simulink model "cubli_XYZ_extensive_simulations"  (R2016a)
settings: Solver=VariableStepAuto  StartTime=0.0  StopTime=10  FixedStep=0.001  RelTol=1e-3
values from neighbouring files (symbols this model uses):
  a = 0.15    [init.m]
  M = 2.5    [init.m]    (also in skew.m = [0 -z y)
  m = 0.204    [init.m]
  s = size(delta_i)    [accessibility_test.m]    (also in observability_test.m = size(delta_i,1))
  state0 = get_equilibrium(0, -pi/4, pi/2, f, state)    [init.m]
undefined symbols (not defined in the file or in its folder): X, Y, Z
libraries: sm_lib x15, nesl_utility x13
(part 3 of 9)

== matlab function cubli_XYZ_extensive_simulations/Cubli/Reference/Slerp ==
  data: R0 input; Rf input; t input; theta_des output; theta input; dtheta_des output; ddtheta_des output
function [theta_des, dtheta_des, ddtheta_des]    = slerp(R0, Rf, t, theta)

% persistent counter th0 thf R0 Rf

% if isempty(counter)
%     counter = 0;
%     R0 = rotx(state0(1))*roty(state0(2))*rotz(state0(3));
%     Rf = rotz(theta) * R0;
%     th0 = [state0(1);state0(2);state0(3)];
%     th21 = atan2(Rf(1,3), sqrt(Rf(2,3)^2 + Rf(3,3)^2));
%     thf = [atan2(-Rf(2,3) / cos(th21), Rf(3,3) / cos(th21));
%            th21;
%            atan2(-Rf(1,2) / cos(th21), Rf(1,1) / cos(th21))];
% end
% t = time/tf;
% 
% if time >= tf
%     t = 1;
% end

% t = time - tf * counter;
% t = time / tf - counter;
% if t > 1
%     counter = counter + 1;
%     t = time/tf - counter;
%     tmp = thf;
%     thf = th0;
%     th0 = tmp;
%     tmp = Rf;
%     Rf = R0;
%     R0 = tmp;
% 
% end

% traj_5_const = 6.0;
% traj_4_const = -15.0;
% traj_3_const = 10.0;
% 
% theta_des = zeros(3,1);
% dtheta_des = zeros(3,1);
% ddtheta_des = zeros(3,1);

% for i = 1:3
%     traj_0_coeff = th0(i);
%     traj_3_coeff = traj_3_const / (tf ^3) * (thf(i) - th0(i));
%     traj_4_coeff = traj_4_const / (tf ^4) * (thf(i) - th0(i));
%     traj_5_coeff = traj_5_const / (tf ^5) * (thf(i) - th0(i));
%     theta_des(i) = traj_5_coeff * t^5 + traj_4_coeff * t^4 + traj_3_coeff * t^3 + traj_0_coeff;
%     dtheta_des(i) = 5 * traj_5_coeff * t^4 + 4 * traj_4_coeff * t^3 + 3 * traj_3_coeff * t^2;
%     ddtheta_des(i) = 5 * 4 * traj_5_coeff * t^3 + 4 * 3 * traj_4_coeff * t^2 + 3 * 2 * traj_3_coeff * t;
% end

q0 = rotm2quat(R0);
q1 = rotm2quat(Rf);

q01 = q0(1);
q02 = q0(2);
q03 = q0(3);
q04 = q0(4);

q11 = q1(1);
q12 = q1(2);
q13 = q1(3);
q14 = q1(4);

th1_des = atan2(2.*csc((1/2).*theta).^2.*((q01.*q02+(-1).* ...
  q03.*q04).*sin((1/2).*(1+(-1).*t).*theta).^2+(q02.*q11+q01.*q12+(-1).* ...
  q04.*q13+(-1).*q03.*q14).*sin((1/2).*(1+(-1).*t).*theta).*sin((1/2).*t.* ...
  theta)+(q11.*q12+(-1).*q13.*q14).*sin((1/2).*t.*theta).^2).*(4.*csc(( ...
  1/2).*theta).^4.*(((-1).*q01.*q02+q03.*q04).*sin((1/2).*(1+(-1).*t).* ...
  theta).^2+(-1).*(q02.*q11+q01.*q12+(-1).*q04.*q13+(-1).*q03.*q14).*sin(( ...
  1/2).*(1+(-1).*t).*theta).*sin((1/2).*t.*theta)+((-1).*q11.*q12+q13.* ...
  q14).*sin((1/2).*t.*theta).^2).^2+(1+(-2).*csc((1/2).*theta).^2.*((q02.* ...
  sin((1/2).*(1+(-1).*t).*theta)+q12.*sin((1/2).*t.*theta)).^2+(q03.*sin(( ...
  1/2).*(1+(-1).*t).*theta)+q13.*sin((1/2).*t.*theta)).^2)).^2).^(-1/2).*( ...
  4.*csc((1/2).*theta).^4.*((q01.*q03+q02.*q04).*sin((1/2).*(1+(-1).*t).* ...
  theta).^2+(q03.*q11+q04.*q12+q01.*q13+q02.*q14).*sin((1/2).*(1+(-1).*t) ...
  .*theta).*sin((1/2).*t.*theta)+(q11.*q13+q12.*q14).*sin((1/2).*t.*theta) ...
  .^2).^2+4.*csc((1/2).*theta).^4.*(((-1).*q01.*q02+q03.*q04).*sin((1/2).* ...
  (1+(-1).*t).*theta).^2+(-1).*(q02.*q11+q01.*q12+(-1).*q04.*q13+(-1).* ...
  q03.*q14).*sin((1/2).*(1+(-1).*t).*theta).*sin((1/2).*t.*theta)+((-1).* ...
  q11.*q12+q13.*q14).*sin((1/2).*t.*theta).^2).^2+(1+(-2).*csc((1/2).* ...
  theta).^2.*((q02.*sin((1/2).*(1+(-1).*t).*theta)+q12.*sin((1/2).*t.* ...
  theta)).^2+(q03.*sin((1/2).*(1+(-1).*t).*theta)+q13.*sin((1/2).*t.* ...
  theta)).^2)).^2).^(1/2),...
  (1+(-2).*csc((1/2).*theta).^2.*((q02.^2+q03.^2).*sin((1/2).*(1+(-1) ...
  .*t).*theta).^2+2.*(q02.*q12+q03.*q13).*sin((1/2).*(1+(-1).*t).*theta).* ...
  sin((1/2).*t.*theta)+(q12.^2+q13.^2).*sin((1/2).*t.*theta).^2)).*(4.* ...
  csc((1/2).*theta).^4.*(((-1).*q01.*q02+q03.*q04).*sin((1/2).*(1+(-1).*t) ...
  .*theta).^2+(-1).*(q02.*q11+q01.*q12+(-1).*q04.*q13+(-1).*q03.*q14).* ...
  sin((1/2).*(1+(-1).*t).*theta).*sin((1/2).*t.*theta)+((-1).*q11.*q12+ ...
  q13.*q14).*sin((1/2).*t.*theta).^2).^2+(1+(-2).*csc((1/2).*theta).^2.*(( ...
  q02.*sin((1/2).*(1+(-1).*t).*theta)+q12.*sin((1/2).*t.*theta)).^2+(q03.* ...
  sin((1/2).*(1+(-1).*t).*theta)+q13.*sin((1/2).*t.*theta)).^2)).^2).^( ...
  -1/2).*(4.*csc((1/2).*theta).^4.*((q01.*q03+q02.*q04).*sin((1/2).*(1+( ...
  -1).*t).*theta).^2+(q03.*q11+q04.*q12+q01.*q13+q02.*q14).*sin((1/2).*(1+ ...
  (-1).*t).*theta).*sin((1/2).*t.*theta)+(q11.*q13+q12.*q14).*sin((1/2).* ...
  t.*theta).^2).^2+4.*csc((1/2).*theta).^4.*(((-1).*q01.*q02+q03.*q04).* ...
  sin((1/2).*(1+(-1).*t).*theta).^2+(-1).*(q02.*q11+q01.*q12+(-1).*q04.* ...
  q13+(-1).*q03.*q14).*sin((1/2).*(1+(-1).*t).*theta).*sin((1/2).*t.* ...
  theta)+((-1).*q11.*q12+q13.*q14).*sin((1/2).*t.*theta).^2).^2+(1+(-2).* ...
  csc((1/2).*theta).^2.*((q02.*sin((1/2).*(1+(-1).*t).*theta)+q12.*sin(( ...
  1/2).*t.*theta)).^2+(q03.*sin((1/2).*(1+(-1).*t).*theta)+q13.*sin((1/2) ...
  .*t.*theta)).^2)).^2).^(1/2));

th2_des = atan2(2.*csc((1/2).*theta).^2.*((q01.*q03+q02.*q04).* ...
  sin((1/2).*(1+(-1).*t).*theta).^2+(q03.*q11+q04.*q12+q01.*q13+q02.*q14) ...
  .*sin((1/2).*(1+(-1).*t).*theta).*sin((1/2).*t.*theta)+(q11.*q13+q12.* ...
  q14).*sin((1/2).*t.*theta).^2),...
 (4.*csc((1/2).*theta).^4.*(((-1).*q01.*q02+q03.*q04).*sin((1/2).*( ...
  1+(-1).*t).*theta).^2+(-1).*(q02.*q11+q01.*q12+(-1).*q04.*q13+(-1).* ...
  q03.*q14).*sin((1/2).*(1+(-1).*t).*theta).*sin((1/2).*t.*theta)+((-1).* ...
  q11.*q12+q13.*q14).*sin((1/2).*t.*theta).^2).^2+(1+(-2).*csc((1/2).* ...
  theta).^2.*((q02.*sin((1/2).*(1+(-1).*t).*theta)+q12.*sin((1/2).*t.* ...
  theta)).^2+(q03.*sin((1/2).*(1+(-1).*t).*theta)+q13.*sin((1/2).*t.* ...
  theta)).^2)).^2).^(1/2));

th3_des = atan2((-2).*csc((1/2).*theta).^2.*((q02.*q03+(-1) ...
  .*q01.*q04).*sin((1/2).*(1+(-1).*t).*theta).^2+(-1).*(q04.*q11+(-1).* ...
  q03.*q12+(-1).*q02.*q13+q01.*q14).*sin((1/2).*(1+(-1).*t).*theta).*sin(( ...
  1/2).*t.*theta)+(q12.*q13+(-1).*q11.*q14).*sin((1/2).*t.*theta).^2).*( ...
  4.*csc((1/2).*theta).^4.*(((-1).*q01.*q02+q03.*q04).*sin((1/2).*(1+(-1) ...
  .*t).*theta).^2+(-1).*(q02.*q11+q01.*q12+(-1).*q04.*q13+(-1).*q03.*q14) ...
  .*sin((1/2).*(1+(-1).*t).*theta).*sin((1/2).*t.*theta)+((-1).*q11.*q12+ ...
  q13.*q14).*sin((1/2).*t.*theta).^2).^2+(1+(-2).*csc((1/2).*theta).^2.*(( ...
  q02.*sin((1/2).*(1+(-1).*t).*theta)+q12.*sin((1/2).*t.*theta)).^2+(q03.* ...
  sin((1/2).*(1+(-1).*t).*theta)+q13.*sin((1/2).*t.*theta)).^2)).^2).^( ...
  -1/2).*(4.*csc((1/2).*theta).^4.*((q01.*q03+q02.*q04).*sin((1/2).*(1+( ...
  -1).*t).*theta).^2+(q03.*q11+q04.*q12+q01.*q13+q02.*q14).*sin((1/2).*(1+ ...
  (-1).*t).*theta).*sin((1/2).*t.*theta)+(q11.*q13+q12.*q14).*sin((1/2).* ...
  t.*theta).^2).^2+4.*csc((1/2).*theta).^4.*(((-1).*q01.*q02+q03.*q04).* ...
  sin((1/2).*(1+(-1).*t).*theta).^2+(-1).*(q02.*q11+q01.*q12+(-1).*q04.* ...
  q13+(-1).*q03.*q14).*sin((1/2).*(1+(-1).*t).*theta).*sin((1/2).*t.* ...
  theta)+((-1).*q11.*q12+q13.*q14).*sin((1/2).*t.*theta).^2).^2+(1+(-2).* ...
  csc((1/2).*theta).^2.*((q02.*sin((1/2).*(1+(-1).*t).*theta)+q12.*sin(( ...
  1/2).*t.*theta)).^2+(q03.*sin((1/2).*(1+(-1).*t).*theta)+q13.*sin((1/2) ...
  .*t.*theta)).^2)).^2).^(1/2),...
  (1+(-2).*csc((1/2).*theta).^2.*((q03.^2+q04.^2).*sin((1/2).*(1+(-1) ...
  .*t).*theta).^2+2.*(q03.*q13+q04.*q14).*sin((1/2).*(1+(-1).*t).*theta).* ...
  sin((1/2).*t.*theta)+(q13.^2+q14.^2).*sin((1/2).*t.*theta).^2)).*(4.* ...
  csc((1/2).*theta).^4.*(((-1).*q01.*q02+q03.*q04).*sin((1/2).*(1+(-1).*t) ...
  .*theta).^2+(-1).*(q02.*q11+q01.*q12+(-1).*q04.*q13+(-1).*q03.*q14).* ...
  sin((1/2).*(1+(-1).*t).*theta).*sin((1/2).*t.*theta)+((-1).*q11.*q12+ ...
  q13.*q14).*sin((1/2).*t.*theta).^2).^2+(1+(-2).*csc((1/2).*theta).^2.*(( ...
  q02.*sin((1/2).*(1+(-1).*t).*theta)+q12.*sin((1/2).*t.*theta)).^2+(q03.* ...
  sin((1/2).*(1+(-1).*t).*theta)+q13.*sin((1/2).*t.*theta)).^2)).^2).^( ...
  -1/2).*(4.*csc((1/2).*theta).^4.*((q01.*q03+q02.*q04).*sin((1/2).*(1+( ...
  -1).*t).*theta).^2+(q03.*q11+q04.*q12+q01.*q13+q02.*q14).*sin((1/2).*(1+ ...
  (-1).*t).*theta).*sin((1/2).*t.*theta)+(q11.*q13+q12.*q14).*sin((1/2).* ...
  t.*theta).^2).^2+4.*csc((1/2).*theta).^4.*(((-1).*q01.*q02+q03.*q04).* ...
  sin((1/2).*(1+(-1).*t).*theta).^2+(-1).*(q02.*q11+q01.*q12+(-1).*q04.* ...
  q13+(-1).*q03.*q14).*sin((1/2).*(1+(-1).*t).*theta).*sin((1/2).*t.* ...
  theta)+((-1).*q11.*q12+q13.*q14).*sin((1/2).*t.*theta).^2).^2+(1+(-2).* ...
  csc((1/2).*theta).^2.*((q02.*sin((1/2).*(1+(-1).*t).*theta)+q12.*sin(( ...
  1/2).*t.*theta)).^2+(q03.*sin((1/2).*(1+(-1).*t).*theta)+q13.*sin((1/2) ...
  .*t.*theta)).^2)).^2).^(1/2));

theta_des = [th1_des; th2_des; th3_des];

dth1_des = (1/4).*theta.*csc((1/2).*theta).^4.*(1+(-4).*csc((1/2).*theta).^2.*(( ...
  q02.^2+q03.^2).*sin((1/2).*(1+(-1).*t).*theta).^2+2.*(q02.*q12+q03.*q13) ...
  .*sin((1/2).*(1+(-1).*t).*theta).*sin((1/2).*t.*theta)+(q12.^2+q13.^2).* ...
  sin((1/2).*t.*theta).^2)+4.*csc((1/2).*theta).^4.*((q01.^2.*q02.^2+ ...
  q02.^4+2.*q02.^2.*q03.^2+q03.^4+(-2).*q01.*q02.*q03.*q04+q03.^2.*q04.^2) ...
  .*sin((1/2).*(1+(-1).*t).*theta).^4+2.*(q01.^2.*q02.*q12+2.*q02.^3.*q12+ ...
  q02.*q03.*((-1).*q04.*q11+2.*q03.*q12)+2.*q02.^2.*q03.*q13+q03.*(2.* ...
  q03.^2.*q13+q04.^2.*q13+q03.*q04.*q14)+q01.*(q02.^2.*q11+(-1).*q03.* ...
  q04.*q12+(-1).*q02.*(q04.*q13+q03.*q14))).*sin((1/2).*(1+(-1).*t).* ...
  theta).^3.*sin((1/2).*t.*theta)+((q01.*q12+(-1).*q04.*q13).^2+q02.^2.*( ...
  q11.^2+6.*q12.^2+2.*q13.^2)+q02.*(4.*q01.*q11.*q12+(-2).*q04.*q11.*q13+ ...
  8.*q03.*q12.*q13+(-2).*q03.*q11.*q14+(-2).*q01.*q13.*q14)+(-2).*q03.*( ...
  q04.*q11.*q12+q01.*q12.*q14+(-2).*q04.*q13.*q14)+q03.^2.*(2.*q12.^2+6.* ...
  q13.^2+q14.^2)).*sin((1/2).*(1+(-1).*t).*theta).^2.*sin((1/2).*t.*theta) ...
  .^2+2.*((-1).*q04.*q11.*q12.*q13+2.*q03.*q12.^2.*q13+2.*q03.*q13.^3+(-1) ...
  .*q03.*q11.*q12.*q14+q04.*q13.^2.*q14+q03.*q13.*q14.^2+q01.*q12.*(q11.* ...
  q12+(-1).*q13.*q14)+q02.*(q11.^2.*q12+2.*q12.*(q12.^2+q13.^2)+(-1).* ...
  q11.*q13.*q14)).*sin((1/2).*(1+(-1).*t).*theta).*sin((1/2).*t.*theta) ...
  .^3+(q11.^2.*q12.^2+q12.^4+2.*q12.^2.*q13.^2+q13.^4+(-2).*q11.*q12.* ...
  q13.*q14+q13.^2.*q14.^2).*sin((1/2).*t.*theta).^4)).^(-1).*((-4).*( ...
  q02.^3.*q11+q03.^2.*q04.*q13+2.*q03.*q11.*q12.*q13+q04.*q12.^2.*q13+ ...
  q04.*q13.^3+(-1).*q01.*q12.*((-1).*q03.^2+q12.^2+q13.^2)+(-1).*q03.^3.* ...
  q14+q03.*q12.^2.*q14+(-1).*q03.*q13.^2.*q14+(-1).*q02.^2.*(q01.*q12+ ...
  q04.*q13+q03.*q14)+q02.*(q03.^2.*q11+2.*q03.*q04.*q12+q11.*q12.^2+(-2).* ...
  q01.*q03.*q13+(-1).*q11.*q13.^2+(-2).*q12.*q13.*q14)).*sin((1/2).*theta) ...
  +4.*((-1).*q01.*q02.*(q12.^2+q13.^2)+q02.^2.*(q11.*q12+(-1).*q13.*q14)+ ...
  q03.*(q04.*(q12.^2+q13.^2)+q03.*(q11.*q12+(-1).*q13.*q14))).*sin(theta)+ ...
  (-1).*q02.*q11.*sin(((3/2)+(-1).*t).*theta)+2.*q02.^3.*q11.*sin(((3/2)+( ...
  -1).*t).*theta)+2.*q02.*q03.^2.*q11.*sin(((3/2)+(-1).*t).*theta)+(-1).* ...
  q01.*q12.*sin(((3/2)+(-1).*t).*theta)+(-2).*q01.*q02.^2.*q12.*sin(((3/2) ...
  +(-1).*t).*theta)+2.*q01.*q03.^2.*q12.*sin(((3/2)+(-1).*t).*theta)+4.* ...
  q02.*q03.*q04.*q12.*sin(((3/2)+(-1).*t).*theta)+(-4).*q01.*q02.*q03.* ...
  q13.*sin(((3/2)+(-1).*t).*theta)+q04.*q13.*sin(((3/2)+(-1).*t).*theta)+( ...
  -2).*q02.^2.*q04.*q13.*sin(((3/2)+(-1).*t).*theta)+2.*q03.^2.*q04.*q13.* ...
  sin(((3/2)+(-1).*t).*theta)+q03.*q14.*sin(((3/2)+(-1).*t).*theta)+(-2).* ...
  q02.^2.*q03.*q14.*sin(((3/2)+(-1).*t).*theta)+(-2).*q03.^3.*q14.*sin((( ...
  3/2)+(-1).*t).*theta)+(-1).*q01.*q02.*sin(((-2)+t).*theta)+q03.*q04.* ...
  sin(((-2)+t).*theta)+(-1).*q01.*q02.*sin(t.*theta)+q03.*q04.*sin(t.* ...
  theta)+2.*q11.*q12.*sin(t.*theta)+(-4).*q02.^2.*q11.*q12.*sin(t.*theta)+ ...
  (-4).*q03.^2.*q11.*q12.*sin(t.*theta)+4.*q01.*q02.*q12.^2.*sin(t.*theta) ...
  +(-4).*q03.*q04.*q12.^2.*sin(t.*theta)+4.*q01.*q02.*q13.^2.*sin(t.* ...
  theta)+(-4).*q03.*q04.*q13.^2.*sin(t.*theta)+(-2).*q13.*q14.*sin(t.* ...
  theta)+4.*q02.^2.*q13.*q14.*sin(t.*theta)+4.*q03.^2.*q13.*q14.*sin(t.* ...
  theta)+q02.*q11.*sin(((1/2)+t).*theta)+q01.*q12.*sin(((1/2)+t).*theta)+ ...
  2.*q02.*q11.*q12.^2.*sin(((1/2)+t).*theta)+(-2).*q01.*q12.^3.*sin(((1/2) ...
  +t).*theta)+(-1).*q04.*q13.*sin(((1/2)+t).*theta)+4.*q03.*q11.*q12.* ...
  q13.*sin(((1/2)+t).*theta)+2.*q04.*q12.^2.*q13.*sin(((1/2)+t).*theta)+( ...
  -2).*q02.*q11.*q13.^2.*sin(((1/2)+t).*theta)+(-2).*q01.*q12.*q13.^2.* ...
  sin(((1/2)+t).*theta)+2.*q04.*q13.^3.*sin(((1/2)+t).*theta)+(-1).*q03.* ...
  q14.*sin(((1/2)+t).*theta)+2.*q03.*q12.^2.*q14.*sin(((1/2)+t).*theta)+( ...
  -4).*q02.*q12.*q13.*q14.*sin(((1/2)+t).*theta)+(-2).*q03.*q13.^2.*q14.* ...
  sin(((1/2)+t).*theta)+(-1).*q11.*q12.*sin((1+t).*theta)+q13.*q14.*sin(( ...
  1+t).*theta)+2.*q02.*q11.*sin((1/2).*(theta+(-2).*t.*theta))+(-2).* ...
  q02.^3.*q11.*sin((1/2).*(theta+(-2).*t.*theta))+(-2).*q02.*q03.^2.*q11.* ...
  sin((1/2).*(theta+(-2).*t.*theta))+2.*q01.*q12.*sin((1/2).*(theta+(-2).* ...
  t.*theta))+2.*q01.*q02.^2.*q12.*sin((1/2).*(theta+(-2).*t.*theta))+(-2) ...
  .*q01.*q03.^2.*q12.*sin((1/2).*(theta+(-2).*t.*theta))+(-4).*q02.*q03.* ...
  q04.*q12.*sin((1/2).*(theta+(-2).*t.*theta))+2.*q02.*q11.*q12.^2.*sin(( ...
  1/2).*(theta+(-2).*t.*theta))+(-2).*q01.*q12.^3.*sin((1/2).*(theta+(-2) ...
  .*t.*theta))+4.*q01.*q02.*q03.*q13.*sin((1/2).*(theta+(-2).*t.*theta))+( ...
  -2).*q04.*q13.*sin((1/2).*(theta+(-2).*t.*theta))+2.*q02.^2.*q04.*q13.* ...
  sin((1/2).*(theta+(-2).*t.*theta))+(-2).*q03.^2.*q04.*q13.*sin((1/2).*( ...
  theta+(-2).*t.*theta))+4.*q03.*q11.*q12.*q13.*sin((1/2).*(theta+(-2).* ...
  t.*theta))+2.*q04.*q12.^2.*q13.*sin((1/2).*(theta+(-2).*t.*theta))+(-2) ...
  .*q02.*q11.*q13.^2.*sin((1/2).*(theta+(-2).*t.*theta))+(-2).*q01.*q12.* ...
  q13.^2.*sin((1/2).*(theta+(-2).*t.*theta))+2.*q04.*q13.^3.*sin((1/2).*( ...
  theta+(-2).*t.*theta))+(-2).*q03.*q14.*sin((1/2).*(theta+(-2).*t.*theta) ...
  )+2.*q02.^2.*q03.*q14.*sin((1/2).*(theta+(-2).*t.*theta))+2.*q03.^3.* ...
  q14.*sin((1/2).*(theta+(-2).*t.*theta))+2.*q03.*q12.^2.*q14.*sin((1/2).* ...
  (theta+(-2).*t.*theta))+(-4).*q02.*q12.*q13.*q14.*sin((1/2).*(theta+(-2) ...
  .*t.*theta))+(-2).*q03.*q13.^2.*q14.*sin((1/2).*(theta+(-2).*t.*theta))+ ...
  (-2).*q01.*q02.*sin(theta+(-1).*t.*theta)+2.*q03.*q04.*sin(theta+(-1).* ...
  t.*theta)+q11.*q12.*sin(theta+(-1).*t.*theta)+(-4).*q02.^2.*q11.*q12.* ...
  sin(theta+(-1).*t.*theta)+(-4).*q03.^2.*q11.*q12.*sin(theta+(-1).*t.* ...
  theta)+4.*q01.*q02.*q12.^2.*sin(theta+(-1).*t.*theta)+(-4).*q03.*q04.* ...
  q12.^2.*sin(theta+(-1).*t.*theta)+4.*q01.*q02.*q13.^2.*sin(theta+(-1).* ...
  t.*theta)+(-4).*q03.*q04.*q13.^2.*sin(theta+(-1).*t.*theta)+(-1).*q13.* ...
  q14.*sin(theta+(-1).*t.*theta)+4.*q02.^2.*q13.*q14.*sin(theta+(-1).*t.* ...
  theta)+4.*q03.^2.*q13.*q14.*sin(theta+(-1).*t.*theta));

dth2_des = csc((1/2).*theta).^2.*(4.*csc((1/2).*theta).^4.*(((-1).*q01.*q02+q03.* ...
  q04).*sin((1/2).*(1+(-1).*t).*theta).^2+(-1).*(q02.*q11+q01.*q12+(-1).* ...
  q04.*q13+(-1).*q03.*q14).*sin((1/2).*(1+(-1).*t).*theta).*sin((1/2).*t.* ...
  theta)+((-1).*q11.*q12+q13.*q14).*sin((1/2).*t.*theta).^2).^2+(1+(-2).* ...
  csc((1/2).*theta).^2.*((q02.*sin((1/2).*(1+(-1).*t).*theta)+q12.*sin(( ...
  1/2).*t.*theta)).^2+(q03.*sin((1/2).*(1+(-1).*t).*theta)+q13.*sin((1/2) ...
  .*t.*theta)).^2)).^2).^(-1/2).*(4.*csc((1/2).*theta).^4.*((q01.*q03+ ...
  q02.*q04).*sin((1/2).*(1+(-1).*t).*theta).^2+(q03.*q11+q04.*q12+q01.* ...
  q13+q02.*q14).*sin((1/2).*(1+(-1).*t).*theta).*sin((1/2).*t.*theta)+( ...
  q11.*q13+q12.*q14).*sin((1/2).*t.*theta).^2).^2+4.*csc((1/2).*theta) ...
  .^4.*(((-1).*q01.*q02+q03.*q04).*sin((1/2).*(1+(-1).*t).*theta).^2+(-1) ...
  .*(q02.*q11+q01.*q12+(-1).*q04.*q13+(-1).*q03.*q14).*sin((1/2).*(1+(-1) ...
  .*t).*theta).*sin((1/2).*t.*theta)+((-1).*q11.*q12+q13.*q14).*sin((1/2) ...
  .*t.*theta).^2).^2+(1+(-2).*csc((1/2).*theta).^2.*((q02.*sin((1/2).*(1+( ...
  -1).*t).*theta)+q12.*sin((1/2).*t.*theta)).^2+(q03.*sin((1/2).*(1+(-1).* ...
  t).*theta)+q13.*sin((1/2).*t.*theta)).^2)).^2).^(-1).*((1/2).*theta.*( ...
  4.*csc((1/2).*theta).^4.*(((-1).*q01.*q02+q03.*q04).*sin((1/2).*(1+(-1) ...
  .*t).*theta).^2+(-1).*(q02.*q11+q01.*q12+(-1).*q04.*q13+(-1).*q03.*q14) ...
  .*sin((1/2).*(1+(-1).*t).*theta).*sin((1/2).*t.*theta)+((-1).*q11.*q12+ ...
  q13.*q14).*sin((1/2).*t.*theta).^2).^2+(1+(-2).*csc((1/2).*theta).^2.*(( ...
  q02.*sin((1/2).*(1+(-1).*t).*theta)+q12.*sin((1/2).*t.*theta)).^2+(q03.* ...
  sin((1/2).*(1+(-1).*t).*theta)+q13.*sin((1/2).*t.*theta)).^2)).^2).*(2.* ...
  (q03.*q11+q04.*q12+q01.*q13+q02.*q14).*cos((1/2).*t.*theta).*sin((1/2).* ...
  (1+(-1).*t).*theta)+(-2).*(q03.*q11+q04.*q12+q01.*q13+q02.*q14).*cos(( ...
  1/2).*((-1)+t).*theta).*sin((1/2).*t.*theta)+2.*(q11.*q13+q12.*q14).* ...
  sin(t.*theta)+(-2).*(q01.*q03+q02.*q04).*sin(theta+(-1).*t.*theta))+(-1) ...
  .*((q01.*q03+q02.*q04).*sin((1/2).*(1+(-1).*t).*theta).^2+(q03.*q11+ ...
  q04.*q12+q01.*q13+q02.*q14).*sin((1/2).*(1+(-1).*t).*theta).*sin((1/2).* ...
  t.*theta)+(q11.*q13+q12.*q14).*sin((1/2).*t.*theta).^2).*((-2).*theta.* ...
  csc((1/2).*theta).^2.*(1+(-2).*csc((1/2).*theta).^2.*((q02.*sin((1/2).*( ...
  1+(-1).*t).*theta)+q12.*sin((1/2).*t.*theta)).^2+(q03.*sin((1/2).*(1+( ...
  -1).*t).*theta)+q13.*sin((1/2).*t.*theta)).^2)).*((q12.^2+q13.^2).*sin( ...
  t.*theta)+2.*(q02.*q12+q03.*q13).*sin((1/2).*(theta+(-2).*t.*theta))+( ...
  -1).*(q02.^2+q03.^2).*sin(theta+(-1).*t.*theta))+(-4).*theta.*csc((1/2) ...
  .*theta).^4.*(((-1).*q01.*q02+q03.*q04).*sin((1/2).*(1+(-1).*t).*theta) ...
  .^2+(-1).*(q02.*q11+q01.*q12+(-1).*q04.*q13+(-1).*q03.*q14).*sin((1/2).* ...
  (1+(-1).*t).*theta).*sin((1/2).*t.*theta)+((-1).*q11.*q12+q13.*q14).* ...
  sin((1/2).*t.*theta).^2).*((q11.*q12+(-1).*q13.*q14).*sin(t.*theta)+( ...
  q02.*q11+q01.*q12+(-1).*q04.*q13+(-1).*q03.*q14).*sin((1/2).*(theta+(-2) ...
  .*t.*theta))+((-1).*q01.*q02+q03.*q04).*sin(theta+(-1).*t.*theta))));

dth3_des = (-1/4).*theta.*csc((1/2).*theta).^4.*(1+(-4).*csc((1/2).*theta).^2.*(( ...
  q03.^2+q04.^2).*sin((1/2).*(1+(-1).*t).*theta).^2+2.*(q03.*q13+q04.*q14) ...
  .*sin((1/2).*(1+(-1).*t).*theta).*sin((1/2).*t.*theta)+(q13.^2+q14.^2).* ...
  sin((1/2).*t.*theta).^2)+4.*csc((1/2).*theta).^4.*((q02.^2.*q03.^2+ ...
  q03.^4+(-2).*q01.*q02.*q03.*q04+q01.^2.*q04.^2+2.*q03.^2.*q04.^2+q04.^4) ...
  .*sin((1/2).*(1+(-1).*t).*theta).^4+2.*(q01.*q04.*(q04.*q11+(-1).*q03.* ...
  q12)+q02.^2.*q03.*q13+q01.^2.*q04.*q14+2.*(q03.^2+q04.^2).*(q03.*q13+ ...
  q04.*q14)+q02.*(q03.^2.*q12+(-1).*q01.*q04.*q13+(-1).*q03.*(q04.*q11+ ...
  q01.*q14))).*sin((1/2).*(1+(-1).*t).*theta).^3.*sin((1/2).*t.*theta)+(( ...
  q02.*q13+(-1).*q01.*q14).^2+(-2).*q03.*((-2).*q02.*q12.*q13+q02.*q11.* ...
  q14+q01.*q12.*q14)+(-2).*q04.*(q03.*q11.*q12+q02.*q11.*q13+q01.*q12.* ...
  q13+(-2).*q01.*q11.*q14+(-4).*q03.*q13.*q14)+q03.^2.*(q12.^2+6.*q13.^2+ ...
  2.*q14.^2)+q04.^2.*(q11.^2+2.*q13.^2+6.*q14.^2)).*sin((1/2).*(1+(-1).*t) ...
  .*theta).^2.*sin((1/2).*t.*theta).^2+2.*((q02.*q13+(-1).*q01.*q14).*( ...
  q12.*q13+(-1).*q11.*q14)+q03.*(q12.^2.*q13+(-1).*q11.*q12.*q14+2.*q13.*( ...
  q13.^2+q14.^2))+q04.*((-1).*q11.*q12.*q13+q11.^2.*q14+2.*q14.*(q13.^2+ ...
  q14.^2))).*sin((1/2).*(1+(-1).*t).*theta).*sin((1/2).*t.*theta).^3+( ...
  q12.^2.*q13.^2+q13.^4+(-2).*q11.*q12.*q13.*q14+q11.^2.*q14.^2+2.* ...
  q13.^2.*q14.^2+q14.^4).*sin((1/2).*t.*theta).^4)).^(-1).*((-4).*((-1).* ...
  q04.^3.*q11+q03.^3.*q12+q04.^2.*(q02.*q13+q01.*q14)+(-1).*q03.^2.*(q04.* ...
  q11+q02.*q13+q01.*q14)+(-1).*(q02.*q13+(-1).*q01.*q14).*(q13.^2+q14.^2)+ ...
  q04.*(q11.*q13.^2+2.*q12.*q13.*q14+(-1).*q11.*q14.^2)+q03.*(q04.^2.*q12+ ...
  2.*q01.*q04.*q13+q12.*q13.^2+(-2).*q02.*q04.*q14+(-2).*q11.*q13.*q14+( ...
  -1).*q12.*q14.^2)).*sin((1/2).*theta)+4.*(q03.^2.*(q12.*q13+(-1).*q11.* ...
  q14)+(-1).*q02.*q03.*(q13.^2+q14.^2)+q04.*(q04.*(q12.*q13+(-1).*q11.* ...
  q14)+q01.*(q13.^2+q14.^2))).*sin(theta)+q04.*q11.*sin(((3/2)+(-1).*t).* ...
  theta)+(-2).*q03.^2.*q04.*q11.*sin(((3/2)+(-1).*t).*theta)+(-2).* ...
  q04.^3.*q11.*sin(((3/2)+(-1).*t).*theta)+(-1).*q03.*q12.*sin(((3/2)+(-1) ...
  .*t).*theta)+2.*q03.^3.*q12.*sin(((3/2)+(-1).*t).*theta)+2.*q03.* ...
  q04.^2.*q12.*sin(((3/2)+(-1).*t).*theta)+(-1).*q02.*q13.*sin(((3/2)+(-1) ...
  .*t).*theta)+(-2).*q02.*q03.^2.*q13.*sin(((3/2)+(-1).*t).*theta)+4.* ...
  q01.*q03.*q04.*q13.*sin(((3/2)+(-1).*t).*theta)+2.*q02.*q04.^2.*q13.* ...
  sin(((3/2)+(-1).*t).*theta)+q01.*q14.*sin(((3/2)+(-1).*t).*theta)+(-2).* ...
  q01.*q03.^2.*q14.*sin(((3/2)+(-1).*t).*theta)+(-4).*q02.*q03.*q04.*q14.* ...
  sin(((3/2)+(-1).*t).*theta)+2.*q01.*q04.^2.*q14.*sin(((3/2)+(-1).*t).* ...
  theta)+(-1).*q02.*q03.*sin(((-2)+t).*theta)+q01.*q04.*sin(((-2)+t).* ...
  theta)+(-1).*q02.*q03.*sin(t.*theta)+q01.*q04.*sin(t.*theta)+2.*q12.* ...
  q13.*sin(t.*theta)+(-4).*q03.^2.*q12.*q13.*sin(t.*theta)+(-4).*q04.^2.* ...
  q12.*q13.*sin(t.*theta)+4.*q02.*q03.*q13.^2.*sin(t.*theta)+(-4).*q01.* ...
  q04.*q13.^2.*sin(t.*theta)+(-2).*q11.*q14.*sin(t.*theta)+4.*q03.^2.* ...
  q11.*q14.*sin(t.*theta)+4.*q04.^2.*q11.*q14.*sin(t.*theta)+4.*q02.*q03.* ...
  q14.^2.*sin(t.*theta)+(-4).*q01.*q04.*q14.^2.*sin(t.*theta)+(-1).*q04.* ...
  q11.*sin(((1/2)+t).*theta)+q03.*q12.*sin(((1/2)+t).*theta)+q02.*q13.* ...
  sin(((1/2)+t).*theta)+2.*q04.*q11.*q13.^2.*sin(((1/2)+t).*theta)+2.* ...
  q03.*q12.*q13.^2.*sin(((1/2)+t).*theta)+(-2).*q02.*q13.^3.*sin(((1/2)+t) ...
  .*theta)+(-1).*q01.*q14.*sin(((1/2)+t).*theta)+(-4).*q03.*q11.*q13.* ...
  q14.*sin(((1/2)+t).*theta)+4.*q04.*q12.*q13.*q14.*sin(((1/2)+t).*theta)+ ...
  2.*q01.*q13.^2.*q14.*sin(((1/2)+t).*theta)+(-2).*q04.*q11.*q14.^2.*sin(( ...
  (1/2)+t).*theta)+(-2).*q03.*q12.*q14.^2.*sin(((1/2)+t).*theta)+(-2).* ...
  q02.*q13.*q14.^2.*sin(((1/2)+t).*theta)+2.*q01.*q14.^3.*sin(((1/2)+t).* ...
  theta)+(-1).*q12.*q13.*sin((1+t).*theta)+q11.*q14.*sin((1+t).*theta)+( ...
  -2).*q04.*q11.*sin((1/2).*(theta+(-2).*t.*theta))+2.*q03.^2.*q04.*q11.* ...
  sin((1/2).*(theta+(-2).*t.*theta))+2.*q04.^3.*q11.*sin((1/2).*(theta+( ...
  -2).*t.*theta))+2.*q03.*q12.*sin((1/2).*(theta+(-2).*t.*theta))+(-2).* ...
  q03.^3.*q12.*sin((1/2).*(theta+(-2).*t.*theta))+(-2).*q03.*q04.^2.*q12.* ...
  sin((1/2).*(theta+(-2).*t.*theta))+2.*q02.*q13.*sin((1/2).*(theta+(-2).* ...
  t.*theta))+2.*q02.*q03.^2.*q13.*sin((1/2).*(theta+(-2).*t.*theta))+(-4) ...
  .*q01.*q03.*q04.*q13.*sin((1/2).*(theta+(-2).*t.*theta))+(-2).*q02.* ...
  q04.^2.*q13.*sin((1/2).*(theta+(-2).*t.*theta))+2.*q04.*q11.*q13.^2.* ...
  sin((1/2).*(theta+(-2).*t.*theta))+2.*q03.*q12.*q13.^2.*sin((1/2).*( ...
  theta+(-2).*t.*theta))+(-2).*q02.*q13.^3.*sin((1/2).*(theta+(-2).*t.* ...
  theta))+(-2).*q01.*q14.*sin((1/2).*(theta+(-2).*t.*theta))+2.*q01.* ...
  q03.^2.*q14.*sin((1/2).*(theta+(-2).*t.*theta))+4.*q02.*q03.*q04.*q14.* ...
  sin((1/2).*(theta+(-2).*t.*theta))+(-2).*q01.*q04.^2.*q14.*sin((1/2).*( ...
  theta+(-2).*t.*theta))+(-4).*q03.*q11.*q13.*q14.*sin((1/2).*(theta+(-2) ...
  .*t.*theta))+4.*q04.*q12.*q13.*q14.*sin((1/2).*(theta+(-2).*t.*theta))+ ...
  2.*q01.*q13.^2.*q14.*sin((1/2).*(theta+(-2).*t.*theta))+(-2).*q04.*q11.* ...
  q14.^2.*sin((1/2).*(theta+(-2).*t.*theta))+(-2).*q03.*q12.*q14.^2.*sin(( ...
  1/2).*(theta+(-2).*t.*theta))+(-2).*q02.*q13.*q14.^2.*sin((1/2).*(theta+ ...
  (-2).*t.*theta))+2.*q01.*q14.^3.*sin((1/2).*(theta+(-2).*t.*theta))+(-2) ...
  .*q02.*q03.*sin(theta+(-1).*t.*theta)+2.*q01.*q04.*sin(theta+(-1).*t.* ...
  theta)+q12.*q13.*sin(theta+(-1).*t.*theta)+(-4).*q03.^2.*q12.*q13.*sin( ...
  theta+(-1).*t.*theta)+(-4).*q04.^2.*q12.*q13.*sin(theta+(-1).*t.*theta)+ ...
  4.*q02.*q03.*q13.^2.*sin(theta+(-1).*t.*theta)+(-4).*q01.*q04.*q13.^2.* ...
  sin(theta+(-1).*t.*theta)+(-1).*q11.*q14.*sin(theta+(-1).*t.*theta)+4.* ...
  q03.^2.*q11.*q14.*sin(theta+(-1).*t.*theta)+4.*q04.^2.*q11.*q14.*sin( ...
  theta+(-1).*t.*theta)+4.*q02.*q03.*q14.^2.*sin(theta+(-1).*t.*theta)+( ...
  -4).*q01.*q04.*q14.^2.*sin(theta+(-1).*t.*theta));

 dtheta_des = [dth1_des; dth2_des; dth3_des];
 
ddth1_des = (1/4).*theta.*(q02.*q11.*theta.*cos(((3/2)+(-1).*t).*theta)+(-2).* ...
  q02.^3.*q11.*theta.*cos(((3/2)+(-1).*t).*theta)+(-2).*q02.*q03.^2.*q11.* ...
  theta.*cos(((3/2)+(-1).*t).*theta)+q01.*q12.*theta.*cos(((3/2)+(-1).*t) ...
  .*theta)+2.*q01.*q02.^2.*q12.*theta.*cos(((3/2)+(-1).*t).*theta)+(-2).* ...
  q01.*q03.^2.*q12.*theta.*cos(((3/2)+(-1).*t).*theta)+(-4).*q02.*q03.* ...
  q04.*q12.*theta.*cos(((3/2)+(-1).*t).*theta)+4.*q01.*q02.*q03.*q13.* ...
  theta.*cos(((3/2)+(-1).*t).*theta)+(-1).*q04.*q13.*theta.*cos(((3/2)+( ...
  -1).*t).*theta)+2.*q02.^2.*q04.*q13.*theta.*cos(((3/2)+(-1).*t).*theta)+ ...
  (-2).*q03.^2.*q04.*q13.*theta.*cos(((3/2)+(-1).*t).*theta)+(-1).*q03.* ...
  q14.*theta.*cos(((3/2)+(-1).*t).*theta)+2.*q02.^2.*q03.*q14.*theta.*cos( ...
  ((3/2)+(-1).*t).*theta)+2.*q03.^3.*q14.*theta.*cos(((3/2)+(-1).*t).* ...
  theta)+(-1).*q01.*q02.*theta.*cos(((-2)+t).*theta)+q03.*q04.*theta.*cos( ...
  ((-2)+t).*theta)+(-1).*q01.*q02.*theta.*cos(t.*theta)+q03.*q04.*theta.* ...
  cos(t.*theta)+2.*q11.*q12.*theta.*cos(t.*theta)+(-4).*q02.^2.*q11.*q12.* ...
  theta.*cos(t.*theta)+(-4).*q03.^2.*q11.*q12.*theta.*cos(t.*theta)+4.* ...
  q01.*q02.*q12.^2.*theta.*cos(t.*theta)+(-4).*q03.*q04.*q12.^2.*theta.* ...
  cos(t.*theta)+4.*q01.*q02.*q13.^2.*theta.*cos(t.*theta)+(-4).*q03.*q04.* ...
  q13.^2.*theta.*cos(t.*theta)+(-2).*q13.*q14.*theta.*cos(t.*theta)+4.* ...
  q02.^2.*q13.*q14.*theta.*cos(t.*theta)+4.*q03.^2.*q13.*q14.*theta.*cos( ...
  t.*theta)+q02.*q11.*theta.*cos(((1/2)+t).*theta)+q01.*q12.*theta.*cos((( ...
  1/2)+t).*theta)+2.*q02.*q11.*q12.^2.*theta.*cos(((1/2)+t).*theta)+(-2).* ...
  q01.*q12.^3.*theta.*cos(((1/2)+t).*theta)+(-1).*q04.*q13.*theta.*cos((( ...
  1/2)+t).*theta)+4.*q03.*q11.*q12.*q13.*theta.*cos(((1/2)+t).*theta)+2.* ...
  q04.*q12.^2.*q13.*theta.*cos(((1/2)+t).*theta)+(-2).*q02.*q11.*q13.^2.* ...
  theta.*cos(((1/2)+t).*theta)+(-2).*q01.*q12.*q13.^2.*theta.*cos(((1/2)+ ...
  t).*theta)+2.*q04.*q13.^3.*theta.*cos(((1/2)+t).*theta)+(-1).*q03.*q14.* ...
  theta.*cos(((1/2)+t).*theta)+2.*q03.*q12.^2.*q14.*theta.*cos(((1/2)+t).* ...
  theta)+(-4).*q02.*q12.*q13.*q14.*theta.*cos(((1/2)+t).*theta)+(-2).* ...
  q03.*q13.^2.*q14.*theta.*cos(((1/2)+t).*theta)+(-1).*q11.*q12.*theta.* ...
  cos((1+t).*theta)+q13.*q14.*theta.*cos((1+t).*theta)+(-2).*q02.*q11.* ...
  theta.*cos((1/2).*(theta+(-2).*t.*theta))+2.*q02.^3.*q11.*theta.*cos(( ...
  1/2).*(theta+(-2).*t.*theta))+2.*q02.*q03.^2.*q11.*theta.*cos((1/2).*( ...
  theta+(-2).*t.*theta))+(-2).*q01.*q12.*theta.*cos((1/2).*(theta+(-2).* ...
  t.*theta))+(-2).*q01.*q02.^2.*q12.*theta.*cos((1/2).*(theta+(-2).*t.* ...
  theta))+2.*q01.*q03.^2.*q12.*theta.*cos((1/2).*(theta+(-2).*t.*theta))+ ...
  4.*q02.*q03.*q04.*q12.*theta.*cos((1/2).*(theta+(-2).*t.*theta))+(-2).* ...
  q02.*q11.*q12.^2.*theta.*cos((1/2).*(theta+(-2).*t.*theta))+2.*q01.* ...
  q12.^3.*theta.*cos((1/2).*(theta+(-2).*t.*theta))+(-4).*q01.*q02.*q03.* ...
  q13.*theta.*cos((1/2).*(theta+(-2).*t.*theta))+2.*q04.*q13.*theta.*cos(( ...
  1/2).*(theta+(-2).*t.*theta))+(-2).*q02.^2.*q04.*q13.*theta.*cos((1/2).* ...
  (theta+(-2).*t.*theta))+2.*q03.^2.*q04.*q13.*theta.*cos((1/2).*(theta+( ...
  -2).*t.*theta))+(-4).*q03.*q11.*q12.*q13.*theta.*cos((1/2).*(theta+(-2) ...
  .*t.*theta))+(-2).*q04.*q12.^2.*q13.*theta.*cos((1/2).*(theta+(-2).*t.* ...
  theta))+2.*q02.*q11.*q13.^2.*theta.*cos((1/2).*(theta+(-2).*t.*theta))+ ...
  2.*q01.*q12.*q13.^2.*theta.*cos((1/2).*(theta+(-2).*t.*theta))+(-2).* ...
  q04.*q13.^3.*theta.*cos((1/2).*(theta+(-2).*t.*theta))+2.*q03.*q14.* ...
  theta.*cos((1/2).*(theta+(-2).*t.*theta))+(-2).*q02.^2.*q03.*q14.* ...
  theta.*cos((1/2).*(theta+(-2).*t.*theta))+(-2).*q03.^3.*q14.*theta.*cos( ...
  (1/2).*(theta+(-2).*t.*theta))+(-2).*q03.*q12.^2.*q14.*theta.*cos((1/2) ...
  .*(theta+(-2).*t.*theta))+4.*q02.*q12.*q13.*q14.*theta.*cos((1/2).*( ...
  theta+(-2).*t.*theta))+2.*q03.*q13.^2.*q14.*theta.*cos((1/2).*(theta+( ...
  -2).*t.*theta))+2.*q01.*q02.*theta.*cos(theta+(-1).*t.*theta)+(-2).* ...
  q03.*q04.*theta.*cos(theta+(-1).*t.*theta)+(-1).*q11.*q12.*theta.*cos( ...
  theta+(-1).*t.*theta)+4.*q02.^2.*q11.*q12.*theta.*cos(theta+(-1).*t.* ...
  theta)+4.*q03.^2.*q11.*q12.*theta.*cos(theta+(-1).*t.*theta)+(-4).*q01.* ...
  q02.*q12.^2.*theta.*cos(theta+(-1).*t.*theta)+4.*q03.*q04.*q12.^2.* ...
  theta.*cos(theta+(-1).*t.*theta)+(-4).*q01.*q02.*q13.^2.*theta.*cos( ...
  theta+(-1).*t.*theta)+4.*q03.*q04.*q13.^2.*theta.*cos(theta+(-1).*t.* ...
  theta)+q13.*q14.*theta.*cos(theta+(-1).*t.*theta)+(-4).*q02.^2.*q13.* ...
  q14.*theta.*cos(theta+(-1).*t.*theta)+(-4).*q03.^2.*q13.*q14.*theta.* ...
  cos(theta+(-1).*t.*theta)).*csc((1/2).*theta).^4.*(1+(-4).*csc((1/2).* ...
  theta).^2.*((q02.^2+q03.^2).*sin((1/2).*(1+(-1).*t).*theta).^2+2.*(q02.* ...
  q12+q03.*q13).*sin((1/2).*(1+(-1).*t).*theta).*sin((1/2).*t.*theta)+( ...
  q12.^2+q13.^2).*sin((1/2).*t.*theta).^2)+4.*csc((1/2).*theta).^4.*(( ...
  q01.^2.*q02.^2+q02.^4+2.*q02.^2.*q03.^2+q03.^4+(-2).*q01.*q02.*q03.*q04+ ...
  q03.^2.*q04.^2).*sin((1/2).*(1+(-1).*t).*theta).^4+2.*(q01.^2.*q02.*q12+ ...
  2.*q02.^3.*q12+q02.*q03.*((-1).*q04.*q11+2.*q03.*q12)+2.*q02.^2.*q03.* ...
  q13+q03.*(2.*q03.^2.*q13+q04.^2.*q13+q03.*q04.*q14)+q01.*(q02.^2.*q11+( ...
  -1).*q03.*q04.*q12+(-1).*q02.*(q04.*q13+q03.*q14))).*sin((1/2).*(1+(-1) ...
  .*t).*theta).^3.*sin((1/2).*t.*theta)+((q01.*q12+(-1).*q04.*q13).^2+ ...
  q02.^2.*(q11.^2+6.*q12.^2+2.*q13.^2)+q02.*(4.*q01.*q11.*q12+(-2).*q04.* ...
  q11.*q13+8.*q03.*q12.*q13+(-2).*q03.*q11.*q14+(-2).*q01.*q13.*q14)+(-2) ...
  .*q03.*(q04.*q11.*q12+q01.*q12.*q14+(-2).*q04.*q13.*q14)+q03.^2.*(2.* ...
  q12.^2+6.*q13.^2+q14.^2)).*sin((1/2).*(1+(-1).*t).*theta).^2.*sin((1/2) ...
  .*t.*theta).^2+2.*((-1).*q04.*q11.*q12.*q13+2.*q03.*q12.^2.*q13+2.*q03.* ...
  q13.^3+(-1).*q03.*q11.*q12.*q14+q04.*q13.^2.*q14+q03.*q13.*q14.^2+q01.* ...
  q12.*(q11.*q12+(-1).*q13.*q14)+q02.*(q11.^2.*q12+2.*q12.*(q12.^2+q13.^2) ...
  +(-1).*q11.*q13.*q14)).*sin((1/2).*(1+(-1).*t).*theta).*sin((1/2).*t.* ...
  theta).^3+(q11.^2.*q12.^2+q12.^4+2.*q12.^2.*q13.^2+q13.^4+(-2).*q11.* ...
  q12.*q13.*q14+q13.^2.*q14.^2).*sin((1/2).*t.*theta).^4)).^(-1)+(-1/4).* ...
  theta.*csc((1/2).*theta).^4.*((-4).*csc((1/2).*theta).^2.*((-1).*( ...
  q02.^2+q03.^2).*theta.*cos((1/2).*(1+(-1).*t).*theta).*sin((1/2).*(1+( ...
  -1).*t).*theta)+(q02.*q12+q03.*q13).*theta.*cos((1/2).*t.*theta).*sin(( ...
  1/2).*(1+(-1).*t).*theta)+(-1).*(q02.*q12+q03.*q13).*theta.*cos((1/2).*( ...
  1+(-1).*t).*theta).*sin((1/2).*t.*theta)+(q12.^2+q13.^2).*theta.*cos(( ...
  1/2).*t.*theta).*sin((1/2).*t.*theta))+4.*csc((1/2).*theta).^4.*((-2).*( ...
  q01.^2.*q02.^2+q02.^4+2.*q02.^2.*q03.^2+q03.^4+(-2).*q01.*q02.*q03.*q04+ ...
  q03.^2.*q04.^2).*theta.*cos((1/2).*(1+(-1).*t).*theta).*sin((1/2).*(1+( ...
  -1).*t).*theta).^3+(q01.^2.*q02.*q12+2.*q02.^3.*q12+q02.*q03.*((-1).* ...
  q04.*q11+2.*q03.*q12)+2.*q02.^2.*q03.*q13+q03.*(2.*q03.^2.*q13+q04.^2.* ...
  q13+q03.*q04.*q14)+q01.*(q02.^2.*q11+(-1).*q03.*q04.*q12+(-1).*q02.*( ...
  q04.*q13+q03.*q14))).*theta.*cos((1/2).*t.*theta).*sin((1/2).*(1+(-1).* ...
  t).*theta).^3+(-3).*(q01.^2.*q02.*q12+2.*q02.^3.*q12+q02.*q03.*((-1).* ...
  q04.*q11+2.*q03.*q12)+2.*q02.^2.*q03.*q13+q03.*(2.*q03.^2.*q13+q04.^2.* ...
  q13+q03.*q04.*q14)+q01.*(q02.^2.*q11+(-1).*q03.*q04.*q12+(-1).*q02.*( ...
  q04.*q13+q03.*q14))).*theta.*cos((1/2).*(1+(-1).*t).*theta).*sin((1/2).* ...
  (1+(-1).*t).*theta).^2.*sin((1/2).*t.*theta)+((q01.*q12+(-1).*q04.*q13) ...
  .^2+q02.^2.*(q11.^2+6.*q12.^2+2.*q13.^2)+q02.*(4.*q01.*q11.*q12+(-2).* ...
  q04.*q11.*q13+8.*q03.*q12.*q13+(-2).*q03.*q11.*q14+(-2).*q01.*q13.*q14)+ ...
  (-2).*q03.*(q04.*q11.*q12+q01.*q12.*q14+(-2).*q04.*q13.*q14)+q03.^2.*( ...
  2.*q12.^2+6.*q13.^2+q14.^2)).*theta.*cos((1/2).*t.*theta).*sin((1/2).*( ...
  1+(-1).*t).*theta).^2.*sin((1/2).*t.*theta)+(-1).*((q01.*q12+(-1).*q04.* ...
  q13).^2+q02.^2.*(q11.^2+6.*q12.^2+2.*q13.^2)+q02.*(4.*q01.*q11.*q12+(-2) ...
  .*q04.*q11.*q13+8.*q03.*q12.*q13+(-2).*q03.*q11.*q14+(-2).*q01.*q13.* ...
  q14)+(-2).*q03.*(q04.*q11.*q12+q01.*q12.*q14+(-2).*q04.*q13.*q14)+ ...
  q03.^2.*(2.*q12.^2+6.*q13.^2+q14.^2)).*theta.*cos((1/2).*(1+(-1).*t).* ...
  theta).*sin((1/2).*(1+(-1).*t).*theta).*sin((1/2).*t.*theta).^2+3.*((-1) ...
  .*q04.*q11.*q12.*q13+2.*q03.*q12.^2.*q13+2.*q03.*q13.^3+(-1).*q03.*q11.* ...
  q12.*q14+q04.*q13.^2.*q14+q03.*q13.*q14.^2+q01.*q12.*(q11.*q12+(-1).* ...
  q13.*q14)+q02.*(q11.^2.*q12+2.*q12.*(q12.^2+q13.^2)+(-1).*q11.*q13.*q14) ...
  ).*theta.*cos((1/2).*t.*theta).*sin((1/2).*(1+(-1).*t).*theta).*sin(( ...
  1/2).*t.*theta).^2+(-1).*((-1).*q04.*q11.*q12.*q13+2.*q03.*q12.^2.*q13+ ...
  2.*q03.*q13.^3+(-1).*q03.*q11.*q12.*q14+q04.*q13.^2.*q14+q03.*q13.* ...
  q14.^2+q01.*q12.*(q11.*q12+(-1).*q13.*q14)+q02.*(q11.^2.*q12+2.*q12.*( ...
  q12.^2+q13.^2)+(-1).*q11.*q13.*q14)).*theta.*cos((1/2).*(1+(-1).*t).* ...
  theta).*sin((1/2).*t.*theta).^3+2.*(q11.^2.*q12.^2+q12.^4+2.*q12.^2.* ...
  q13.^2+q13.^4+(-2).*q11.*q12.*q13.*q14+q13.^2.*q14.^2).*theta.*cos((1/2) ...
  .*t.*theta).*sin((1/2).*t.*theta).^3)).*(1+(-4).*csc((1/2).*theta).^2.*( ...
  (q02.^2+q03.^2).*sin((1/2).*(1+(-1).*t).*theta).^2+2.*(q02.*q12+q03.* ...
  q13).*sin((1/2).*(1+(-1).*t).*theta).*sin((1/2).*t.*theta)+(q12.^2+ ...
  q13.^2).*sin((1/2).*t.*theta).^2)+4.*csc((1/2).*theta).^4.*((q01.^2.* ...
  q02.^2+q02.^4+2.*q02.^2.*q03.^2+q03.^4+(-2).*q01.*q02.*q03.*q04+q03.^2.* ...
  q04.^2).*sin((1/2).*(1+(-1).*t).*theta).^4+2.*(q01.^2.*q02.*q12+2.* ...
  q02.^3.*q12+q02.*q03.*((-1).*q04.*q11+2.*q03.*q12)+2.*q02.^2.*q03.*q13+ ...
  q03.*(2.*q03.^2.*q13+q04.^2.*q13+q03.*q04.*q14)+q01.*(q02.^2.*q11+(-1).* ...
  q03.*q04.*q12+(-1).*q02.*(q04.*q13+q03.*q14))).*sin((1/2).*(1+(-1).*t).* ...
  theta).^3.*sin((1/2).*t.*theta)+((q01.*q12+(-1).*q04.*q13).^2+q02.^2.*( ...
  q11.^2+6.*q12.^2+2.*q13.^2)+q02.*(4.*q01.*q11.*q12+(-2).*q04.*q11.*q13+ ...
  8.*q03.*q12.*q13+(-2).*q03.*q11.*q14+(-2).*q01.*q13.*q14)+(-2).*q03.*( ...
  q04.*q11.*q12+q01.*q12.*q14+(-2).*q04.*q13.*q14)+q03.^2.*(2.*q12.^2+6.* ...
  q13.^2+q14.^2)).*sin((1/2).*(1+(-1).*t).*theta).^2.*sin((1/2).*t.*theta) ...
  .^2+2.*((-1).*q04.*q11.*q12.*q13+2.*q03.*q12.^2.*q13+2.*q03.*q13.^3+(-1) ...
  .*q03.*q11.*q12.*q14+q04.*q13.^2.*q14+q03.*q13.*q14.^2+q01.*q12.*(q11.* ...
  q12+(-1).*q13.*q14)+q02.*(q11.^2.*q12+2.*q12.*(q12.^2+q13.^2)+(-1).* ...
  q11.*q13.*q14)).*sin((1/2).*(1+(-1).*t).*theta).*sin((1/2).*t.*theta) ...
  .^3+(q11.^2.*q12.^2+q12.^4+2.*q12.^2.*q13.^2+q13.^4+(-2).*q11.*q12.* ...
  q13.*q14+q13.^2.*q14.^2).*sin((1/2).*t.*theta).^4)).^(-2).*((-4).*( ...
  q02.^3.*q11+q03.^2.*q04.*q13+2.*q03.*q11.*q12.*q13+q04.*q12.^2.*q13+ ...
  q04.*q13.^3+(-1).*q01.*q12.*((-1).*q03.^2+q12.^2+q13.^2)+(-1).*q03.^3.* ...
  q14+q03.*q12.^2.*q14+(-1).*q03.*q13.^2.*q14+(-1).*q02.^2.*(q01.*q12+ ...
  q04.*q13+q03.*q14)+q02.*(q03.^2.*q11+2.*q03.*q04.*q12+q11.*q12.^2+(-2).* ...
  q01.*q03.*q13+(-1).*q11.*q13.^2+(-2).*q12.*q13.*q14)).*sin((1/2).*theta) ...
  +4.*((-1).*q01.*q02.*(q12.^2+q13.^2)+q02.^2.*(q11.*q12+(-1).*q13.*q14)+ ...
  q03.*(q04.*(q12.^2+q13.^2)+q03.*(q11.*q12+(-1).*q13.*q14))).*sin(theta)+ ...
  (-1).*q02.*q11.*sin(((3/2)+(-1).*t).*theta)+2.*q02.^3.*q11.*sin(((3/2)+( ...
  -1).*t).*theta)+2.*q02.*q03.^2.*q11.*sin(((3/2)+(-1).*t).*theta)+(-1).* ...
  q01.*q12.*sin(((3/2)+(-1).*t).*theta)+(-2).*q01.*q02.^2.*q12.*sin(((3/2) ...
  +(-1).*t).*theta)+2.*q01.*q03.^2.*q12.*sin(((3/2)+(-1).*t).*theta)+4.* ...
  q02.*q03.*q04.*q12.*sin(((3/2)+(-1).*t).*theta)+(-4).*q01.*q02.*q03.* ...
  q13.*sin(((3/2)+(-1).*t).*theta)+q04.*q13.*sin(((3/2)+(-1).*t).*theta)+( ...
  -2).*q02.^2.*q04.*q13.*sin(((3/2)+(-1).*t).*theta)+2.*q03.^2.*q04.*q13.* ...
  sin(((3/2)+(-1).*t).*theta)+q03.*q14.*sin(((3/2)+(-1).*t).*theta)+(-2).* ...
  q02.^2.*q03.*q14.*sin(((3/2)+(-1).*t).*theta)+(-2).*q03.^3.*q14.*sin((( ...
  3/2)+(-1).*t).*theta)+(-1).*q01.*q02.*sin(((-2)+t).*theta)+q03.*q04.* ...
  sin(((-2)+t).*theta)+(-1).*q01.*q02.*sin(t.*theta)+q03.*q04.*sin(t.* ...
  theta)+2.*q11.*q12.*sin(t.*theta)+(-4).*q02.^2.*q11.*q12.*sin(t.*theta)+ ...
  (-4).*q03.^2.*q11.*q12.*sin(t.*theta)+4.*q01.*q02.*q12.^2.*sin(t.*theta) ...
  +(-4).*q03.*q04.*q12.^2.*sin(t.*theta)+4.*q01.*q02.*q13.^2.*sin(t.* ...
  theta)+(-4).*q03.*q04.*q13.^2.*sin(t.*theta)+(-2).*q13.*q14.*sin(t.* ...
  theta)+4.*q02.^2.*q13.*q14.*sin(t.*theta)+4.*q03.^2.*q13.*q14.*sin(t.* ...
  theta)+q02.*q11.*sin(((1/2)+t).*theta)+q01.*q12.*sin(((1/2)+t).*theta)+ ...
  2.*q02.*q11.*q12.^2.*sin(((1/2)+t).*theta)+(-2).*q01.*q12.^3.*sin(((1/2) ...
  +t).*theta)+(-1).*q04.*q13.*sin(((1/2)+t).*theta)+4.*q03.*q11.*q12.* ...
  q13.*sin(((1/2)+t).*theta)+2.*q04.*q12.^2.*q13.*sin(((1/2)+t).*theta)+( ...
  -2).*q02.*q11.*q13.^2.*sin(((1/2)+t).*theta)+(-2).*q01.*q12.*q13.^2.* ...
  sin(((1/2)+t).*theta)+2.*q04.*q13.^3.*sin(((1/2)+t).*theta)+(-1).*q03.* ...
  q14.*sin(((1/2)+t).*theta)+2.*q03.*q12.^2.*q14.*sin(((1/2)+t).*theta)+( ...
  -4).*q02.*q12.*q13.*q14.*sin(((1/2)+t).*theta)+(-2).*q03.*q13.^2.*q14.* ...
  sin(((1/2)+t).*theta)+(-1).*q11.*q12.*sin((1+t).*theta)+q13.*q14.*sin(( ...
  1+t).*theta)+2.*q02.*q11.*sin((1/2).*(theta+(-2).*t.*theta))+(-2).* ...
  q02.^3.*q11.*sin((1/2).*(theta+(-2).*t.*theta))+(-2).*q02.*q03.^2.*q11.* ...
  sin((1/2).*(theta+(-2).*t.*theta))+2.*q01.*q12.*sin((1/2).*(theta+(-2).* ...
  t.*theta))+2.*q01.*q02.^2.*q12.*sin((1/2).*(theta+(-2).*t.*theta))+(-2) ...
  .*q01.*q03.^2.*q12.*sin((1/2).*(theta+(-2).*t.*theta))+(-4).*q02.*q03.* ...
  q04.*q12.*sin((1/2).*(theta+(-2).*t.*theta))+2.*q02.*q11.*q12.^2.*sin(( ...
  1/2).*(theta+(-2).*t.*theta))+(-2).*q01.*q12.^3.*sin((1/2).*(theta+(-2) ...
  .*t.*theta))+4.*q01.*q02.*q03.*q13.*sin((1/2).*(theta+(-2).*t.*theta))+( ...
  -2).*q04.*q13.*sin((1/2).*(theta+(-2).*t.*theta))+2.*q02.^2.*q04.*q13.* ...
  sin((1/2).*(theta+(-2).*t.*theta))+(-2).*q03.^2.*q04.*q13.*sin((1/2).*( ...
  theta+(-2).*t.*theta))+4.*q03.*q11.*q12.*q13.*sin((1/2).*(theta+(-2).* ...
  t.*theta))+2.*q04.*q12.^2.*q13.*sin((1/2).*(theta+(-2).*t.*theta))+(-2) ...
  .*q02.*q11.*q13.^2.*sin((1/2).*(theta+(-2).*t.*theta))+(-2).*q01.*q12.* ...
  q13.^2.*sin((1/2).*(theta+(-2).*t.*theta))+2.*q04.*q13.^3.*sin((1/2).*( ...
  theta+(-2).*t.*theta))+(-2).*q03.*q14.*sin((1/2).*(theta+(-2).*t.*theta) ...
  )+2.*q02.^2.*q03.*q14.*sin((1/2).*(theta+(-2).*t.*theta))+2.*q03.^3.* ...
  q14.*sin((1/2).*(theta+(-2).*t.*theta))+2.*q03.*q12.^2.*q14.*sin((1/2).* ...
  (theta+(-2).*t.*theta))+(-4).*q02.*q12.*q13.*q14.*sin((1/2).*(theta+(-2) ...
  .*t.*theta))+(-2).*q03.*q13.^2.*q14.*sin((1/2).*(theta+(-2).*t.*theta))+ ...
  (-2).*q01.*q02.*sin(theta+(-1).*t.*theta)+2.*q03.*q04.*sin(theta+(-1).* ...
  t.*theta)+q11.*q12.*sin(theta+(-1).*t.*theta)+(-4).*q02.^2.*q11.*q12.* ...
  sin(theta+(-1).*t.*theta)+(-4).*q03.^2.*q11.*q12.*sin(theta+(-1).*t.* ...
  theta)+4.*q01.*q02.*q12.^2.*sin(theta+(-1).*t.*theta)+(-4).*q03.*q04.* ...
  q12.^2.*sin(theta+(-1).*t.*theta)+4.*q01.*q02.*q13.^2.*sin(theta+(-1).* ...
  t.*theta)+(-4).*q03.*q04.*q13.^2.*sin(theta+(-1).*t.*theta)+(-1).*q13.* ...
  q14.*sin(theta+(-1).*t.*theta)+4.*q02.^2.*q13.*q14.*sin(theta+(-1).*t.* ...
  theta)+4.*q03.^2.*q13.*q14.*sin(theta+(-1).*t.*theta));

ddth2_des = (csc((1/2).*theta).^2.*(q01.*sin((1/2).*(1+(-1).*t).*theta)+q11.*sin(( ...
  1/2).*t.*theta)).*(q03.*sin((1/2).*(1+(-1).*t).*theta)+q13.*sin((1/2).* ...
  t.*theta))+csc((1/2).*theta).^2.*(q02.*sin((1/2).*(1+(-1).*t).*theta)+ ...
  q12.*sin((1/2).*t.*theta)).*(q04.*sin((1/2).*(1+(-1).*t).*theta)+q14.* ...
  sin((1/2).*t.*theta))).*(8.*((-1).*((-1/2).*q02.*theta.*cos((1/2).*(1+( ...
  -1).*t).*theta)+(1/2).*q12.*theta.*cos((1/2).*t.*theta)).*csc((1/2).* ...
  theta).^2.*(q01.*sin((1/2).*(1+(-1).*t).*theta)+q11.*sin((1/2).*t.* ...
  theta))+(-1).*((-1/2).*q01.*theta.*cos((1/2).*(1+(-1).*t).*theta)+(1/2) ...
  .*q11.*theta.*cos((1/2).*t.*theta)).*csc((1/2).*theta).^2.*(q02.*sin(( ...
  1/2).*(1+(-1).*t).*theta)+q12.*sin((1/2).*t.*theta))+((-1/2).*q04.* ...
  theta.*cos((1/2).*(1+(-1).*t).*theta)+(1/2).*q14.*theta.*cos((1/2).*t.* ...
  theta)).*csc((1/2).*theta).^2.*(q03.*sin((1/2).*(1+(-1).*t).*theta)+ ...
  q13.*sin((1/2).*t.*theta))+((-1/2).*q03.*theta.*cos((1/2).*(1+(-1).*t).* ...
  theta)+(1/2).*q13.*theta.*cos((1/2).*t.*theta)).*csc((1/2).*theta).^2.*( ...
  q04.*sin((1/2).*(1+(-1).*t).*theta)+q14.*sin((1/2).*t.*theta))).*((-1).* ...
  csc((1/2).*theta).^2.*(q01.*sin((1/2).*(1+(-1).*t).*theta)+q11.*sin(( ...
  1/2).*t.*theta)).*(q02.*sin((1/2).*(1+(-1).*t).*theta)+q12.*sin((1/2).* ...
  t.*theta))+csc((1/2).*theta).^2.*(q03.*sin((1/2).*(1+(-1).*t).*theta)+ ...
  q13.*sin((1/2).*t.*theta)).*(q04.*sin((1/2).*(1+(-1).*t).*theta)+q14.* ...
  sin((1/2).*t.*theta)))+(-4).*(2.*((-1/2).*q02.*theta.*cos((1/2).*(1+(-1) ...
  .*t).*theta)+(1/2).*q12.*theta.*cos((1/2).*t.*theta)).*csc((1/2).*theta) ...
  .^2.*(q02.*sin((1/2).*(1+(-1).*t).*theta)+q12.*sin((1/2).*t.*theta))+2.* ...
  ((-1/2).*q03.*theta.*cos((1/2).*(1+(-1).*t).*theta)+(1/2).*q13.*theta.* ...
  cos((1/2).*t.*theta)).*csc((1/2).*theta).^2.*(q03.*sin((1/2).*(1+(-1).* ...
  t).*theta)+q13.*sin((1/2).*t.*theta))).*(1+(-2).*(csc((1/2).*theta).^2.* ...
  (q02.*sin((1/2).*(1+(-1).*t).*theta)+q12.*sin((1/2).*t.*theta)).^2+csc(( ...
  1/2).*theta).^2.*(q03.*sin((1/2).*(1+(-1).*t).*theta)+q13.*sin((1/2).* ...
  t.*theta)).^2))).*(8.*(((-1/2).*q03.*theta.*cos((1/2).*(1+(-1).*t).* ...
  theta)+(1/2).*q13.*theta.*cos((1/2).*t.*theta)).*csc((1/2).*theta).^2.*( ...
  q01.*sin((1/2).*(1+(-1).*t).*theta)+q11.*sin((1/2).*t.*theta))+((-1/2).* ...
  q04.*theta.*cos((1/2).*(1+(-1).*t).*theta)+(1/2).*q14.*theta.*cos((1/2) ...
  .*t.*theta)).*csc((1/2).*theta).^2.*(q02.*sin((1/2).*(1+(-1).*t).*theta) ...
  +q12.*sin((1/2).*t.*theta))+((-1/2).*q01.*theta.*cos((1/2).*(1+(-1).*t) ...
  .*theta)+(1/2).*q11.*theta.*cos((1/2).*t.*theta)).*csc((1/2).*theta) ...
  .^2.*(q03.*sin((1/2).*(1+(-1).*t).*theta)+q13.*sin((1/2).*t.*theta))+(( ...
  -1/2).*q02.*theta.*cos((1/2).*(1+(-1).*t).*theta)+(1/2).*q12.*theta.* ...
  cos((1/2).*t.*theta)).*csc((1/2).*theta).^2.*(q04.*sin((1/2).*(1+(-1).* ...
  t).*theta)+q14.*sin((1/2).*t.*theta))).*(csc((1/2).*theta).^2.*(q01.* ...
  sin((1/2).*(1+(-1).*t).*theta)+q11.*sin((1/2).*t.*theta)).*(q03.*sin(( ...
  1/2).*(1+(-1).*t).*theta)+q13.*sin((1/2).*t.*theta))+csc((1/2).*theta) ...
  .^2.*(q02.*sin((1/2).*(1+(-1).*t).*theta)+q12.*sin((1/2).*t.*theta)).*( ...
  q04.*sin((1/2).*(1+(-1).*t).*theta)+q14.*sin((1/2).*t.*theta)))+8.*((-1) ...
  .*((-1/2).*q02.*theta.*cos((1/2).*(1+(-1).*t).*theta)+(1/2).*q12.* ...
  theta.*cos((1/2).*t.*theta)).*csc((1/2).*theta).^2.*(q01.*sin((1/2).*(1+ ...
  (-1).*t).*theta)+q11.*sin((1/2).*t.*theta))+(-1).*((-1/2).*q01.*theta.* ...
  cos((1/2).*(1+(-1).*t).*theta)+(1/2).*q11.*theta.*cos((1/2).*t.*theta)) ...
  .*csc((1/2).*theta).^2.*(q02.*sin((1/2).*(1+(-1).*t).*theta)+q12.*sin(( ...
  1/2).*t.*theta))+((-1/2).*q04.*theta.*cos((1/2).*(1+(-1).*t).*theta)+( ...
  1/2).*q14.*theta.*cos((1/2).*t.*theta)).*csc((1/2).*theta).^2.*(q03.* ...
  sin((1/2).*(1+(-1).*t).*theta)+q13.*sin((1/2).*t.*theta))+((-1/2).*q03.* ...
  theta.*cos((1/2).*(1+(-1).*t).*theta)+(1/2).*q13.*theta.*cos((1/2).*t.* ...
  theta)).*csc((1/2).*theta).^2.*(q04.*sin((1/2).*(1+(-1).*t).*theta)+ ...
  q14.*sin((1/2).*t.*theta))).*((-1).*csc((1/2).*theta).^2.*(q01.*sin(( ...
  1/2).*(1+(-1).*t).*theta)+q11.*sin((1/2).*t.*theta)).*(q02.*sin((1/2).*( ...
  1+(-1).*t).*theta)+q12.*sin((1/2).*t.*theta))+csc((1/2).*theta).^2.*( ...
  q03.*sin((1/2).*(1+(-1).*t).*theta)+q13.*sin((1/2).*t.*theta)).*(q04.* ...
  sin((1/2).*(1+(-1).*t).*theta)+q14.*sin((1/2).*t.*theta)))+(-4).*(2.*(( ...
  -1/2).*q02.*theta.*cos((1/2).*(1+(-1).*t).*theta)+(1/2).*q12.*theta.* ...
  cos((1/2).*t.*theta)).*csc((1/2).*theta).^2.*(q02.*sin((1/2).*(1+(-1).* ...
  t).*theta)+q12.*sin((1/2).*t.*theta))+2.*((-1/2).*q03.*theta.*cos((1/2) ...
  .*(1+(-1).*t).*theta)+(1/2).*q13.*theta.*cos((1/2).*t.*theta)).*csc(( ...
  1/2).*theta).^2.*(q03.*sin((1/2).*(1+(-1).*t).*theta)+q13.*sin((1/2).* ...
  t.*theta))).*(1+(-2).*(csc((1/2).*theta).^2.*(q02.*sin((1/2).*(1+(-1).* ...
  t).*theta)+q12.*sin((1/2).*t.*theta)).^2+csc((1/2).*theta).^2.*(q03.* ...
  sin((1/2).*(1+(-1).*t).*theta)+q13.*sin((1/2).*t.*theta)).^2))).*(4.*(( ...
  -1).*csc((1/2).*theta).^2.*(q01.*sin((1/2).*(1+(-1).*t).*theta)+q11.* ...
  sin((1/2).*t.*theta)).*(q02.*sin((1/2).*(1+(-1).*t).*theta)+q12.*sin(( ...
  1/2).*t.*theta))+csc((1/2).*theta).^2.*(q03.*sin((1/2).*(1+(-1).*t).* ...
  theta)+q13.*sin((1/2).*t.*theta)).*(q04.*sin((1/2).*(1+(-1).*t).*theta)+ ...
  q14.*sin((1/2).*t.*theta))).^2+(1+(-2).*(csc((1/2).*theta).^2.*(q02.* ...
  sin((1/2).*(1+(-1).*t).*theta)+q12.*sin((1/2).*t.*theta)).^2+csc((1/2).* ...
  theta).^2.*(q03.*sin((1/2).*(1+(-1).*t).*theta)+q13.*sin((1/2).*t.* ...
  theta)).^2)).^2).^(-1/2).*(4.*(csc((1/2).*theta).^2.*(q01.*sin((1/2).*( ...
  1+(-1).*t).*theta)+q11.*sin((1/2).*t.*theta)).*(q03.*sin((1/2).*(1+(-1) ...
  .*t).*theta)+q13.*sin((1/2).*t.*theta))+csc((1/2).*theta).^2.*(q02.*sin( ...
  (1/2).*(1+(-1).*t).*theta)+q12.*sin((1/2).*t.*theta)).*(q04.*sin((1/2).* ...
  (1+(-1).*t).*theta)+q14.*sin((1/2).*t.*theta))).^2+4.*((-1).*csc((1/2).* ...
  theta).^2.*(q01.*sin((1/2).*(1+(-1).*t).*theta)+q11.*sin((1/2).*t.* ...
  theta)).*(q02.*sin((1/2).*(1+(-1).*t).*theta)+q12.*sin((1/2).*t.*theta)) ...
  +csc((1/2).*theta).^2.*(q03.*sin((1/2).*(1+(-1).*t).*theta)+q13.*sin(( ...
  1/2).*t.*theta)).*(q04.*sin((1/2).*(1+(-1).*t).*theta)+q14.*sin((1/2).* ...
  t.*theta))).^2+(1+(-2).*(csc((1/2).*theta).^2.*(q02.*sin((1/2).*(1+(-1) ...
  .*t).*theta)+q12.*sin((1/2).*t.*theta)).^2+csc((1/2).*theta).^2.*(q03.* ...
  sin((1/2).*(1+(-1).*t).*theta)+q13.*sin((1/2).*t.*theta)).^2)).^2).^(-2) ...
  +(-2).*(((-1/2).*q03.*theta.*cos((1/2).*(1+(-1).*t).*theta)+(1/2).*q13.* ...
  theta.*cos((1/2).*t.*theta)).*csc((1/2).*theta).^2.*(q01.*sin((1/2).*(1+ ...
  (-1).*t).*theta)+q11.*sin((1/2).*t.*theta))+((-1/2).*q04.*theta.*cos(( ...
  1/2).*(1+(-1).*t).*theta)+(1/2).*q14.*theta.*cos((1/2).*t.*theta)).*csc( ...
  (1/2).*theta).^2.*(q02.*sin((1/2).*(1+(-1).*t).*theta)+q12.*sin((1/2).* ...
  t.*theta))+((-1/2).*q01.*theta.*cos((1/2).*(1+(-1).*t).*theta)+(1/2).* ...
  q11.*theta.*cos((1/2).*t.*theta)).*csc((1/2).*theta).^2.*(q03.*sin((1/2) ...
  .*(1+(-1).*t).*theta)+q13.*sin((1/2).*t.*theta))+((-1/2).*q02.*theta.* ...
  cos((1/2).*(1+(-1).*t).*theta)+(1/2).*q12.*theta.*cos((1/2).*t.*theta)) ...
  .*csc((1/2).*theta).^2.*(q04.*sin((1/2).*(1+(-1).*t).*theta)+q14.*sin(( ...
  1/2).*t.*theta))).*(8.*(((-1/2).*q03.*theta.*cos((1/2).*(1+(-1).*t).* ...
  theta)+(1/2).*q13.*theta.*cos((1/2).*t.*theta)).*csc((1/2).*theta).^2.*( ...
  q01.*sin((1/2).*(1+(-1).*t).*theta)+q11.*sin((1/2).*t.*theta))+((-1/2).* ...
  q04.*theta.*cos((1/2).*(1+(-1).*t).*theta)+(1/2).*q14.*theta.*cos((1/2) ...
  .*t.*theta)).*csc((1/2).*theta).^2.*(q02.*sin((1/2).*(1+(-1).*t).*theta) ...
  +q12.*sin((1/2).*t.*theta))+((-1/2).*q01.*theta.*cos((1/2).*(1+(-1).*t) ...
  .*theta)+(1/2).*q11.*theta.*cos((1/2).*t.*theta)).*csc((1/2).*theta) ...
  .^2.*(q03.*sin((1/2).*(1+(-1).*t).*theta)+q13.*sin((1/2).*t.*theta))+(( ...
  -1/2).*q02.*theta.*cos((1/2).*(1+(-1).*t).*theta)+(1/2).*q12.*theta.* ...
  cos((1/2).*t.*theta)).*csc((1/2).*theta).^2.*(q04.*sin((1/2).*(1+(-1).* ...
  t).*theta)+q14.*sin((1/2).*t.*theta))).*(csc((1/2).*theta).^2.*(q01.* ...
  sin((1/2).*(1+(-1).*t).*theta)+q11.*sin((1/2).*t.*theta)).*(q03.*sin(( ...
  1/2).*(1+(-1).*t).*theta)+q13.*sin((1/2).*t.*theta))+csc((1/2).*theta) ...
  .^2.*(q02.*sin((1/2).*(1+(-1).*t).*theta)+q12.*sin((1/2).*t.*theta)).*( ...
  q04.*sin((1/2).*(1+(-1).*t).*theta)+q14.*sin((1/2).*t.*theta)))+8.*((-1) ...
  .*((-1/2).*q02.*theta.*cos((1/2).*(1+(-1).*t).*theta)+(1/2).*q12.* ...
  theta.*cos((1/2).*t.*theta)).*csc((1/2).*theta).^2.*(q01.*sin((1/2).*(1+ ...
  (-1).*t).*theta)+q11.*sin((1/2).*t.*theta))+(-1).*((-1/2).*q01.*theta.* ...
  cos((1/2).*(1+(-1).*t).*theta)+(1/2).*q11.*theta.*cos((1/2).*t.*theta)) ...
  .*csc((1/2).*theta).^2.*(q02.*sin((1/2).*(1+(-1).*t).*theta)+q12.*sin(( ...
  1/2).*t.*theta))+((-1/2).*q04.*theta.*cos((1/2).*(1+(-1).*t).*theta)+( ...
  1/2).*q14.*theta.*cos((1/2).*t.*theta)).*csc((1/2).*theta).^2.*(q03.* ...
  sin((1/2).*(1+(-1).*t).*theta)+q13.*sin((1/2).*t.*theta))+((-1/2).*q03.* ...
  theta.*cos((1/2).*(1+(-1).*t).*theta)+(1/2).*q13.*theta.*cos((1/2).*t.* ...
  theta)).*csc((1/2).*theta).^2.*(q04.*sin((1/2).*(1+(-1).*t).*theta)+ ...
  q14.*sin((1/2).*t.*theta))).*((-1).*csc((1/2).*theta).^2.*(q01.*sin(( ...
  1/2).*(1+(-1).*t).*theta)+q11.*sin((1/2).*t.*theta)).*(q02.*sin((1/2).*( ...
  1+(-1).*t).*theta)+q12.*sin((1/2).*t.*theta))+csc((1/2).*theta).^2.*( ...
  q03.*sin((1/2).*(1+(-1).*t).*theta)+q13.*sin((1/2).*t.*theta)).*(q04.* ...
  sin((1/2).*(1+(-1).*t).*theta)+q14.*sin((1/2).*t.*theta)))+(-4).*(2.*(( ...
  -1/2).*q02.*theta.*cos((1/2).*(1+(-1).*t).*theta)+(1/2).*q12.*theta.* ...
  cos((1/2).*t.*theta)).*csc((1/2).*theta).^2.*(q02.*sin((1/2).*(1+(-1).* ...
  t).*theta)+q12.*sin((1/2).*t.*theta))+2.*((-1/2).*q03.*theta.*cos((1/2) ...
  .*(1+(-1).*t).*theta)+(1/2).*q13.*theta.*cos((1/2).*t.*theta)).*csc(( ...
  1/2).*theta).^2.*(q03.*sin((1/2).*(1+(-1).*t).*theta)+q13.*sin((1/2).* ...
  t.*theta))).*(1+(-2).*(csc((1/2).*theta).^2.*(q02.*sin((1/2).*(1+(-1).* ...
  t).*theta)+q12.*sin((1/2).*t.*theta)).^2+csc((1/2).*theta).^2.*(q03.* ...
  sin((1/2).*(1+(-1).*t).*theta)+q13.*sin((1/2).*t.*theta)).^2))).*(4.*(( ...
  -1).*csc((1/2).*theta).^2.*(q01.*sin((1/2).*(1+(-1).*t).*theta)+q11.* ...
  sin((1/2).*t.*theta)).*(q02.*sin((1/2).*(1+(-1).*t).*theta)+q12.*sin(( ...
  1/2).*t.*theta))+csc((1/2).*theta).^2.*(q03.*sin((1/2).*(1+(-1).*t).* ...
  theta)+q13.*sin((1/2).*t.*theta)).*(q04.*sin((1/2).*(1+(-1).*t).*theta)+ ...
  q14.*sin((1/2).*t.*theta))).^2+(1+(-2).*(csc((1/2).*theta).^2.*(q02.* ...
  sin((1/2).*(1+(-1).*t).*theta)+q12.*sin((1/2).*t.*theta)).^2+csc((1/2).* ...
  theta).^2.*(q03.*sin((1/2).*(1+(-1).*t).*theta)+q13.*sin((1/2).*t.* ...
  theta)).^2)).^2).^(1/2).*(4.*(csc((1/2).*theta).^2.*(q01.*sin((1/2).*(1+ ...
  (-1).*t).*theta)+q11.*sin((1/2).*t.*theta)).*(q03.*sin((1/2).*(1+(-1).* ...
  t).*theta)+q13.*sin((1/2).*t.*theta))+csc((1/2).*theta).^2.*(q02.*sin(( ...
  1/2).*(1+(-1).*t).*theta)+q12.*sin((1/2).*t.*theta)).*(q04.*sin((1/2).*( ...
  1+(-1).*t).*theta)+q14.*sin((1/2).*t.*theta))).^2+4.*((-1).*csc((1/2).* ...
  theta).^2.*(q01.*sin((1/2).*(1+(-1).*t).*theta)+q11.*sin((1/2).*t.* ...
  theta)).*(q02.*sin((1/2).*(1+(-1).*t).*theta)+q12.*sin((1/2).*t.*theta)) ...
  +csc((1/2).*theta).^2.*(q03.*sin((1/2).*(1+(-1).*t).*theta)+q13.*sin(( ...
  1/2).*t.*theta)).*(q04.*sin((1/2).*(1+(-1).*t).*theta)+q14.*sin((1/2).* ...
  t.*theta))).^2+(1+(-2).*(csc((1/2).*theta).^2.*(q02.*sin((1/2).*(1+(-1) ...
  .*t).*theta)+q12.*sin((1/2).*t.*theta)).^2+csc((1/2).*theta).^2.*(q03.* ...
  sin((1/2).*(1+(-1).*t).*theta)+q13.*sin((1/2).*t.*theta)).^2)).^2).^(-2) ...
  +(1/2).*(csc((1/2).*theta).^2.*(q01.*sin((1/2).*(1+(-1).*t).*theta)+ ...
  q11.*sin((1/2).*t.*theta)).*(q03.*sin((1/2).*(1+(-1).*t).*theta)+q13.* ...
  sin((1/2).*t.*theta))+csc((1/2).*theta).^2.*(q02.*sin((1/2).*(1+(-1).*t) ...
  .*theta)+q12.*sin((1/2).*t.*theta)).*(q04.*sin((1/2).*(1+(-1).*t).* ...
  theta)+q14.*sin((1/2).*t.*theta))).*(8.*((-1).*((-1/2).*q02.*theta.*cos( ...
  (1/2).*(1+(-1).*t).*theta)+(1/2).*q12.*theta.*cos((1/2).*t.*theta)).* ...
  csc((1/2).*theta).^2.*(q01.*sin((1/2).*(1+(-1).*t).*theta)+q11.*sin(( ...
  1/2).*t.*theta))+(-1).*((-1/2).*q01.*theta.*cos((1/2).*(1+(-1).*t).* ...
  theta)+(1/2).*q11.*theta.*cos((1/2).*t.*theta)).*csc((1/2).*theta).^2.*( ...
  q02.*sin((1/2).*(1+(-1).*t).*theta)+q12.*sin((1/2).*t.*theta))+((-1/2).* ...
  q04.*theta.*cos((1/2).*(1+(-1).*t).*theta)+(1/2).*q14.*theta.*cos((1/2) ...
  .*t.*theta)).*csc((1/2).*theta).^2.*(q03.*sin((1/2).*(1+(-1).*t).*theta) ...
  +q13.*sin((1/2).*t.*theta))+((-1/2).*q03.*theta.*cos((1/2).*(1+(-1).*t) ...
  .*theta)+(1/2).*q13.*theta.*cos((1/2).*t.*theta)).*csc((1/2).*theta) ...
  .^2.*(q04.*sin((1/2).*(1+(-1).*t).*theta)+q14.*sin((1/2).*t.*theta))).*( ...
  (-1).*csc((1/2).*theta).^2.*(q01.*sin((1/2).*(1+(-1).*t).*theta)+q11.* ...
  sin((1/2).*t.*theta)).*(q02.*sin((1/2).*(1+(-1).*t).*theta)+q12.*sin(( ...
  1/2).*t.*theta))+csc((1/2).*theta).^2.*(q03.*sin((1/2).*(1+(-1).*t).* ...
  theta)+q13.*sin((1/2).*t.*theta)).*(q04.*sin((1/2).*(1+(-1).*t).*theta)+ ...
  q14.*sin((1/2).*t.*theta)))+(-4).*(2.*((-1/2).*q02.*theta.*cos((1/2).*( ...
  1+(-1).*t).*theta)+(1/2).*q12.*theta.*cos((1/2).*t.*theta)).*csc((1/2).* ...
  theta).^2.*(q02.*sin((1/2).*(1+(-1).*t).*theta)+q12.*sin((1/2).*t.* ...
  theta))+2.*((-1/2).*q03.*theta.*cos((1/2).*(1+(-1).*t).*theta)+(1/2).* ...
  q13.*theta.*cos((1/2).*t.*theta)).*csc((1/2).*theta).^2.*(q03.*sin((1/2) ...
  .*(1+(-1).*t).*theta)+q13.*sin((1/2).*t.*theta))).*(1+(-2).*(csc((1/2).* ...
  theta).^2.*(q02.*sin((1/2).*(1+(-1).*t).*theta)+q12.*sin((1/2).*t.* ...
  theta)).^2+csc((1/2).*theta).^2.*(q03.*sin((1/2).*(1+(-1).*t).*theta)+ ...
  q13.*sin((1/2).*t.*theta)).^2))).^2.*(4.*((-1).*csc((1/2).*theta).^2.*( ...
  q01.*sin((1/2).*(1+(-1).*t).*theta)+q11.*sin((1/2).*t.*theta)).*(q02.* ...
  sin((1/2).*(1+(-1).*t).*theta)+q12.*sin((1/2).*t.*theta))+csc((1/2).* ...
  theta).^2.*(q03.*sin((1/2).*(1+(-1).*t).*theta)+q13.*sin((1/2).*t.* ...
  theta)).*(q04.*sin((1/2).*(1+(-1).*t).*theta)+q14.*sin((1/2).*t.*theta)) ...
  ).^2+(1+(-2).*(csc((1/2).*theta).^2.*(q02.*sin((1/2).*(1+(-1).*t).* ...
  theta)+q12.*sin((1/2).*t.*theta)).^2+csc((1/2).*theta).^2.*(q03.*sin(( ...
  1/2).*(1+(-1).*t).*theta)+q13.*sin((1/2).*t.*theta)).^2)).^2).^(-3/2).*( ...
  4.*(csc((1/2).*theta).^2.*(q01.*sin((1/2).*(1+(-1).*t).*theta)+q11.*sin( ...
  (1/2).*t.*theta)).*(q03.*sin((1/2).*(1+(-1).*t).*theta)+q13.*sin((1/2).* ...
  t.*theta))+csc((1/2).*theta).^2.*(q02.*sin((1/2).*(1+(-1).*t).*theta)+ ...
  q12.*sin((1/2).*t.*theta)).*(q04.*sin((1/2).*(1+(-1).*t).*theta)+q14.* ...
  sin((1/2).*t.*theta))).^2+4.*((-1).*csc((1/2).*theta).^2.*(q01.*sin(( ...
  1/2).*(1+(-1).*t).*theta)+q11.*sin((1/2).*t.*theta)).*(q02.*sin((1/2).*( ...
  1+(-1).*t).*theta)+q12.*sin((1/2).*t.*theta))+csc((1/2).*theta).^2.*( ...
  q03.*sin((1/2).*(1+(-1).*t).*theta)+q13.*sin((1/2).*t.*theta)).*(q04.* ...
  sin((1/2).*(1+(-1).*t).*theta)+q14.*sin((1/2).*t.*theta))).^2+(1+(-2).*( ...
  csc((1/2).*theta).^2.*(q02.*sin((1/2).*(1+(-1).*t).*theta)+q12.*sin(( ...
  1/2).*t.*theta)).^2+csc((1/2).*theta).^2.*(q03.*sin((1/2).*(1+(-1).*t).* ...
  theta)+q13.*sin((1/2).*t.*theta)).^2)).^2).^(-1)+(-1).*(csc((1/2).* ...
  theta).^2.*(q01.*sin((1/2).*(1+(-1).*t).*theta)+q11.*sin((1/2).*t.* ...
  theta)).*(q03.*sin((1/2).*(1+(-1).*t).*theta)+q13.*sin((1/2).*t.*theta)) ...
  +csc((1/2).*theta).^2.*(q02.*sin((1/2).*(1+(-1).*t).*theta)+q12.*sin(( ...
  1/2).*t.*theta)).*(q04.*sin((1/2).*(1+(-1).*t).*theta)+q14.*sin((1/2).* ...
  t.*theta))).*(8.*(2.*((-1/2).*q02.*theta.*cos((1/2).*(1+(-1).*t).*theta) ...
  +(1/2).*q12.*theta.*cos((1/2).*t.*theta)).*csc((1/2).*theta).^2.*(q02.* ...
  sin((1/2).*(1+(-1).*t).*theta)+q12.*sin((1/2).*t.*theta))+2.*((-1/2).* ...
  q03.*theta.*cos((1/2).*(1+(-1).*t).*theta)+(1/2).*q13.*theta.*cos((1/2) ...
  .*t.*theta)).*csc((1/2).*theta).^2.*(q03.*sin((1/2).*(1+(-1).*t).*theta) ...
  +q13.*sin((1/2).*t.*theta))).^2+8.*((-1).*((-1/2).*q02.*theta.*cos((1/2) ...
  .*(1+(-1).*t).*theta)+(1/2).*q12.*theta.*cos((1/2).*t.*theta)).*csc(( ...
  1/2).*theta).^2.*(q01.*sin((1/2).*(1+(-1).*t).*theta)+q11.*sin((1/2).* ...
  t.*theta))+(-1).*((-1/2).*q01.*theta.*cos((1/2).*(1+(-1).*t).*theta)+( ...
  1/2).*q11.*theta.*cos((1/2).*t.*theta)).*csc((1/2).*theta).^2.*(q02.* ...
  sin((1/2).*(1+(-1).*t).*theta)+q12.*sin((1/2).*t.*theta))+((-1/2).*q04.* ...
  theta.*cos((1/2).*(1+(-1).*t).*theta)+(1/2).*q14.*theta.*cos((1/2).*t.* ...
  theta)).*csc((1/2).*theta).^2.*(q03.*sin((1/2).*(1+(-1).*t).*theta)+ ...
  q13.*sin((1/2).*t.*theta))+((-1/2).*q03.*theta.*cos((1/2).*(1+(-1).*t).* ...
  theta)+(1/2).*q13.*theta.*cos((1/2).*t.*theta)).*csc((1/2).*theta).^2.*( ...
  q04.*sin((1/2).*(1+(-1).*t).*theta)+q14.*sin((1/2).*t.*theta))).^2+8.*(( ...
  -1).*csc((1/2).*theta).^2.*(q01.*sin((1/2).*(1+(-1).*t).*theta)+q11.* ...
  sin((1/2).*t.*theta)).*(q02.*sin((1/2).*(1+(-1).*t).*theta)+q12.*sin(( ...
  1/2).*t.*theta))+csc((1/2).*theta).^2.*(q03.*sin((1/2).*(1+(-1).*t).* ...
  theta)+q13.*sin((1/2).*t.*theta)).*(q04.*sin((1/2).*(1+(-1).*t).*theta)+ ...
  q14.*sin((1/2).*t.*theta))).*((-2).*((-1/2).*q01.*theta.*cos((1/2).*(1+( ...
  -1).*t).*theta)+(1/2).*q11.*theta.*cos((1/2).*t.*theta)).*((-1/2).*q02.* ...
  theta.*cos((1/2).*(1+(-1).*t).*theta)+(1/2).*q12.*theta.*cos((1/2).*t.* ...
  theta)).*csc((1/2).*theta).^2+2.*((-1/2).*q03.*theta.*cos((1/2).*(1+(-1) ...
  .*t).*theta)+(1/2).*q13.*theta.*cos((1/2).*t.*theta)).*((-1/2).*q04.* ...
  theta.*cos((1/2).*(1+(-1).*t).*theta)+(1/2).*q14.*theta.*cos((1/2).*t.* ...
  theta)).*csc((1/2).*theta).^2+(-1).*csc((1/2).*theta).^2.*(q02.*sin(( ...
  1/2).*(1+(-1).*t).*theta)+q12.*sin((1/2).*t.*theta)).*((-1/4).*q01.* ...
  theta.^2.*sin((1/2).*(1+(-1).*t).*theta)+(-1/4).*q11.*theta.^2.*sin(( ...
  1/2).*t.*theta))+(-1).*csc((1/2).*theta).^2.*(q01.*sin((1/2).*(1+(-1).* ...
  t).*theta)+q11.*sin((1/2).*t.*theta)).*((-1/4).*q02.*theta.^2.*sin((1/2) ...
  .*(1+(-1).*t).*theta)+(-1/4).*q12.*theta.^2.*sin((1/2).*t.*theta))+csc(( ...
  1/2).*theta).^2.*(q04.*sin((1/2).*(1+(-1).*t).*theta)+q14.*sin((1/2).* ...
  t.*theta)).*((-1/4).*q03.*theta.^2.*sin((1/2).*(1+(-1).*t).*theta)+( ...
  -1/4).*q13.*theta.^2.*sin((1/2).*t.*theta))+csc((1/2).*theta).^2.*(q03.* ...
  sin((1/2).*(1+(-1).*t).*theta)+q13.*sin((1/2).*t.*theta)).*((-1/4).* ...
  q04.*theta.^2.*sin((1/2).*(1+(-1).*t).*theta)+(-1/4).*q14.*theta.^2.* ...
  sin((1/2).*t.*theta)))+(-4).*(2.*((-1/2).*q02.*theta.*cos((1/2).*(1+(-1) ...
  .*t).*theta)+(1/2).*q12.*theta.*cos((1/2).*t.*theta)).^2.*csc((1/2).* ...
  theta).^2+2.*((-1/2).*q03.*theta.*cos((1/2).*(1+(-1).*t).*theta)+(1/2).* ...
  q13.*theta.*cos((1/2).*t.*theta)).^2.*csc((1/2).*theta).^2+2.*csc((1/2) ...
  .*theta).^2.*(q02.*sin((1/2).*(1+(-1).*t).*theta)+q12.*sin((1/2).*t.* ...
  theta)).*((-1/4).*q02.*theta.^2.*sin((1/2).*(1+(-1).*t).*theta)+(-1/4).* ...
  q12.*theta.^2.*sin((1/2).*t.*theta))+2.*csc((1/2).*theta).^2.*(q03.*sin( ...
  (1/2).*(1+(-1).*t).*theta)+q13.*sin((1/2).*t.*theta)).*((-1/4).*q03.* ...
  theta.^2.*sin((1/2).*(1+(-1).*t).*theta)+(-1/4).*q13.*theta.^2.*sin(( ...
  1/2).*t.*theta))).*(1+(-2).*(csc((1/2).*theta).^2.*(q02.*sin((1/2).*(1+( ...
  -1).*t).*theta)+q12.*sin((1/2).*t.*theta)).^2+csc((1/2).*theta).^2.*( ...
  q03.*sin((1/2).*(1+(-1).*t).*theta)+q13.*sin((1/2).*t.*theta)).^2))).*( ...
  4.*((-1).*csc((1/2).*theta).^2.*(q01.*sin((1/2).*(1+(-1).*t).*theta)+ ...
  q11.*sin((1/2).*t.*theta)).*(q02.*sin((1/2).*(1+(-1).*t).*theta)+q12.* ...
  sin((1/2).*t.*theta))+csc((1/2).*theta).^2.*(q03.*sin((1/2).*(1+(-1).*t) ...
  .*theta)+q13.*sin((1/2).*t.*theta)).*(q04.*sin((1/2).*(1+(-1).*t).* ...
  theta)+q14.*sin((1/2).*t.*theta))).^2+(1+(-2).*(csc((1/2).*theta).^2.*( ...
  q02.*sin((1/2).*(1+(-1).*t).*theta)+q12.*sin((1/2).*t.*theta)).^2+csc(( ...
  1/2).*theta).^2.*(q03.*sin((1/2).*(1+(-1).*t).*theta)+q13.*sin((1/2).* ...
  t.*theta)).^2)).^2).^(-1/2).*(4.*(csc((1/2).*theta).^2.*(q01.*sin((1/2) ...
  .*(1+(-1).*t).*theta)+q11.*sin((1/2).*t.*theta)).*(q03.*sin((1/2).*(1+( ...
  -1).*t).*theta)+q13.*sin((1/2).*t.*theta))+csc((1/2).*theta).^2.*(q02.* ...
  sin((1/2).*(1+(-1).*t).*theta)+q12.*sin((1/2).*t.*theta)).*(q04.*sin(( ...
  1/2).*(1+(-1).*t).*theta)+q14.*sin((1/2).*t.*theta))).^2+4.*((-1).*csc(( ...
  1/2).*theta).^2.*(q01.*sin((1/2).*(1+(-1).*t).*theta)+q11.*sin((1/2).* ...
  t.*theta)).*(q02.*sin((1/2).*(1+(-1).*t).*theta)+q12.*sin((1/2).*t.* ...
  theta))+csc((1/2).*theta).^2.*(q03.*sin((1/2).*(1+(-1).*t).*theta)+q13.* ...
  sin((1/2).*t.*theta)).*(q04.*sin((1/2).*(1+(-1).*t).*theta)+q14.*sin(( ...
  1/2).*t.*theta))).^2+(1+(-2).*(csc((1/2).*theta).^2.*(q02.*sin((1/2).*( ...
  1+(-1).*t).*theta)+q12.*sin((1/2).*t.*theta)).^2+csc((1/2).*theta).^2.*( ...
  q03.*sin((1/2).*(1+(-1).*t).*theta)+q13.*sin((1/2).*t.*theta)).^2)).^2) ...
  .^(-1)+2.*(2.*((-1/2).*q01.*theta.*cos((1/2).*(1+(-1).*t).*theta)+(1/2) ...
  .*q11.*theta.*cos((1/2).*t.*theta)).*((-1/2).*q03.*theta.*cos((1/2).*(1+ ...
  (-1).*t).*theta)+(1/2).*q13.*theta.*cos((1/2).*t.*theta)).*csc((1/2).* ...
  theta).^2+2.*((-1/2).*q02.*theta.*cos((1/2).*(1+(-1).*t).*theta)+(1/2).* ...
  q12.*theta.*cos((1/2).*t.*theta)).*((-1/2).*q04.*theta.*cos((1/2).*(1+( ...
  -1).*t).*theta)+(1/2).*q14.*theta.*cos((1/2).*t.*theta)).*csc((1/2).* ...
  theta).^2+csc((1/2).*theta).^2.*(q03.*sin((1/2).*(1+(-1).*t).*theta)+ ...
  q13.*sin((1/2).*t.*theta)).*((-1/4).*q01.*theta.^2.*sin((1/2).*(1+(-1).* ...
  t).*theta)+(-1/4).*q11.*theta.^2.*sin((1/2).*t.*theta))+csc((1/2).* ...
  theta).^2.*(q04.*sin((1/2).*(1+(-1).*t).*theta)+q14.*sin((1/2).*t.* ...
  theta)).*((-1/4).*q02.*theta.^2.*sin((1/2).*(1+(-1).*t).*theta)+(-1/4).* ...
  q12.*theta.^2.*sin((1/2).*t.*theta))+csc((1/2).*theta).^2.*(q01.*sin(( ...
  1/2).*(1+(-1).*t).*theta)+q11.*sin((1/2).*t.*theta)).*((-1/4).*q03.* ...
  theta.^2.*sin((1/2).*(1+(-1).*t).*theta)+(-1/4).*q13.*theta.^2.*sin(( ...
  1/2).*t.*theta))+csc((1/2).*theta).^2.*(q02.*sin((1/2).*(1+(-1).*t).* ...
  theta)+q12.*sin((1/2).*t.*theta)).*((-1/4).*q04.*theta.^2.*sin((1/2).*( ...
  1+(-1).*t).*theta)+(-1/4).*q14.*theta.^2.*sin((1/2).*t.*theta))).*(4.*(( ...
  -1).*csc((1/2).*theta).^2.*(q01.*sin((1/2).*(1+(-1).*t).*theta)+q11.* ...
  sin((1/2).*t.*theta)).*(q02.*sin((1/2).*(1+(-1).*t).*theta)+q12.*sin(( ...
  1/2).*t.*theta))+csc((1/2).*theta).^2.*(q03.*sin((1/2).*(1+(-1).*t).* ...
  theta)+q13.*sin((1/2).*t.*theta)).*(q04.*sin((1/2).*(1+(-1).*t).*theta)+ ...
  q14.*sin((1/2).*t.*theta))).^2+(1+(-2).*(csc((1/2).*theta).^2.*(q02.* ...
  sin((1/2).*(1+(-1).*t).*theta)+q12.*sin((1/2).*t.*theta)).^2+csc((1/2).* ...
  theta).^2.*(q03.*sin((1/2).*(1+(-1).*t).*theta)+q13.*sin((1/2).*t.* ...
  theta)).^2)).^2).^(1/2).*(4.*(csc((1/2).*theta).^2.*(q01.*sin((1/2).*(1+ ...
  (-1).*t).*theta)+q11.*sin((1/2).*t.*theta)).*(q03.*sin((1/2).*(1+(-1).* ...
  t).*theta)+q13.*sin((1/2).*t.*theta))+csc((1/2).*theta).^2.*(q02.*sin(( ...
  1/2).*(1+(-1).*t).*theta)+q12.*sin((1/2).*t.*theta)).*(q04.*sin((1/2).*( ...
  1+(-1).*t).*theta)+q14.*sin((1/2).*t.*theta))).^2+4.*((-1).*csc((1/2).* ...
  theta).^2.*(q01.*sin((1/2).*(1+(-1).*t).*theta)+q11.*sin((1/2).*t.* ...
  theta)).*(q02.*sin((1/2).*(1+(-1).*t).*theta)+q12.*sin((1/2).*t.*theta)) ...
  +csc((1/2).*theta).^2.*(q03.*sin((1/2).*(1+(-1).*t).*theta)+q13.*sin(( ...
  1/2).*t.*theta)).*(q04.*sin((1/2).*(1+(-1).*t).*theta)+q14.*sin((1/2).* ...
  t.*theta))).^2+(1+(-2).*(csc((1/2).*theta).^2.*(q02.*sin((1/2).*(1+(-1) ...
  .*t).*theta)+q12.*sin((1/2).*t.*theta)).^2+csc((1/2).*theta).^2.*(q03.* ...
  sin((1/2).*(1+(-1).*t).*theta)+q13.*sin((1/2).*t.*theta)).^2)).^2).^(-1) ...
  ;
ddth3_des = 0;(-1).*(1+(-2).*(csc((1/2).*theta).^2.*(q03.*sin((1/2).*(1+(-1).*t).* ...
  theta)+q13.*sin((1/2).*t.*theta)).^2+csc((1/2).*theta).^2.*(q04.*sin(( ...
  1/2).*(1+(-1).*t).*theta)+q14.*sin((1/2).*t.*theta)).^2)).*(4.*((-1).* ...
  csc((1/2).*theta).^2.*(q01.*sin((1/2).*(1+(-1).*t).*theta)+q11.*sin(( ...
  1/2).*t.*theta)).*(q02.*sin((1/2).*(1+(-1).*t).*theta)+q12.*sin((1/2).* ...
  t.*theta))+csc((1/2).*theta).^2.*(q03.*sin((1/2).*(1+(-1).*t).*theta)+ ...
  q13.*sin((1/2).*t.*theta)).*(q04.*sin((1/2).*(1+(-1).*t).*theta)+q14.* ...
  sin((1/2).*t.*theta))).^2+(1+(-2).*(csc((1/2).*theta).^2.*(q02.*sin(( ...
  1/2).*(1+(-1).*t).*theta)+q12.*sin((1/2).*t.*theta)).^2+csc((1/2).* ...
  theta).^2.*(q03.*sin((1/2).*(1+(-1).*t).*theta)+q13.*sin((1/2).*t.* ...
  theta)).^2)).^2).^(-1/2).*(4.*(csc((1/2).*theta).^2.*(q01.*sin((1/2).*( ...
  1+(-1).*t).*theta)+q11.*sin((1/2).*t.*theta)).*(q03.*sin((1/2).*(1+(-1) ...
  .*t).*theta)+q13.*sin((1/2).*t.*theta))+csc((1/2).*theta).^2.*(q02.*sin( ...
  (1/2).*(1+(-1).*t).*theta)+q12.*sin((1/2).*t.*theta)).*(q04.*sin((1/2).* ...
  (1+(-1).*t).*theta)+q14.*sin((1/2).*t.*theta))).^2+4.*((-1).*csc((1/2).* ...
  theta).^2.*(q01.*sin((1/2).*(1+(-1).*t).*theta)+q11.*sin((1/2).*t.* ...
  theta)).*(q02.*sin((1/2).*(1+(-1).*t).*theta)+q12.*sin((1/2).*t.*theta)) ...
  +csc((1/2).*theta).^2.*(q03.*sin((1/2).*(1+(-1).*t).*theta)+q13.*sin(( ...
  1/2).*t.*theta)).*(q04.*sin((1/2).*(1+(-1).*t).*theta)+q14.*sin((1/2).* ...
  t.*theta))).^2+(1+(-2).*(csc((1/2).*theta).^2.*(q02.*sin((1/2).*(1+(-1) ...
  .*t).*theta)+q12.*sin((1/2).*t.*theta)).^2+csc((1/2).*theta).^2.*(q03.* ...
  sin((1/2).*(1+(-1).*t).*theta)+q13.*sin((1/2).*t.*theta)).^2)).^2).^( ...
  1/2).*((-1).*(csc((1/2).*theta).^2.*(q02.*sin((1/2).*(1+(-1).*t).*theta) ...
  +q12.*sin((1/2).*t.*theta)).*(q03.*sin((1/2).*(1+(-1).*t).*theta)+q13.* ...
  sin((1/2).*t.*theta))+(-1).*csc((1/2).*theta).^2.*(q01.*sin((1/2).*(1+( ...
  -1).*t).*theta)+q11.*sin((1/2).*t.*theta)).*(q04.*sin((1/2).*(1+(-1).*t) ...
  .*theta)+q14.*sin((1/2).*t.*theta))).*(8.*(((-1/2).*q03.*theta.*cos(( ...
  1/2).*(1+(-1).*t).*theta)+(1/2).*q13.*theta.*cos((1/2).*t.*theta)).*csc( ...
  (1/2).*theta).^2.*(q01.*sin((1/2).*(1+(-1).*t).*theta)+q11.*sin((1/2).* ...
  t.*theta))+((-1/2).*q04.*theta.*cos((1/2).*(1+(-1).*t).*theta)+(1/2).* ...
  q14.*theta.*cos((1/2).*t.*theta)).*csc((1/2).*theta).^2.*(q02.*sin((1/2) ...
  .*(1+(-1).*t).*theta)+q12.*sin((1/2).*t.*theta))+((-1/2).*q01.*theta.* ...
  cos((1/2).*(1+(-1).*t).*theta)+(1/2).*q11.*theta.*cos((1/2).*t.*theta)) ...
  .*csc((1/2).*theta).^2.*(q03.*sin((1/2).*(1+(-1).*t).*theta)+q13.*sin(( ...
  1/2).*t.*theta))+((-1/2).*q02.*theta.*cos((1/2).*(1+(-1).*t).*theta)+( ...
  1/2).*q12.*theta.*cos((1/2).*t.*theta)).*csc((1/2).*theta).^2.*(q04.* ...
  sin((1/2).*(1+(-1).*t).*theta)+q14.*sin((1/2).*t.*theta))).*(csc((1/2).* ...
  theta).^2.*(q01.*sin((1/2).*(1+(-1).*t).*theta)+q11.*sin((1/2).*t.* ...
  theta)).*(q03.*sin((1/2).*(1+(-1).*t).*theta)+q13.*sin((1/2).*t.*theta)) ...
  +csc((1/2).*theta).^2.*(q02.*sin((1/2).*(1+(-1).*t).*theta)+q12.*sin(( ...
  1/2).*t.*theta)).*(q04.*sin((1/2).*(1+(-1).*t).*theta)+q14.*sin((1/2).* ...
  t.*theta)))+8.*((-1).*((-1/2).*q02.*theta.*cos((1/2).*(1+(-1).*t).* ...
  theta)+(1/2).*q12.*theta.*cos((1/2).*t.*theta)).*csc((1/2).*theta).^2.*( ...
  q01.*sin((1/2).*(1+(-1).*t).*theta)+q11.*sin((1/2).*t.*theta))+(-1).*(( ...
  -1/2).*q01.*theta.*cos((1/2).*(1+(-1).*t).*theta)+(1/2).*q11.*theta.* ...
  cos((1/2).*t.*theta)).*csc((1/2).*theta).^2.*(q02.*sin((1/2).*(1+(-1).* ...
  t).*theta)+q12.*sin((1/2).*t.*theta))+((-1/2).*q04.*theta.*cos((1/2).*( ...
  1+(-1).*t).*theta)+(1/2).*q14.*theta.*cos((1/2).*t.*theta)).*csc((1/2).* ...
  theta).^2.*(q03.*sin((1/2).*(1+(-1).*t).*theta)+q13.*sin((1/2).*t.* ...
  theta))+((-1/2).*q03.*theta.*cos((1/2).*(1+(-1).*t).*theta)+(1/2).*q13.* ...
  theta.*cos((1/2).*t.*theta)).*csc((1/2).*theta).^2.*(q04.*sin((1/2).*(1+ ...
  (-1).*t).*theta)+q14.*sin((1/2).*t.*theta))).*((-1).*csc((1/2).*theta) ...
  .^2.*(q01.*sin((1/2).*(1+(-1).*t).*theta)+q11.*sin((1/2).*t.*theta)).*( ...
  q02.*sin((1/2).*(1+(-1).*t).*theta)+q12.*sin((1/2).*t.*theta))+csc((1/2) ...
  .*theta).^2.*(q03.*sin((1/2).*(1+(-1).*t).*theta)+q13.*sin((1/2).*t.* ...
  theta)).*(q04.*sin((1/2).*(1+(-1).*t).*theta)+q14.*sin((1/2).*t.*theta)) ...
  )+(-4).*(2.*((-1/2).*q02.*theta.*cos((1/2).*(1+(-1).*t).*theta)+(1/2).* ...
  q12.*theta.*cos((1/2).*t.*theta)).*csc((1/2).*theta).^2.*(q02.*sin((1/2) ...
  .*(1+(-1).*t).*theta)+q12.*sin((1/2).*t.*theta))+2.*((-1/2).*q03.* ...
  theta.*cos((1/2).*(1+(-1).*t).*theta)+(1/2).*q13.*theta.*cos((1/2).*t.* ...
  theta)).*csc((1/2).*theta).^2.*(q03.*sin((1/2).*(1+(-1).*t).*theta)+ ...
  q13.*sin((1/2).*t.*theta))).*(1+(-2).*(csc((1/2).*theta).^2.*(q02.*sin(( ...
  1/2).*(1+(-1).*t).*theta)+q12.*sin((1/2).*t.*theta)).^2+csc((1/2).* ...
  theta).^2.*(q03.*sin((1/2).*(1+(-1).*t).*theta)+q13.*sin((1/2).*t.* ...
  theta)).^2))).*(4.*((-1).*csc((1/2).*theta).^2.*(q01.*sin((1/2).*(1+(-1) ...
  .*t).*theta)+q11.*sin((1/2).*t.*theta)).*(q02.*sin((1/2).*(1+(-1).*t).* ...
  theta)+q12.*sin((1/2).*t.*theta))+csc((1/2).*theta).^2.*(q03.*sin((1/2) ...
  .*(1+(-1).*t).*theta)+q13.*sin((1/2).*t.*theta)).*(q04.*sin((1/2).*(1+( ...
  -1).*t).*theta)+q14.*sin((1/2).*t.*theta))).^2+(1+(-2).*(csc((1/2).* ...
  theta).^2.*(q02.*sin((1/2).*(1+(-1).*t).*theta)+q12.*sin((1/2).*t.* ...
  theta)).^2+csc((1/2).*theta).^2.*(q03.*sin((1/2).*(1+(-1).*t).*theta)+ ...
  q13.*sin((1/2).*t.*theta)).^2)).^2).^(-1/2).*(4.*(csc((1/2).*theta).^2.* ...
  (q01.*sin((1/2).*(1+(-1).*t).*theta)+q11.*sin((1/2).*t.*theta)).*(q03.* ...
  sin((1/2).*(1+(-1).*t).*theta)+q13.*sin((1/2).*t.*theta))+csc((1/2).* ...
  theta).^2.*(q02.*sin((1/2).*(1+(-1).*t).*theta)+q12.*sin((1/2).*t.* ...
  theta)).*(q04.*sin((1/2).*(1+(-1).*t).*theta)+q14.*sin((1/2).*t.*theta)) ...
  ).^2+4.*((-1).*csc((1/2).*theta).^2.*(q01.*sin((1/2).*(1+(-1).*t).* ...
  theta)+q11.*sin((1/2).*t.*theta)).*(q02.*sin((1/2).*(1+(-1).*t).*theta)+ ...
  q12.*sin((1/2).*t.*theta))+csc((1/2).*theta).^2.*(q03.*sin((1/2).*(1+( ...
  -1).*t).*theta)+q13.*sin((1/2).*t.*theta)).*(q04.*sin((1/2).*(1+(-1).*t) ...
  .*theta)+q14.*sin((1/2).*t.*theta))).^2+(1+(-2).*(csc((1/2).*theta).^2.* ...
  (q02.*sin((1/2).*(1+(-1).*t).*theta)+q12.*sin((1/2).*t.*theta)).^2+csc(( ...
  1/2).*theta).^2.*(q03.*sin((1/2).*(1+(-1).*t).*theta)+q13.*sin((1/2).* ...
  t.*theta)).^2)).^2).^(-1/2)+(csc((1/2).*theta).^2.*(q02.*sin((1/2).*(1+( ...
  -1).*t).*theta)+q12.*sin((1/2).*t.*theta)).*(q03.*sin((1/2).*(1+(-1).*t) ...
  .*theta)+q13.*sin((1/2).*t.*theta))+(-1).*csc((1/2).*theta).^2.*(q01.* ...
  sin((1/2).*(1+(-1).*t).*theta)+q11.*sin((1/2).*t.*theta)).*(q04.*sin(( ...
  1/2).*(1+(-1).*t).*theta)+q14.*sin((1/2).*t.*theta))).*(8.*((-1).*(( ...
  -1/2).*q02.*theta.*cos((1/2).*(1+(-1).*t).*theta)+(1/2).*q12.*theta.* ...
  cos((1/2).*t.*theta)).*csc((1/2).*theta).^2.*(q01.*sin((1/2).*(1+(-1).* ...
  t).*theta)+q11.*sin((1/2).*t.*theta))+(-1).*((-1/2).*q01.*theta.*cos(( ...
  1/2).*(1+(-1).*t).*theta)+(1/2).*q11.*theta.*cos((1/2).*t.*theta)).*csc( ...
  (1/2).*theta).^2.*(q02.*sin((1/2).*(1+(-1).*t).*theta)+q12.*sin((1/2).* ...
  t.*theta))+((-1/2).*q04.*theta.*cos((1/2).*(1+(-1).*t).*theta)+(1/2).* ...
  q14.*theta.*cos((1/2).*t.*theta)).*csc((1/2).*theta).^2.*(q03.*sin((1/2) ...
  .*(1+(-1).*t).*theta)+q13.*sin((1/2).*t.*theta))+((-1/2).*q03.*theta.* ...
  cos((1/2).*(1+(-1).*t).*theta)+(1/2).*q13.*theta.*cos((1/2).*t.*theta)) ...
  .*csc((1/2).*theta).^2.*(q04.*sin((1/2).*(1+(-1).*t).*theta)+q14.*sin(( ...
  1/2).*t.*theta))).*((-1).*csc((1/2).*theta).^2.*(q01.*sin((1/2).*(1+(-1) ...
  .*t).*theta)+q11.*sin((1/2).*t.*theta)).*(q02.*sin((1/2).*(1+(-1).*t).* ...
  theta)+q12.*sin((1/2).*t.*theta))+csc((1/2).*theta).^2.*(q03.*sin((1/2) ...
  .*(1+(-1).*t).*theta)+q13.*sin((1/2).*t.*theta)).*(q04.*sin((1/2).*(1+( ...
  -1).*t).*theta)+q14.*sin((1/2).*t.*theta)))+(-4).*(2.*((-1/2).*q02.* ...
  theta.*cos((1/2).*(1+(-1).*t).*theta)+(1/2).*q12.*theta.*cos((1/2).*t.* ...
  theta)).*csc((1/2).*theta).^2.*(q02.*sin((1/2).*(1+(-1).*t).*theta)+ ...
  q12.*sin((1/2).*t.*theta))+2.*((-1/2).*q03.*theta.*cos((1/2).*(1+(-1).* ...
  t).*theta)+(1/2).*q13.*theta.*cos((1/2).*t.*theta)).*csc((1/2).*theta) ...
  .^2.*(q03.*sin((1/2).*(1+(-1).*t).*theta)+q13.*sin((1/2).*t.*theta))).*( ...
  1+(-2).*(csc((1/2).*theta).^2.*(q02.*sin((1/2).*(1+(-1).*t).*theta)+ ...
  q12.*sin((1/2).*t.*theta)).^2+csc((1/2).*theta).^2.*(q03.*sin((1/2).*(1+ ...
  (-1).*t).*theta)+q13.*sin((1/2).*t.*theta)).^2))).*(4.*((-1).*csc((1/2) ...
  .*theta).^2.*(q01.*sin((1/2).*(1+(-1).*t).*theta)+q11.*sin((1/2).*t.* ...
  theta)).*(q02.*sin((1/2).*(1+(-1).*t).*theta)+q12.*sin((1/2).*t.*theta)) ...
  +csc((1/2).*theta).^2.*(q03.*sin((1/2).*(1+(-1).*t).*theta)+q13.*sin(( ...
  1/2).*t.*theta)).*(q04.*sin((1/2).*(1+(-1).*t).*theta)+q14.*sin((1/2).* ...
  t.*theta))).^2+(1+(-2).*(csc((1/2).*theta).^2.*(q02.*sin((1/2).*(1+(-1) ...
  .*t).*theta)+q12.*sin((1/2).*t.*theta)).^2+csc((1/2).*theta).^2.*(q03.* ...
  sin((1/2).*(1+(-1).*t).*theta)+q13.*sin((1/2).*t.*theta)).^2)).^2).^( ...
  -3/2).*(4.*(csc((1/2).*theta).^2.*(q01.*sin((1/2).*(1+(-1).*t).*theta)+ ...
  q11.*sin((1/2).*t.*theta)).*(q03.*sin((1/2).*(1+(-1).*t).*theta)+q13.* ...
  sin((1/2).*t.*theta))+csc((1/2).*theta).^2.*(q02.*sin((1/2).*(1+(-1).*t) ...
  .*theta)+q12.*sin((1/2).*t.*theta)).*(q04.*sin((1/2).*(1+(-1).*t).* ...
  theta)+q14.*sin((1/2).*t.*theta))).^2+4.*((-1).*csc((1/2).*theta).^2.*( ...
  q01.*sin((1/2).*(1+(-1).*t).*theta)+q11.*sin((1/2).*t.*theta)).*(q02.* ...
  sin((1/2).*(1+(-1).*t).*theta)+q12.*sin((1/2).*t.*theta))+csc((1/2).* ...
  theta).^2.*(q03.*sin((1/2).*(1+(-1).*t).*theta)+q13.*sin((1/2).*t.* ...
  theta)).*(q04.*sin((1/2).*(1+(-1).*t).*theta)+q14.*sin((1/2).*t.*theta)) ...
  ).^2+(1+(-2).*(csc((1/2).*theta).^2.*(q02.*sin((1/2).*(1+(-1).*t).* ...
  theta)+q12.*sin((1/2).*t.*theta)).^2+csc((1/2).*theta).^2.*(q03.*sin(( ...
  1/2).*(1+(-1).*t).*theta)+q13.*sin((1/2).*t.*theta)).^2)).^2).^(1/2)+( ...
  -2).*((-1).*((-1/2).*q04.*theta.*cos((1/2).*(1+(-1).*t).*theta)+(1/2).* ...
  q14.*theta.*cos((1/2).*t.*theta)).*csc((1/2).*theta).^2.*(q01.*sin((1/2) ...
  .*(1+(-1).*t).*theta)+q11.*sin((1/2).*t.*theta))+((-1/2).*q03.*theta.* ...
  cos((1/2).*(1+(-1).*t).*theta)+(1/2).*q13.*theta.*cos((1/2).*t.*theta)) ...
  .*csc((1/2).*theta).^2.*(q02.*sin((1/2).*(1+(-1).*t).*theta)+q12.*sin(( ...
  1/2).*t.*theta))+((-1/2).*q02.*theta.*cos((1/2).*(1+(-1).*t).*theta)+( ...
  1/2).*q12.*theta.*cos((1/2).*t.*theta)).*csc((1/2).*theta).^2.*(q03.* ...
  sin((1/2).*(1+(-1).*t).*theta)+q13.*sin((1/2).*t.*theta))+(-1).*((-1/2) ...
  .*q01.*theta.*cos((1/2).*(1+(-1).*t).*theta)+(1/2).*q11.*theta.*cos(( ...
  1/2).*t.*theta)).*csc((1/2).*theta).^2.*(q04.*sin((1/2).*(1+(-1).*t).* ...
  theta)+q14.*sin((1/2).*t.*theta))).*(4.*((-1).*csc((1/2).*theta).^2.*( ...
  q01.*sin((1/2).*(1+(-1).*t).*theta)+q11.*sin((1/2).*t.*theta)).*(q02.* ...
  sin((1/2).*(1+(-1).*t).*theta)+q12.*sin((1/2).*t.*theta))+csc((1/2).* ...
  theta).^2.*(q03.*sin((1/2).*(1+(-1).*t).*theta)+q13.*sin((1/2).*t.* ...
  theta)).*(q04.*sin((1/2).*(1+(-1).*t).*theta)+q14.*sin((1/2).*t.*theta)) ...
  ).^2+(1+(-2).*(csc((1/2).*theta).^2.*(q02.*sin((1/2).*(1+(-1).*t).* ...
  theta)+q12.*sin((1/2).*t.*theta)).^2+csc((1/2).*theta).^2.*(q03.*sin(( ...
  1/2).*(1+(-1).*t).*theta)+q13.*sin((1/2).*t.*theta)).^2)).^2).^(-1/2).*( ...
  4.*(csc((1/2).*theta).^2.*(q01.*sin((1/2).*(1+(-1).*t).*theta)+q11.*sin( ...
  (1/2).*t.*theta)).*(q03.*sin((1/2).*(1+(-1).*t).*theta)+q13.*sin((1/2).* ...
  t.*theta))+csc((1/2).*theta).^2.*(q02.*sin((1/2).*(1+(-1).*t).*theta)+ ...
  q12.*sin((1/2).*t.*theta)).*(q04.*sin((1/2).*(1+(-1).*t).*theta)+q14.* ...
  sin((1/2).*t.*theta))).^2+4.*((-1).*csc((1/2).*theta).^2.*(q01.*sin(( ...
  1/2).*(1+(-1).*t).*theta)+q11.*sin((1/2).*t.*theta)).*(q02.*sin((1/2).*( ...
  1+(-1).*t).*theta)+q12.*sin((1/2).*t.*theta))+csc((1/2).*theta).^2.*( ...
  q03.*sin((1/2).*(1+(-1).*t).*theta)+q13.*sin((1/2).*t.*theta)).*(q04.* ...
  sin((1/2).*(1+(-1).*t).*theta)+q14.*sin((1/2).*t.*theta))).^2+(1+(-2).*( ...
  csc((1/2).*theta).^2.*(q02.*sin((1/2).*(1+(-1).*t).*theta)+q12.*sin(( ...
  1/2).*t.*theta)).^2+csc((1/2).*theta).^2.*(q03.*sin((1/2).*(1+(-1).*t).* ...
  theta)+q13.*sin((1/2).*t.*theta)).^2)).^2).^(1/2)).*(4.*(csc((1/2).* ...
  theta).^2.*(q02.*sin((1/2).*(1+(-1).*t).*theta)+q12.*sin((1/2).*t.* ...
  theta)).*(q03.*sin((1/2).*(1+(-1).*t).*theta)+q13.*sin((1/2).*t.*theta)) ...
  +(-1).*csc((1/2).*theta).^2.*(q01.*sin((1/2).*(1+(-1).*t).*theta)+q11.* ...
  sin((1/2).*t.*theta)).*(q04.*sin((1/2).*(1+(-1).*t).*theta)+q14.*sin(( ...
  1/2).*t.*theta))).^2.*(8.*(((-1/2).*q03.*theta.*cos((1/2).*(1+(-1).*t).* ...
  theta)+(1/2).*q13.*theta.*cos((1/2).*t.*theta)).*csc((1/2).*theta).^2.*( ...
  q01.*sin((1/2).*(1+(-1).*t).*theta)+q11.*sin((1/2).*t.*theta))+((-1/2).* ...
  q04.*theta.*cos((1/2).*(1+(-1).*t).*theta)+(1/2).*q14.*theta.*cos((1/2) ...
  .*t.*theta)).*csc((1/2).*theta).^2.*(q02.*sin((1/2).*(1+(-1).*t).*theta) ...
  +q12.*sin((1/2).*t.*theta))+((-1/2).*q01.*theta.*cos((1/2).*(1+(-1).*t) ...
  .*theta)+(1/2).*q11.*theta.*cos((1/2).*t.*theta)).*csc((1/2).*theta) ...
  .^2.*(q03.*sin((1/2).*(1+(-1).*t).*theta)+q13.*sin((1/2).*t.*theta))+(( ...
  -1/2).*q02.*theta.*cos((1/2).*(1+(-1).*t).*theta)+(1/2).*q12.*theta.* ...
  cos((1/2).*t.*theta)).*csc((1/2).*theta).^2.*(q04.*sin((1/2).*(1+(-1).* ...
  t).*theta)+q14.*sin((1/2).*t.*theta))).*(csc((1/2).*theta).^2.*(q01.* ...
  sin((1/2).*(1+(-1).*t).*theta)+q11.*sin((1/2).*t.*theta)).*(q03.*sin(( ...
  1/2).*(1+(-1).*t).*theta)+q13.*sin((1/2).*t.*theta))+csc((1/2).*theta) ...
  .^2.*(q02.*sin((1/2).*(1+(-1).*t).*theta)+q12.*sin((1/2).*t.*theta)).*( ...
  q04.*sin((1/2).*(1+(-1).*t).*theta)+q14.*sin((1/2).*t.*theta)))+8.*((-1) ...
  .*((-1/2).*q02.*theta.*cos((1/2).*(1+(-1).*t).*theta)+(1/2).*q12.* ...
  theta.*cos((1/2).*t.*theta)).*csc((1/2).*theta).^2.*(q01.*sin((1/2).*(1+ ...
  (-1).*t).*theta)+q11.*sin((1/2).*t.*theta))+(-1).*((-1/2).*q01.*theta.* ...
  cos((1/2).*(1+(-1).*t).*theta)+(1/2).*q11.*theta.*cos((1/2).*t.*theta)) ...
  .*csc((1/2).*theta).^2.*(q02.*sin((1/2).*(1+(-1).*t).*theta)+q12.*sin(( ...
  1/2).*t.*theta))+((-1/2).*q04.*theta.*cos((1/2).*(1+(-1).*t).*theta)+( ...
  1/2).*q14.*theta.*cos((1/2).*t.*theta)).*csc((1/2).*theta).^2.*(q03.* ...
  sin((1/2).*(1+(-1).*t).*theta)+q13.*sin((1/2).*t.*theta))+((-1/2).*q03.* ...
  theta.*cos((1/2).*(1+(-1).*t).*theta)+(1/2).*q13.*theta.*cos((1/2).*t.* ...
  theta)).*csc((1/2).*theta).^2.*(q04.*sin((1/2).*(1+(-1).*t).*theta)+ ...
  q14.*sin((1/2).*t.*theta))).*((-1).*csc((1/2).*theta).^2.*(q01.*sin(( ...
  1/2).*(1+(-1).*t).*theta)+q11.*sin((1/2).*t.*theta)).*(q02.*sin((1/2).*( ...
  1+(-1).*t).*theta)+q12.*sin((1/2).*t.*theta))+csc((1/2).*theta).^2.*( ...
  q03.*sin((1/2).*(1+(-1).*t).*theta)+q13.*sin((1/2).*t.*theta)).*(q04.* ...
  sin((1/2).*(1+(-1).*t).*theta)+q14.*sin((1/2).*t.*theta)))+(-4).*(2.*(( ...
  -1/2).*q02.*theta.*cos((1/2).*(1+(-1).*t).*theta)+(1/2).*q12.*theta.* ...
  cos((1/2).*t.*theta)).*csc((1/2).*theta).^2.*(q02.*sin((1/2).*(1+(-1).* ...
  t).*theta)+q12.*sin((1/2).*t.*theta))+2.*((-1/2).*q03.*theta.*cos((1/2) ...
  .*(1+(-1).*t).*theta)+(1/2).*q13.*theta.*cos((1/2).*t.*theta)).*csc(( ...
  1/2).*theta).^2.*(q03.*sin((1/2).*(1+(-1).*t).*theta)+q13.*sin((1/2).* ...
  t.*theta))).*(1+(-2).*(csc((1/2).*theta).^2.*(q02.*sin((1/2).*(1+(-1).* ...
  t).*theta)+q12.*sin((1/2).*t.*theta)).^2+csc((1/2).*theta).^2.*(q03.* ...
  sin((1/2).*(1+(-1).*t).*theta)+q13.*sin((1/2).*t.*theta)).^2))).*(4.*(( ...
  -1).*csc((1/2).*theta).^2.*(q01.*sin((1/2).*(1+(-1).*t).*theta)+q11.* ...
  sin((1/2).*t.*theta)).*(q02.*sin((1/2).*(1+(-1).*t).*theta)+q12.*sin(( ...
  1/2).*t.*theta))+csc((1/2).*theta).^2.*(q03.*sin((1/2).*(1+(-1).*t).* ...
  theta)+q13.*sin((1/2).*t.*theta)).*(q04.*sin((1/2).*(1+(-1).*t).*theta)+ ...
  q14.*sin((1/2).*t.*theta))).^2+(1+(-2).*(csc((1/2).*theta).^2.*(q02.* ...
  sin((1/2).*(1+(-1).*t).*theta)+q12.*sin((1/2).*t.*theta)).^2+csc((1/2).* ...
  theta).^2.*(q03.*sin((1/2).*(1+(-1).*t).*theta)+q13.*sin((1/2).*t.* ...
  theta)).^2)).^2).^(-1)+(1+(-2).*(csc((1/2).*theta).^2.*(q03.*sin((1/2).* ...
  (1+(-1).*t).*theta)+q13.*sin((1/2).*t.*theta)).^2+csc((1/2).*theta).^2.* ...
  (q04.*sin((1/2).*(1+(-1).*t).*theta)+q14.*sin((1/2).*t.*theta)).^2)) ...
  .^2.*(8.*(((-1/2).*q03.*theta.*cos((1/2).*(1+(-1).*t).*theta)+(1/2).* ...
  q13.*theta.*cos((1/2).*t.*theta)).*csc((1/2).*theta).^2.*(q01.*sin((1/2) ...
  .*(1+(-1).*t).*theta)+q11.*sin((1/2).*t.*theta))+((-1/2).*q04.*theta.* ...
  cos((1/2).*(1+(-1).*t).*theta)+(1/2).*q14.*theta.*cos((1/2).*t.*theta)) ...
  .*csc((1/2).*theta).^2.*(q02.*sin((1/2).*(1+(-1).*t).*theta)+q12.*sin(( ...
  1/2).*t.*theta))+((-1/2).*q01.*theta.*cos((1/2).*(1+(-1).*t).*theta)+( ...
  1/2).*q11.*theta.*cos((1/2).*t.*theta)).*csc((1/2).*theta).^2.*(q03.* ...
  sin((1/2).*(1+(-1).*t).*theta)+q13.*sin((1/2).*t.*theta))+((-1/2).*q02.* ...
  theta.*cos((1/2).*(1+(-1).*t).*theta)+(1/2).*q12.*theta.*cos((1/2).*t.* ...
  theta)).*csc((1/2).*theta).^2.*(q04.*sin((1/2).*(1+(-1).*t).*theta)+ ...
  q14.*sin((1/2).*t.*theta))).*(csc((1/2).*theta).^2.*(q01.*sin((1/2).*(1+ ...
  (-1).*t).*theta)+q11.*sin((1/2).*t.*theta)).*(q03.*sin((1/2).*(1+(-1).* ...
  t).*theta)+q13.*sin((1/2).*t.*theta))+csc((1/2).*theta).^2.*(q02.*sin(( ...
  1/2).*(1+(-1).*t).*theta)+q12.*sin((1/2).*t.*theta)).*(q04.*sin((1/2).*( ...
  1+(-1).*t).*theta)+q14.*sin((1/2).*t.*theta)))+8.*((-1).*((-1/2).*q02.* ...
  theta.*cos((1/2).*(1+(-1).*t).*theta)+(1/2).*q12.*theta.*cos((1/2).*t.* ...
  theta)).*csc((1/2).*theta).^2.*(q01.*sin((1/2).*(1+(-1).*t).*theta)+ ...
  q11.*sin((1/2).*t.*theta))+(-1).*((-1/2).*q01.*theta.*cos((1/2).*(1+(-1) ...
  .*t).*theta)+(1/2).*q11.*theta.*cos((1/2).*t.*theta)).*csc((1/2).*theta) ...
  .^2.*(q02.*sin((1/2).*(1+(-1).*t).*theta)+q12.*sin((1/2).*t.*theta))+(( ...
  -1/2).*q04.*theta.*cos((1/2).*(1+(-1).*t).*theta)+(1/2).*q14.*theta.* ...
  cos((1/2).*t.*theta)).*csc((1/2).*theta).^2.*(q03.*sin((1/2).*(1+(-1).* ...
  t).*theta)+q13.*sin((1/2).*t.*theta))+((-1/2).*q03.*theta.*cos((1/2).*( ...
  1+(-1).*t).*theta)+(1/2).*q13.*theta.*cos((1/2).*t.*theta)).*csc((1/2).* ...
  theta).^2.*(q04.*sin((1/2).*(1+(-1).*t).*theta)+q14.*sin((1/2).*t.* ...
  theta))).*((-1).*csc((1/2).*theta).^2.*(q01.*sin((1/2).*(1+(-1).*t).* ...
  theta)+q11.*sin((1/2).*t.*theta)).*(q02.*sin((1/2).*(1+(-1).*t).*theta)+ ...
  q12.*sin((1/2).*t.*theta))+csc((1/2).*theta).^2.*(q03.*sin((1/2).*(1+( ...
  -1).*t).*theta)+q13.*sin((1/2).*t.*theta)).*(q04.*sin((1/2).*(1+(-1).*t) ...
  .*theta)+q14.*sin((1/2).*t.*theta)))+(-4).*(2.*((-1/2).*q02.*theta.*cos( ...
  (1/2).*(1+(-1).*t).*theta)+(1/2).*q12.*theta.*cos((1/2).*t.*theta)).* ...
  csc((1/2).*theta).^2.*(q02.*sin((1/2).*(1+(-1).*t).*theta)+q12.*sin(( ...
  1/2).*t.*theta))+2.*((-1/2).*q03.*theta.*cos((1/2).*(1+(-1).*t).*theta)+ ...
  (1/2).*q13.*theta.*cos((1/2).*t.*theta)).*csc((1/2).*theta).^2.*(q03.* ...
  sin((1/2).*(1+(-1).*t).*theta)+q13.*sin((1/2).*t.*theta))).*(1+(-2).*( ...
  csc((1/2).*theta).^2.*(q02.*sin((1/2).*(1+(-1).*t).*theta)+q12.*sin(( ...
  1/2).*t.*theta)).^2+csc((1/2).*theta).^2.*(q03.*sin((1/2).*(1+(-1).*t).* ...
  theta)+q13.*sin((1/2).*t.*theta)).^2))).*(4.*((-1).*csc((1/2).*theta) ...
  .^2.*(q01.*sin((1/2).*(1+(-1).*t).*theta)+q11.*sin((1/2).*t.*theta)).*( ...
  q02.*sin((1/2).*(1+(-1).*t).*theta)+q12.*sin((1/2).*t.*theta))+csc((1/2) ...
  .*theta).^2.*(q03.*sin((1/2).*(1+(-1).*t).*theta)+q13.*sin((1/2).*t.* ...
  theta)).*(q04.*sin((1/2).*(1+(-1).*t).*theta)+q14.*sin((1/2).*t.*theta)) ...
  ).^2+(1+(-2).*(csc((1/2).*theta).^2.*(q02.*sin((1/2).*(1+(-1).*t).* ...
  theta)+q12.*sin((1/2).*t.*theta)).^2+csc((1/2).*theta).^2.*(q03.*sin(( ...
  1/2).*(1+(-1).*t).*theta)+q13.*sin((1/2).*t.*theta)).^2)).^2).^(-1)+(-4) ...
  .*(csc((1/2).*theta).^2.*(q02.*sin((1/2).*(1+(-1).*t).*theta)+q12.*sin(( ...
  1/2).*t.*theta)).*(q03.*sin((1/2).*(1+(-1).*t).*theta)+q13.*sin((1/2).* ...
  t.*theta))+(-1).*csc((1/2).*theta).^2.*(q01.*sin((1/2).*(1+(-1).*t).* ...
  theta)+q11.*sin((1/2).*t.*theta)).*(q04.*sin((1/2).*(1+(-1).*t).*theta)+ ...
  q14.*sin((1/2).*t.*theta))).^2.*(8.*((-1).*((-1/2).*q02.*theta.*cos(( ...
  1/2).*(1+(-1).*t).*theta)+(1/2).*q12.*theta.*cos((1/2).*t.*theta)).*csc( ...
  (1/2).*theta).^2.*(q01.*sin((1/2).*(1+(-1).*t).*theta)+q11.*sin((1/2).* ...
  t.*theta))+(-1).*((-1/2).*q01.*theta.*cos((1/2).*(1+(-1).*t).*theta)+( ...
  1/2).*q11.*theta.*cos((1/2).*t.*theta)).*csc((1/2).*theta).^2.*(q02.* ...
  sin((1/2).*(1+(-1).*t).*theta)+q12.*sin((1/2).*t.*theta))+((-1/2).*q04.* ...
  theta.*cos((1/2).*(1+(-1).*t).*theta)+(1/2).*q14.*theta.*cos((1/2).*t.* ...
  theta)).*csc((1/2).*theta).^2.*(q03.*sin((1/2).*(1+(-1).*t).*theta)+ ...
  q13.*sin((1/2).*t.*theta))+((-1/2).*q03.*theta.*cos((1/2).*(1+(-1).*t).* ...
  theta)+(1/2).*q13.*theta.*cos((1/2).*t.*theta)).*csc((1/2).*theta).^2.*( ...
  q04.*sin((1/2).*(1+(-1).*t).*theta)+q14.*sin((1/2).*t.*theta))).*((-1).* ...
  csc((1/2).*theta).^2.*(q01.*sin((1/2).*(1+(-1).*t).*theta)+q11.*sin(( ...
  1/2).*t.*theta)).*(q02.*sin((1/2).*(1+(-1).*t).*theta)+q12.*sin((1/2).* ...
  t.*theta))+csc((1/2).*theta).^2.*(q03.*sin((1/2).*(1+(-1).*t).*theta)+ ...
  q13.*sin((1/2).*t.*theta)).*(q04.*sin((1/2).*(1+(-1).*t).*theta)+q14.* ...
  sin((1/2).*t.*theta)))+(-4).*(2.*((-1/2).*q02.*theta.*cos((1/2).*(1+(-1) ...
  .*t).*theta)+(1/2).*q12.*theta.*cos((1/2).*t.*theta)).*csc((1/2).*theta) ...
  .^2.*(q02.*sin((1/2).*(1+(-1).*t).*theta)+q12.*sin((1/2).*t.*theta))+2.* ...
  ((-1/2).*q03.*theta.*cos((1/2).*(1+(-1).*t).*theta)+(1/2).*q13.*theta.* ...
  cos((1/2).*t.*theta)).*csc((1/2).*theta).^2.*(q03.*sin((1/2).*(1+(-1).* ...
  t).*theta)+q13.*sin((1/2).*t.*theta))).*(1+(-2).*(csc((1/2).*theta).^2.* ...
  (q02.*sin((1/2).*(1+(-1).*t).*theta)+q12.*sin((1/2).*t.*theta)).^2+csc(( ...
  1/2).*theta).^2.*(q03.*sin((1/2).*(1+(-1).*t).*theta)+q13.*sin((1/2).* ...
  t.*theta)).^2))).*(4.*((-1).*csc((1/2).*theta).^2.*(q01.*sin((1/2).*(1+( ...
  -1).*t).*theta)+q11.*sin((1/2).*t.*theta)).*(q02.*sin((1/2).*(1+(-1).*t) ...
  .*theta)+q12.*sin((1/2).*t.*theta))+csc((1/2).*theta).^2.*(q03.*sin(( ...
  1/2).*(1+(-1).*t).*theta)+q13.*sin((1/2).*t.*theta)).*(q04.*sin((1/2).*( ...
  1+(-1).*t).*theta)+q14.*sin((1/2).*t.*theta))).^2+(1+(-2).*(csc((1/2).* ...
  theta).^2.*(q02.*sin((1/2).*(1+(-1).*t).*theta)+q12.*sin((1/2).*t.* ...
  theta)).^2+csc((1/2).*theta).^2.*(q03.*sin((1/2).*(1+(-1).*t).*theta)+ ...
  q13.*sin((1/2).*t.*theta)).^2)).^2).^(-2).*(4.*(csc((1/2).*theta).^2.*( ...
  q01.*sin((1/2).*(1+(-1).*t).*theta)+q11.*sin((1/2).*t.*theta)).*(q03.* ...
  sin((1/2).*(1+(-1).*t).*theta)+q13.*sin((1/2).*t.*theta))+csc((1/2).* ...
  theta).^2.*(q02.*sin((1/2).*(1+(-1).*t).*theta)+q12.*sin((1/2).*t.* ...
  theta)).*(q04.*sin((1/2).*(1+(-1).*t).*theta)+q14.*sin((1/2).*t.*theta)) ...
  ).^2+4.*((-1).*csc((1/2).*theta).^2.*(q01.*sin((1/2).*(1+(-1).*t).* ...
  theta)+q11.*sin((1/2).*t.*theta)).*(q02.*sin((1/2).*(1+(-1).*t).*theta)+ ...
  q12.*sin((1/2).*t.*theta))+csc((1/2).*theta).^2.*(q03.*sin((1/2).*(1+( ...
  -1).*t).*theta)+q13.*sin((1/2).*t.*theta)).*(q04.*sin((1/2).*(1+(-1).*t) ...
  .*theta)+q14.*sin((1/2).*t.*theta))).^2+(1+(-2).*(csc((1/2).*theta).^2.* ...
  (q02.*sin((1/2).*(1+(-1).*t).*theta)+q12.*sin((1/2).*t.*theta)).^2+csc(( ...
  1/2).*theta).^2.*(q03.*sin((1/2).*(1+(-1).*t).*theta)+q13.*sin((1/2).* ...
  t.*theta)).^2)).^2)+(-1).*(1+(-2).*(csc((1/2).*theta).^2.*(q03.*sin(( ...
  1/2).*(1+(-1).*t).*theta)+q13.*sin((1/2).*t.*theta)).^2+csc((1/2).* ...
  theta).^2.*(q04.*sin((1/2).*(1+(-1).*t).*theta)+q14.*sin((1/2).*t.* ...
  theta)).^2)).^2.*(8.*((-1).*((-1/2).*q02.*theta.*cos((1/2).*(1+(-1).*t) ...
  .*theta)+(1/2).*q12.*theta.*cos((1/2).*t.*theta)).*csc((1/2).*theta) ...
  .^2.*(q01.*sin((1/2).*(1+(-1).*t).*theta)+q11.*sin((1/2).*t.*theta))+( ...
  -1).*((-1/2).*q01.*theta.*cos((1/2).*(1+(-1).*t).*theta)+(1/2).*q11.* ...
  theta.*cos((1/2).*t.*theta)).*csc((1/2).*theta).^2.*(q02.*sin((1/2).*(1+ ...
  (-1).*t).*theta)+q12.*sin((1/2).*t.*theta))+((-1/2).*q04.*theta.*cos(( ...
  1/2).*(1+(-1).*t).*theta)+(1/2).*q14.*theta.*cos((1/2).*t.*theta)).*csc( ...
  (1/2).*theta).^2.*(q03.*sin((1/2).*(1+(-1).*t).*theta)+q13.*sin((1/2).* ...
  t.*theta))+((-1/2).*q03.*theta.*cos((1/2).*(1+(-1).*t).*theta)+(1/2).* ...
  q13.*theta.*cos((1/2).*t.*theta)).*csc((1/2).*theta).^2.*(q04.*sin((1/2) ...
  .*(1+(-1).*t).*theta)+q14.*sin((1/2).*t.*theta))).*((-1).*csc((1/2).* ...
  theta).^2.*(q01.*sin((1/2).*(1+(-1).*t).*theta)+q11.*sin((1/2).*t.* ...
  theta)).*(q02.*sin((1/2).*(1+(-1).*t).*theta)+q12.*sin((1/2).*t.*theta)) ...
  +csc((1/2).*theta).^2.*(q03.*sin((1/2).*(1+(-1).*t).*theta)+q13.*sin(( ...
  1/2).*t.*theta)).*(q04.*sin((1/2).*(1+(-1).*t).*theta)+q14.*sin((1/2).* ...
  t.*theta)))+(-4).*(2.*((-1/2).*q02.*theta.*cos((1/2).*(1+(-1).*t).* ...
  theta)+(1/2).*q12.*theta.*cos((1/2).*t.*theta)).*csc((1/2).*theta).^2.*( ...
  q02.*sin((1/2).*(1+(-1).*t).*theta)+q12.*sin((1/2).*t.*theta))+2.*(( ...
  -1/2).*q03.*theta.*cos((1/2).*(1+(-1).*t).*theta)+(1/2).*q13.*theta.* ...
  cos((1/2).*t.*theta)).*csc((1/2).*theta).^2.*(q03.*sin((1/2).*(1+(-1).* ...
  t).*theta)+q13.*sin((1/2).*t.*theta))).*(1+(-2).*(csc((1/2).*theta).^2.* ...
  (q02.*sin((1/2).*(1+(-1).*t).*theta)+q12.*sin((1/2).*t.*theta)).^2+csc(( ...
  1/2).*theta).^2.*(q03.*sin((1/2).*(1+(-1).*t).*theta)+q13.*sin((1/2).* ...
  t.*theta)).^2))).*(4.*((-1).*csc((1/2).*theta).^2.*(q01.*sin((1/2).*(1+( ...
  -1).*t).*theta)+q11.*sin((1/2).*t.*theta)).*(q02.*sin((1/2).*(1+(-1).*t) ...
  .*theta)+q12.*sin((1/2).*t.*theta))+csc((1/2).*theta).^2.*(q03.*sin(( ...
  1/2).*(1+(-1).*t).*theta)+q13.*sin((1/2).*t.*theta)).*(q04.*sin((1/2).*( ...
  1+(-1).*t).*theta)+q14.*sin((1/2).*t.*theta))).^2+(1+(-2).*(csc((1/2).* ...
  theta).^2.*(q02.*sin((1/2).*(1+(-1).*t).*theta)+q12.*sin((1/2).*t.* ...
  theta)).^2+csc((1/2).*theta).^2.*(q03.*sin((1/2).*(1+(-1).*t).*theta)+ ...
  q13.*sin((1/2).*t.*theta)).^2)).^2).^(-2).*(4.*(csc((1/2).*theta).^2.*( ...
  q01.*sin((1/2).*(1+(-1).*t).*theta)+q11.*sin((1/2).*t.*theta)).*(q03.* ...
  sin((1/2).*(1+(-1).*t).*theta)+q13.*sin((1/2).*t.*theta))+csc((1/2).* ...
  theta).^2.*(q02.*sin((1/2).*(1+(-1).*t).*theta)+q12.*sin((1/2).*t.* ...
  theta)).*(q04.*sin((1/2).*(1+(-1).*t).*theta)+q14.*sin((1/2).*t.*theta)) ...
  ).^2+4.*((-1).*csc((1/2).*theta).^2.*(q01.*sin((1/2).*(1+(-1).*t).* ...
  theta)+q11.*sin((1/2).*t.*theta)).*(q02.*sin((1/2).*(1+(-1).*t).*theta)+ ...
  q12.*sin((1/2).*t.*theta))+csc((1/2).*theta).^2.*(q03.*sin((1/2).*(1+( ...
  -1).*t).*theta)+q13.*sin((1/2).*t.*theta)).*(q04.*sin((1/2).*(1+(-1).*t) ...
  .*theta)+q14.*sin((1/2).*t.*theta))).^2+(1+(-2).*(csc((1/2).*theta).^2.* ...
  (q02.*sin((1/2).*(1+(-1).*t).*theta)+q12.*sin((1/2).*t.*theta)).^2+csc(( ...
  1/2).*theta).^2.*(q03.*sin((1/2).*(1+(-1).*t).*theta)+q13.*sin((1/2).* ...
  t.*theta)).^2)).^2)+8.*((-1).*((-1/2).*q04.*theta.*cos((1/2).*(1+(-1).* ...
  t).*theta)+(1/2).*q14.*theta.*cos((1/2).*t.*theta)).*csc((1/2).*theta) ...
  .^2.*(q01.*sin((1/2).*(1+(-1).*t).*theta)+q11.*sin((1/2).*t.*theta))+(( ...
  -1/2).*q03.*theta.*cos((1/2).*(1+(-1).*t).*theta)+(1/2).*q13.*theta.* ...
  cos((1/2).*t.*theta)).*csc((1/2).*theta).^2.*(q02.*sin((1/2).*(1+(-1).* ...
  t).*theta)+q12.*sin((1/2).*t.*theta))+((-1/2).*q02.*theta.*cos((1/2).*( ...
  1+(-1).*t).*theta)+(1/2).*q12.*theta.*cos((1/2).*t.*theta)).*csc((1/2).* ...
  theta).^2.*(q03.*sin((1/2).*(1+(-1).*t).*theta)+q13.*sin((1/2).*t.* ...
  theta))+(-1).*((-1/2).*q01.*theta.*cos((1/2).*(1+(-1).*t).*theta)+(1/2) ...
  .*q11.*theta.*cos((1/2).*t.*theta)).*csc((1/2).*theta).^2.*(q04.*sin(( ...
  1/2).*(1+(-1).*t).*theta)+q14.*sin((1/2).*t.*theta))).*(csc((1/2).* ...
  theta).^2.*(q02.*sin((1/2).*(1+(-1).*t).*theta)+q12.*sin((1/2).*t.* ...
  theta)).*(q03.*sin((1/2).*(1+(-1).*t).*theta)+q13.*sin((1/2).*t.*theta)) ...
  +(-1).*csc((1/2).*theta).^2.*(q01.*sin((1/2).*(1+(-1).*t).*theta)+q11.* ...
  sin((1/2).*t.*theta)).*(q04.*sin((1/2).*(1+(-1).*t).*theta)+q14.*sin(( ...
  1/2).*t.*theta))).*(4.*((-1).*csc((1/2).*theta).^2.*(q01.*sin((1/2).*(1+ ...
  (-1).*t).*theta)+q11.*sin((1/2).*t.*theta)).*(q02.*sin((1/2).*(1+(-1).* ...
  t).*theta)+q12.*sin((1/2).*t.*theta))+csc((1/2).*theta).^2.*(q03.*sin(( ...
  1/2).*(1+(-1).*t).*theta)+q13.*sin((1/2).*t.*theta)).*(q04.*sin((1/2).*( ...
  1+(-1).*t).*theta)+q14.*sin((1/2).*t.*theta))).^2+(1+(-2).*(csc((1/2).* ...
  theta).^2.*(q02.*sin((1/2).*(1+(-1).*t).*theta)+q12.*sin((1/2).*t.* ...
  theta)).^2+csc((1/2).*theta).^2.*(q03.*sin((1/2).*(1+(-1).*t).*theta)+ ...
  q13.*sin((1/2).*t.*theta)).^2)).^2).^(-1).*(4.*(csc((1/2).*theta).^2.*( ...
  q01.*sin((1/2).*(1+(-1).*t).*theta)+q11.*sin((1/2).*t.*theta)).*(q03.* ...
  sin((1/2).*(1+(-1).*t).*theta)+q13.*sin((1/2).*t.*theta))+csc((1/2).* ...
  theta).^2.*(q02.*sin((1/2).*(1+(-1).*t).*theta)+q12.*sin((1/2).*t.* ...
  theta)).*(q04.*sin((1/2).*(1+(-1).*t).*theta)+q14.*sin((1/2).*t.*theta)) ...
  ).^2+4.*((-1).*csc((1/2).*theta).^2.*(q01.*sin((1/2).*(1+(-1).*t).* ...
  theta)+q11.*sin((1/2).*t.*theta)).*(q02.*sin((1/2).*(1+(-1).*t).*theta)+ ...
  q12.*sin((1/2).*t.*theta))+csc((1/2).*theta).^2.*(q03.*sin((1/2).*(1+( ...
  -1).*t).*theta)+q13.*sin((1/2).*t.*theta)).*(q04.*sin((1/2).*(1+(-1).*t) ...
  .*theta)+q14.*sin((1/2).*t.*theta))).^2+(1+(-2).*(csc((1/2).*theta).^2.* ...
  (q02.*sin((1/2).*(1+(-1).*t).*theta)+q12.*sin((1/2).*t.*theta)).^2+csc(( ...
  1/2).*theta).^2.*(q03.*sin((1/2).*(1+(-1).*t).*theta)+q13.*sin((1/2).* ...
  t.*theta)).^2)).^2)+(-4).*(2.*((-1/2).*q03.*theta.*cos((1/2).*(1+(-1).* ...
  t).*theta)+(1/2).*q13.*theta.*cos((1/2).*t.*theta)).*csc((1/2).*theta) ...
  .^2.*(q03.*sin((1/2).*(1+(-1).*t).*theta)+q13.*sin((1/2).*t.*theta))+2.* ...
  ((-1/2).*q04.*theta.*cos((1/2).*(1+(-1).*t).*theta)+(1/2).*q14.*theta.* ...
  cos((1/2).*t.*theta)).*csc((1/2).*theta).^2.*(q04.*sin((1/2).*(1+(-1).* ...
  t).*theta)+q14.*sin((1/2).*t.*theta))).*(1+(-2).*(csc((1/2).*theta).^2.* ...
  (q03.*sin((1/2).*(1+(-1).*t).*theta)+q13.*sin((1/2).*t.*theta)).^2+csc(( ...
  1/2).*theta).^2.*(q04.*sin((1/2).*(1+(-1).*t).*theta)+q14.*sin((1/2).* ...
  t.*theta)).^2)).*(4.*((-1).*csc((1/2).*theta).^2.*(q01.*sin((1/2).*(1+( ...
  -1).*t).*theta)+q11.*sin((1/2).*t.*theta)).*(q02.*sin((1/2).*(1+(-1).*t) ...
  .*theta)+q12.*sin((1/2).*t.*theta))+csc((1/2).*theta).^2.*(q03.*sin(( ...
  1/2).*(1+(-1).*t).*theta)+q13.*sin((1/2).*t.*theta)).*(q04.*sin((1/2).*( ...
  1+(-1).*t).*theta)+q14.*sin((1/2).*t.*theta))).^2+(1+(-2).*(csc((1/2).* ...
  theta).^2.*(q02.*sin((1/2).*(1+(-1).*t).*theta)+q12.*sin((1/2).*t.* ...
  theta)).^2+csc((1/2).*theta).^2.*(q03.*sin((1/2).*(1+(-1).*t).*theta)+ ...
  q13.*sin((1/2).*t.*theta)).^2)).^2).^(-1).*(4.*(csc((1/2).*theta).^2.*( ...
  q01.*sin((1/2).*(1+(-1).*t).*theta)+q11.*sin((1/2).*t.*theta)).*(q03.* ...
  sin((1/2).*(1+(-1).*t).*theta)+q13.*sin((1/2).*t.*theta))+csc((1/2).* ...
  theta).^2.*(q02.*sin((1/2).*(1+(-1).*t).*theta)+q12.*sin((1/2).*t.* ...
  theta)).*(q04.*sin((1/2).*(1+(-1).*t).*theta)+q14.*sin((1/2).*t.*theta)) ...
  ).^2+4.*((-1).*csc((1/2).*theta).^2.*(q01.*sin((1/2).*(1+(-1).*t).* ...
  theta)+q11.*sin((1/2).*t.*theta)).*(q02.*sin((1/2).*(1+(-1).*t).*theta)+ ...
  q12.*sin((1/2).*t.*theta))+csc((1/2).*theta).^2.*(q03.*sin((1/2).*(1+( ...
  -1).*t).*theta)+q13.*sin((1/2).*t.*theta)).*(q04.*sin((1/2).*(1+(-1).*t) ...
  .*theta)+q14.*sin((1/2).*t.*theta))).^2+(1+(-2).*(csc((1/2).*theta).^2.* ...
  (q02.*sin((1/2).*(1+(-1).*t).*theta)+q12.*sin((1/2).*t.*theta)).^2+csc(( ...
  1/2).*theta).^2.*(q03.*sin((1/2).*(1+(-1).*t).*theta)+q13.*sin((1/2).* ...
  t.*theta)).^2)).^2)).*(4.*(csc((1/2).*theta).^2.*(q02.*sin((1/2).*(1+( ...
  -1).*t).*theta)+q12.*sin((1/2).*t.*theta)).*(q03.*sin((1/2).*(1+(-1).*t) ...
  .*theta)+q13.*sin((1/2).*t.*theta))+(-1).*csc((1/2).*theta).^2.*(q01.* ...
  sin((1/2).*(1+(-1).*t).*theta)+q11.*sin((1/2).*t.*theta)).*(q04.*sin(( ...
  1/2).*(1+(-1).*t).*theta)+q14.*sin((1/2).*t.*theta))).^2.*(4.*((-1).* ...
  csc((1/2).*theta).^2.*(q01.*sin((1/2).*(1+(-1).*t).*theta)+q11.*sin(( ...
  1/2).*t.*theta)).*(q02.*sin((1/2).*(1+(-1).*t).*theta)+q12.*sin((1/2).* ...
  t.*theta))+csc((1/2).*theta).^2.*(q03.*sin((1/2).*(1+(-1).*t).*theta)+ ...
  q13.*sin((1/2).*t.*theta)).*(q04.*sin((1/2).*(1+(-1).*t).*theta)+q14.* ...
  sin((1/2).*t.*theta))).^2+(1+(-2).*(csc((1/2).*theta).^2.*(q02.*sin(( ...
  1/2).*(1+(-1).*t).*theta)+q12.*sin((1/2).*t.*theta)).^2+csc((1/2).* ...
  theta).^2.*(q03.*sin((1/2).*(1+(-1).*t).*theta)+q13.*sin((1/2).*t.* ...
  theta)).^2)).^2).^(-1).*(4.*(csc((1/2).*theta).^2.*(q01.*sin((1/2).*(1+( ...
  -1).*t).*theta)+q11.*sin((1/2).*t.*theta)).*(q03.*sin((1/2).*(1+(-1).*t) ...
  .*theta)+q13.*sin((1/2).*t.*theta))+csc((1/2).*theta).^2.*(q02.*sin(( ...
  1/2).*(1+(-1).*t).*theta)+q12.*sin((1/2).*t.*theta)).*(q04.*sin((1/2).*( ...
  1+(-1).*t).*theta)+q14.*sin((1/2).*t.*theta))).^2+4.*((-1).*csc((1/2).* ...
  theta).^2.*(q01.*sin((1/2).*(1+(-1).*t).*theta)+q11.*sin((1/2).*t.* ...
  theta)).*(q02.*sin((1/2).*(1+(-1).*t).*theta)+q12.*sin((1/2).*t.*theta)) ...
  +csc((1/2).*theta).^2.*(q03.*sin((1/2).*(1+(-1).*t).*theta)+q13.*sin(( ...
  1/2).*t.*theta)).*(q04.*sin((1/2).*(1+(-1).*t).*theta)+q14.*sin((1/2).* ...
  t.*theta))).^2+(1+(-2).*(csc((1/2).*theta).^2.*(q02.*sin((1/2).*(1+(-1) ...
  .*t).*theta)+q12.*sin((1/2).*t.*theta)).^2+csc((1/2).*theta).^2.*(q03.* ...
  sin((1/2).*(1+(-1).*t).*theta)+q13.*sin((1/2).*t.*theta)).^2)).^2)+(1+( ...
  -2).*(csc((1/2).*theta).^2.*(q03.*sin((1/2).*(1+(-1).*t).*theta)+q13.* ...
  sin((1/2).*t.*theta)).^2+csc((1/2).*theta).^2.*(q04.*sin((1/2).*(1+(-1) ...
  .*t).*theta)+q14.*sin((1/2).*t.*theta)).^2)).^2.*(4.*((-1).*csc((1/2).* ...
  theta).^2.*(q01.*sin((1/2).*(1+(-1).*t).*theta)+q11.*sin((1/2).*t.* ...
  theta)).*(q02.*sin((1/2).*(1+(-1).*t).*theta)+q12.*sin((1/2).*t.*theta)) ...
  +csc((1/2).*theta).^2.*(q03.*sin((1/2).*(1+(-1).*t).*theta)+q13.*sin(( ...
  1/2).*t.*theta)).*(q04.*sin((1/2).*(1+(-1).*t).*theta)+q14.*sin((1/2).* ...
  t.*theta))).^2+(1+(-2).*(csc((1/2).*theta).^2.*(q02.*sin((1/2).*(1+(-1) ...
  .*t).*theta)+q12.*sin((1/2).*t.*theta)).^2+csc((1/2).*theta).^2.*(q03.* ...
  sin((1/2).*(1+(-1).*t).*theta)+q13.*sin((1/2).*t.*theta)).^2)).^2).^(-1) ...
  .*(4.*(csc((1/2).*theta).^2.*(q01.*sin((1/2).*(1+(-1).*t).*theta)+q11.* ...
  sin((1/2).*t.*theta)).*(q03.*sin((1/2).*(1+(-1).*t).*theta)+q13.*sin(( ...
  1/2).*t.*theta))+csc((1/2).*theta).^2.*(q02.*sin((1/2).*(1+(-1).*t).* ...
  theta)+q12.*sin((1/2).*t.*theta)).*(q04.*sin((1/2).*(1+(-1).*t).*theta)+ ...
  q14.*sin((1/2).*t.*theta))).^2+4.*((-1).*csc((1/2).*theta).^2.*(q01.* ...
  sin((1/2).*(1+(-1).*t).*theta)+q11.*sin((1/2).*t.*theta)).*(q02.*sin(( ...
  1/2).*(1+(-1).*t).*theta)+q12.*sin((1/2).*t.*theta))+csc((1/2).*theta) ...
  .^2.*(q03.*sin((1/2).*(1+(-1).*t).*theta)+q13.*sin((1/2).*t.*theta)).*( ...
  q04.*sin((1/2).*(1+(-1).*t).*theta)+q14.*sin((1/2).*t.*theta))).^2+(1+( ...
  -2).*(csc((1/2).*theta).^2.*(q02.*sin((1/2).*(1+(-1).*t).*theta)+q12.* ...
  sin((1/2).*t.*theta)).^2+csc((1/2).*theta).^2.*(q03.*sin((1/2).*(1+(-1) ...
  .*t).*theta)+q13.*sin((1/2).*t.*theta)).^2)).^2)).^(-2)+(-2).*(csc((1/2) ...
  .*theta).^2.*(q02.*sin((1/2).*(1+(-1).*t).*theta)+q12.*sin((1/2).*t.* ...
  theta)).*(q03.*sin((1/2).*(1+(-1).*t).*theta)+q13.*sin((1/2).*t.*theta)) ...
  +(-1).*csc((1/2).*theta).^2.*(q01.*sin((1/2).*(1+(-1).*t).*theta)+q11.* ...
  sin((1/2).*t.*theta)).*(q04.*sin((1/2).*(1+(-1).*t).*theta)+q14.*sin(( ...
  1/2).*t.*theta))).*(4.*((-1).*csc((1/2).*theta).^2.*(q01.*sin((1/2).*(1+ ...
  (-1).*t).*theta)+q11.*sin((1/2).*t.*theta)).*(q02.*sin((1/2).*(1+(-1).* ...
  t).*theta)+q12.*sin((1/2).*t.*theta))+csc((1/2).*theta).^2.*(q03.*sin(( ...
  1/2).*(1+(-1).*t).*theta)+q13.*sin((1/2).*t.*theta)).*(q04.*sin((1/2).*( ...
  1+(-1).*t).*theta)+q14.*sin((1/2).*t.*theta))).^2+(1+(-2).*(csc((1/2).* ...
  theta).^2.*(q02.*sin((1/2).*(1+(-1).*t).*theta)+q12.*sin((1/2).*t.* ...
  theta)).^2+csc((1/2).*theta).^2.*(q03.*sin((1/2).*(1+(-1).*t).*theta)+ ...
  q13.*sin((1/2).*t.*theta)).^2)).^2).^(-1/2).*(4.*(csc((1/2).*theta).^2.* ...
  (q01.*sin((1/2).*(1+(-1).*t).*theta)+q11.*sin((1/2).*t.*theta)).*(q03.* ...
  sin((1/2).*(1+(-1).*t).*theta)+q13.*sin((1/2).*t.*theta))+csc((1/2).* ...
  theta).^2.*(q02.*sin((1/2).*(1+(-1).*t).*theta)+q12.*sin((1/2).*t.* ...
  theta)).*(q04.*sin((1/2).*(1+(-1).*t).*theta)+q14.*sin((1/2).*t.*theta)) ...
  ).^2+4.*((-1).*csc((1/2).*theta).^2.*(q01.*sin((1/2).*(1+(-1).*t).* ...
  theta)+q11.*sin((1/2).*t.*theta)).*(q02.*sin((1/2).*(1+(-1).*t).*theta)+ ...
  q12.*sin((1/2).*t.*theta))+csc((1/2).*theta).^2.*(q03.*sin((1/2).*(1+( ...
  -1).*t).*theta)+q13.*sin((1/2).*t.*theta)).*(q04.*sin((1/2).*(1+(-1).*t) ...
  .*theta)+q14.*sin((1/2).*t.*theta))).^2+(1+(-2).*(csc((1/2).*theta).^2.* ...
  (q02.*sin((1/2).*(1+(-1).*t).*theta)+q12.*sin((1/2).*t.*theta)).^2+csc(( ...
  1/2).*theta).^2.*(q03.*sin((1/2).*(1+(-1).*t).*theta)+q13.*sin((1/2).* ...
  t.*theta)).^2)).^2).^(1/2).*((1/2).*(1+(-2).*(csc((1/2).*theta).^2.*( ...
  q03.*sin((1/2).*(1+(-1).*t).*theta)+q13.*sin((1/2).*t.*theta)).^2+csc(( ...
  1/2).*theta).^2.*(q04.*sin((1/2).*(1+(-1).*t).*theta)+q14.*sin((1/2).* ...
  t.*theta)).^2)).*(8.*(((-1/2).*q03.*theta.*cos((1/2).*(1+(-1).*t).* ...
  theta)+(1/2).*q13.*theta.*cos((1/2).*t.*theta)).*csc((1/2).*theta).^2.*( ...
  q01.*sin((1/2).*(1+(-1).*t).*theta)+q11.*sin((1/2).*t.*theta))+((-1/2).* ...
  q04.*theta.*cos((1/2).*(1+(-1).*t).*theta)+(1/2).*q14.*theta.*cos((1/2) ...
  .*t.*theta)).*csc((1/2).*theta).^2.*(q02.*sin((1/2).*(1+(-1).*t).*theta) ...
  +q12.*sin((1/2).*t.*theta))+((-1/2).*q01.*theta.*cos((1/2).*(1+(-1).*t) ...
  .*theta)+(1/2).*q11.*theta.*cos((1/2).*t.*theta)).*csc((1/2).*theta) ...
  .^2.*(q03.*sin((1/2).*(1+(-1).*t).*theta)+q13.*sin((1/2).*t.*theta))+(( ...
  -1/2).*q02.*theta.*cos((1/2).*(1+(-1).*t).*theta)+(1/2).*q12.*theta.* ...
  cos((1/2).*t.*theta)).*csc((1/2).*theta).^2.*(q04.*sin((1/2).*(1+(-1).* ...
  t).*theta)+q14.*sin((1/2).*t.*theta))).*(csc((1/2).*theta).^2.*(q01.* ...
  sin((1/2).*(1+(-1).*t).*theta)+q11.*sin((1/2).*t.*theta)).*(q03.*sin(( ...
  1/2).*(1+(-1).*t).*theta)+q13.*sin((1/2).*t.*theta))+csc((1/2).*theta) ...
  .^2.*(q02.*sin((1/2).*(1+(-1).*t).*theta)+q12.*sin((1/2).*t.*theta)).*( ...
  q04.*sin((1/2).*(1+(-1).*t).*theta)+q14.*sin((1/2).*t.*theta)))+8.*((-1) ...
  .*((-1/2).*q02.*theta.*cos((1/2).*(1+(-1).*t).*theta)+(1/2).*q12.* ...
  theta.*cos((1/2).*t.*theta)).*csc((1/2).*theta).^2.*(q01.*sin((1/2).*(1+ ...
  (-1).*t).*theta)+q11.*sin((1/2).*t.*theta))+(-1).*((-1/2).*q01.*theta.* ...
  cos((1/2).*(1+(-1).*t).*theta)+(1/2).*q11.*theta.*cos((1/2).*t.*theta)) ...
  .*csc((1/2).*theta).^2.*(q02.*sin((1/2).*(1+(-1).*t).*theta)+q12.*sin(( ...
  1/2).*t.*theta))+((-1/2).*q04.*theta.*cos((1/2).*(1+(-1).*t).*theta)+( ...
  1/2).*q14.*theta.*cos((1/2).*t.*theta)).*csc((1/2).*theta).^2.*(q03.* ...
  sin((1/2).*(1+(-1).*t).*theta)+q13.*sin((1/2).*t.*theta))+((-1/2).*q03.* ...
  theta.*cos((1/2).*(1+(-1).*t).*theta)+(1/2).*q13.*theta.*cos((1/2).*t.* ...
  theta)).*csc((1/2).*theta).^2.*(q04.*sin((1/2).*(1+(-1).*t).*theta)+ ...
  q14.*sin((1/2).*t.*theta))).*((-1).*csc((1/2).*theta).^2.*(q01.*sin(( ...
  1/2).*(1+(-1).*t).*theta)+q11.*sin((1/2).*t.*theta)).*(q02.*sin((1/2).*( ...
  1+(-1).*t).*theta)+q12.*sin((1/2).*t.*theta))+csc((1/2).*theta).^2.*( ...
  q03.*sin((1/2).*(1+(-1).*t).*theta)+q13.*sin((1/2).*t.*theta)).*(q04.* ...
  sin((1/2).*(1+(-1).*t).*theta)+q14.*sin((1/2).*t.*theta)))+(-4).*(2.*(( ...
  -1/2).*q02.*theta.*cos((1/2).*(1+(-1).*t).*theta)+(1/2).*q12.*theta.* ...
  cos((1/2).*t.*theta)).*csc((1/2).*theta).^2.*(q02.*sin((1/2).*(1+(-1).* ...
  t).*theta)+q12.*sin((1/2).*t.*theta))+2.*((-1/2).*q03.*theta.*cos((1/2) ...
  .*(1+(-1).*t).*theta)+(1/2).*q13.*theta.*cos((1/2).*t.*theta)).*csc(( ...
  1/2).*theta).^2.*(q03.*sin((1/2).*(1+(-1).*t).*theta)+q13.*sin((1/2).* ...
  t.*theta))).*(1+(-2).*(csc((1/2).*theta).^2.*(q02.*sin((1/2).*(1+(-1).* ...
  t).*theta)+q12.*sin((1/2).*t.*theta)).^2+csc((1/2).*theta).^2.*(q03.* ...
  sin((1/2).*(1+(-1).*t).*theta)+q13.*sin((1/2).*t.*theta)).^2))).*(4.*(( ...
  -1).*csc((1/2).*theta).^2.*(q01.*sin((1/2).*(1+(-1).*t).*theta)+q11.* ...
  sin((1/2).*t.*theta)).*(q02.*sin((1/2).*(1+(-1).*t).*theta)+q12.*sin(( ...
  1/2).*t.*theta))+csc((1/2).*theta).^2.*(q03.*sin((1/2).*(1+(-1).*t).* ...
  theta)+q13.*sin((1/2).*t.*theta)).*(q04.*sin((1/2).*(1+(-1).*t).*theta)+ ...
  q14.*sin((1/2).*t.*theta))).^2+(1+(-2).*(csc((1/2).*theta).^2.*(q02.* ...
  sin((1/2).*(1+(-1).*t).*theta)+q12.*sin((1/2).*t.*theta)).^2+csc((1/2).* ...
  theta).^2.*(q03.*sin((1/2).*(1+(-1).*t).*theta)+q13.*sin((1/2).*t.* ...
  theta)).^2)).^2).^(-1/2).*(4.*(csc((1/2).*theta).^2.*(q01.*sin((1/2).*( ...
  1+(-1).*t).*theta)+q11.*sin((1/2).*t.*theta)).*(q03.*sin((1/2).*(1+(-1) ...
  .*t).*theta)+q13.*sin((1/2).*t.*theta))+csc((1/2).*theta).^2.*(q02.*sin( ...
  (1/2).*(1+(-1).*t).*theta)+q12.*sin((1/2).*t.*theta)).*(q04.*sin((1/2).* ...
  (1+(-1).*t).*theta)+q14.*sin((1/2).*t.*theta))).^2+4.*((-1).*csc((1/2).* ...
  theta).^2.*(q01.*sin((1/2).*(1+(-1).*t).*theta)+q11.*sin((1/2).*t.* ...
  theta)).*(q02.*sin((1/2).*(1+(-1).*t).*theta)+q12.*sin((1/2).*t.*theta)) ...
  +csc((1/2).*theta).^2.*(q03.*sin((1/2).*(1+(-1).*t).*theta)+q13.*sin(( ...
  1/2).*t.*theta)).*(q04.*sin((1/2).*(1+(-1).*t).*theta)+q14.*sin((1/2).* ...
  t.*theta))).^2+(1+(-2).*(csc((1/2).*theta).^2.*(q02.*sin((1/2).*(1+(-1) ...
  .*t).*theta)+q12.*sin((1/2).*t.*theta)).^2+csc((1/2).*theta).^2.*(q03.* ...
  sin((1/2).*(1+(-1).*t).*theta)+q13.*sin((1/2).*t.*theta)).^2)).^2).^( ...
  -1/2)+(-1/2).*(1+(-2).*(csc((1/2).*theta).^2.*(q03.*sin((1/2).*(1+(-1).* ...
  t).*theta)+q13.*sin((1/2).*t.*theta)).^2+csc((1/2).*theta).^2.*(q04.* ...
  sin((1/2).*(1+(-1).*t).*theta)+q14.*sin((1/2).*t.*theta)).^2)).*(8.*(( ...
  -1).*((-1/2).*q02.*theta.*cos((1/2).*(1+(-1).*t).*theta)+(1/2).*q12.* ...
  theta.*cos((1/2).*t.*theta)).*csc((1/2).*theta).^2.*(q01.*sin((1/2).*(1+ ...
  (-1).*t).*theta)+q11.*sin((1/2).*t.*theta))+(-1).*((-1/2).*q01.*theta.* ...
  cos((1/2).*(1+(-1).*t).*theta)+(1/2).*q11.*theta.*cos((1/2).*t.*theta)) ...
  .*csc((1/2).*theta).^2.*(q02.*sin((1/2).*(1+(-1).*t).*theta)+q12.*sin(( ...
  1/2).*t.*theta))+((-1/2).*q04.*theta.*cos((1/2).*(1+(-1).*t).*theta)+( ...
  1/2).*q14.*theta.*cos((1/2).*t.*theta)).*csc((1/2).*theta).^2.*(q03.* ...
  sin((1/2).*(1+(-1).*t).*theta)+q13.*sin((1/2).*t.*theta))+((-1/2).*q03.* ...
  theta.*cos((1/2).*(1+(-1).*t).*theta)+(1/2).*q13.*theta.*cos((1/2).*t.* ...
  theta)).*csc((1/2).*theta).^2.*(q04.*sin((1/2).*(1+(-1).*t).*theta)+ ...
  q14.*sin((1/2).*t.*theta))).*((-1).*csc((1/2).*theta).^2.*(q01.*sin(( ...
  1/2).*(1+(-1).*t).*theta)+q11.*sin((1/2).*t.*theta)).*(q02.*sin((1/2).*( ...
  1+(-1).*t).*theta)+q12.*sin((1/2).*t.*theta))+csc((1/2).*theta).^2.*( ...
  q03.*sin((1/2).*(1+(-1).*t).*theta)+q13.*sin((1/2).*t.*theta)).*(q04.* ...
  sin((1/2).*(1+(-1).*t).*theta)+q14.*sin((1/2).*t.*theta)))+(-4).*(2.*(( ...
  -1/2).*q02.*theta.*cos((1/2).*(1+(-1).*t).*theta)+(1/2).*q12.*theta.* ...
  cos((1/2).*t.*theta)).*csc((1/2).*theta).^2.*(q02.*sin((1/2).*(1+(-1).* ...
  t).*theta)+q12.*sin((1/2).*t.*theta))+2.*((-1/2).*q03.*theta.*cos((1/2) ...
  .*(1+(-1).*t).*theta)+(1/2).*q13.*theta.*cos((1/2).*t.*theta)).*csc(( ...
  1/2).*theta).^2.*(q03.*sin((1/2).*(1+(-1).*t).*theta)+q13.*sin((1/2).* ...
  t.*theta))).*(1+(-2).*(csc((1/2).*theta).^2.*(q02.*sin((1/2).*(1+(-1).* ...
  t).*theta)+q12.*sin((1/2).*t.*theta)).^2+csc((1/2).*theta).^2.*(q03.* ...
  sin((1/2).*(1+(-1).*t).*theta)+q13.*sin((1/2).*t.*theta)).^2))).*(4.*(( ...
  -1).*csc((1/2).*theta).^2.*(q01.*sin((1/2).*(1+(-1).*t).*theta)+q11.* ...
  sin((1/2).*t.*theta)).*(q02.*sin((1/2).*(1+(-1).*t).*theta)+q12.*sin(( ...
  1/2).*t.*theta))+csc((1/2).*theta).^2.*(q03.*sin((1/2).*(1+(-1).*t).* ...
  theta)+q13.*sin((1/2).*t.*theta)).*(q04.*sin((1/2).*(1+(-1).*t).*theta)+ ...
  q14.*sin((1/2).*t.*theta))).^2+(1+(-2).*(csc((1/2).*theta).^2.*(q02.* ...
  sin((1/2).*(1+(-1).*t).*theta)+q12.*sin((1/2).*t.*theta)).^2+csc((1/2).* ...
  theta).^2.*(q03.*sin((1/2).*(1+(-1).*t).*theta)+q13.*sin((1/2).*t.* ...
  theta)).^2)).^2).^(-3/2).*(4.*(csc((1/2).*theta).^2.*(q01.*sin((1/2).*( ...
  1+(-1).*t).*theta)+q11.*sin((1/2).*t.*theta)).*(q03.*sin((1/2).*(1+(-1) ...
  .*t).*theta)+q13.*sin((1/2).*t.*theta))+csc((1/2).*theta).^2.*(q02.*sin( ...
  (1/2).*(1+(-1).*t).*theta)+q12.*sin((1/2).*t.*theta)).*(q04.*sin((1/2).* ...
  (1+(-1).*t).*theta)+q14.*sin((1/2).*t.*theta))).^2+4.*((-1).*csc((1/2).* ...
  theta).^2.*(q01.*sin((1/2).*(1+(-1).*t).*theta)+q11.*sin((1/2).*t.* ...
  theta)).*(q02.*sin((1/2).*(1+(-1).*t).*theta)+q12.*sin((1/2).*t.*theta)) ...
  +csc((1/2).*theta).^2.*(q03.*sin((1/2).*(1+(-1).*t).*theta)+q13.*sin(( ...
  1/2).*t.*theta)).*(q04.*sin((1/2).*(1+(-1).*t).*theta)+q14.*sin((1/2).* ...
  t.*theta))).^2+(1+(-2).*(csc((1/2).*theta).^2.*(q02.*sin((1/2).*(1+(-1) ...
  .*t).*theta)+q12.*sin((1/2).*t.*theta)).^2+csc((1/2).*theta).^2.*(q03.* ...
  sin((1/2).*(1+(-1).*t).*theta)+q13.*sin((1/2).*t.*theta)).^2)).^2).^( ...
  1/2)+(-2).*(2.*((-1/2).*q03.*theta.*cos((1/2).*(1+(-1).*t).*theta)+(1/2) ...
  .*q13.*theta.*cos((1/2).*t.*theta)).*csc((1/2).*theta).^2.*(q03.*sin(( ...
  1/2).*(1+(-1).*t).*theta)+q13.*sin((1/2).*t.*theta))+2.*((-1/2).*q04.* ...
  theta.*cos((1/2).*(1+(-1).*t).*theta)+(1/2).*q14.*theta.*cos((1/2).*t.* ...
  theta)).*csc((1/2).*theta).^2.*(q04.*sin((1/2).*(1+(-1).*t).*theta)+ ...
  q14.*sin((1/2).*t.*theta))).*(4.*((-1).*csc((1/2).*theta).^2.*(q01.*sin( ...
  (1/2).*(1+(-1).*t).*theta)+q11.*sin((1/2).*t.*theta)).*(q02.*sin((1/2).* ...
  (1+(-1).*t).*theta)+q12.*sin((1/2).*t.*theta))+csc((1/2).*theta).^2.*( ...
  q03.*sin((1/2).*(1+(-1).*t).*theta)+q13.*sin((1/2).*t.*theta)).*(q04.* ...
  sin((1/2).*(1+(-1).*t).*theta)+q14.*sin((1/2).*t.*theta))).^2+(1+(-2).*( ...
  csc((1/2).*theta).^2.*(q02.*sin((1/2).*(1+(-1).*t).*theta)+q12.*sin(( ...
  1/2).*t.*theta)).^2+csc((1/2).*theta).^2.*(q03.*sin((1/2).*(1+(-1).*t).* ...
  theta)+q13.*sin((1/2).*t.*theta)).^2)).^2).^(-1/2).*(4.*(csc((1/2).* ...
  theta).^2.*(q01.*sin((1/2).*(1+(-1).*t).*theta)+q11.*sin((1/2).*t.* ...
  theta)).*(q03.*sin((1/2).*(1+(-1).*t).*theta)+q13.*sin((1/2).*t.*theta)) ...
  +csc((1/2).*theta).^2.*(q02.*sin((1/2).*(1+(-1).*t).*theta)+q12.*sin(( ...
  1/2).*t.*theta)).*(q04.*sin((1/2).*(1+(-1).*t).*theta)+q14.*sin((1/2).* ...
  t.*theta))).^2+4.*((-1).*csc((1/2).*theta).^2.*(q01.*sin((1/2).*(1+(-1) ...
  .*t).*theta)+q11.*sin((1/2).*t.*theta)).*(q02.*sin((1/2).*(1+(-1).*t).* ...
  theta)+q12.*sin((1/2).*t.*theta))+csc((1/2).*theta).^2.*(q03.*sin((1/2) ...
  .*(1+(-1).*t).*theta)+q13.*sin((1/2).*t.*theta)).*(q04.*sin((1/2).*(1+( ...
  -1).*t).*theta)+q14.*sin((1/2).*t.*theta))).^2+(1+(-2).*(csc((1/2).* ...
  theta).^2.*(q02.*sin((1/2).*(1+(-1).*t).*theta)+q12.*sin((1/2).*t.* ...
  theta)).^2+csc((1/2).*theta).^2.*(q03.*sin((1/2).*(1+(-1).*t).*theta)+ ...
  q13.*sin((1/2).*t.*theta)).^2)).^2).^(1/2)).*(4.*(csc((1/2).*theta).^2.* ...
  (q02.*sin((1/2).*(1+(-1).*t).*theta)+q12.*sin((1/2).*t.*theta)).*(q03.* ...
  sin((1/2).*(1+(-1).*t).*theta)+q13.*sin((1/2).*t.*theta))+(-1).*csc(( ...
  1/2).*theta).^2.*(q01.*sin((1/2).*(1+(-1).*t).*theta)+q11.*sin((1/2).* ...
  t.*theta)).*(q04.*sin((1/2).*(1+(-1).*t).*theta)+q14.*sin((1/2).*t.* ...
  theta))).^2.*(8.*(((-1/2).*q03.*theta.*cos((1/2).*(1+(-1).*t).*theta)+( ...
  1/2).*q13.*theta.*cos((1/2).*t.*theta)).*csc((1/2).*theta).^2.*(q01.* ...
  sin((1/2).*(1+(-1).*t).*theta)+q11.*sin((1/2).*t.*theta))+((-1/2).*q04.* ...
  theta.*cos((1/2).*(1+(-1).*t).*theta)+(1/2).*q14.*theta.*cos((1/2).*t.* ...
  theta)).*csc((1/2).*theta).^2.*(q02.*sin((1/2).*(1+(-1).*t).*theta)+ ...
  q12.*sin((1/2).*t.*theta))+((-1/2).*q01.*theta.*cos((1/2).*(1+(-1).*t).* ...
  theta)+(1/2).*q11.*theta.*cos((1/2).*t.*theta)).*csc((1/2).*theta).^2.*( ...
  q03.*sin((1/2).*(1+(-1).*t).*theta)+q13.*sin((1/2).*t.*theta))+((-1/2).* ...
  q02.*theta.*cos((1/2).*(1+(-1).*t).*theta)+(1/2).*q12.*theta.*cos((1/2) ...
  .*t.*theta)).*csc((1/2).*theta).^2.*(q04.*sin((1/2).*(1+(-1).*t).*theta) ...
  +q14.*sin((1/2).*t.*theta))).*(csc((1/2).*theta).^2.*(q01.*sin((1/2).*( ...
  1+(-1).*t).*theta)+q11.*sin((1/2).*t.*theta)).*(q03.*sin((1/2).*(1+(-1) ...
  .*t).*theta)+q13.*sin((1/2).*t.*theta))+csc((1/2).*theta).^2.*(q02.*sin( ...
  (1/2).*(1+(-1).*t).*theta)+q12.*sin((1/2).*t.*theta)).*(q04.*sin((1/2).* ...
  (1+(-1).*t).*theta)+q14.*sin((1/2).*t.*theta)))+8.*((-1).*((-1/2).*q02.* ...
  theta.*cos((1/2).*(1+(-1).*t).*theta)+(1/2).*q12.*theta.*cos((1/2).*t.* ...
  theta)).*csc((1/2).*theta).^2.*(q01.*sin((1/2).*(1+(-1).*t).*theta)+ ...
  q11.*sin((1/2).*t.*theta))+(-1).*((-1/2).*q01.*theta.*cos((1/2).*(1+(-1) ...
  .*t).*theta)+(1/2).*q11.*theta.*cos((1/2).*t.*theta)).*csc((1/2).*theta) ...
  .^2.*(q02.*sin((1/2).*(1+(-1).*t).*theta)+q12.*sin((1/2).*t.*theta))+(( ...
  -1/2).*q04.*theta.*cos((1/2).*(1+(-1).*t).*theta)+(1/2).*q14.*theta.* ...
  cos((1/2).*t.*theta)).*csc((1/2).*theta).^2.*(q03.*sin((1/2).*(1+(-1).* ...
  t).*theta)+q13.*sin((1/2).*t.*theta))+((-1/2).*q03.*theta.*cos((1/2).*( ...
  1+(-1).*t).*theta)+(1/2).*q13.*theta.*cos((1/2).*t.*theta)).*csc((1/2).* ...
  theta).^2.*(q04.*sin((1/2).*(1+(-1).*t).*theta)+q14.*sin((1/2).*t.* ...
  theta))).*((-1).*csc((1/2).*theta).^2.*(q01.*sin((1/2).*(1+(-1).*t).* ...
  theta)+q11.*sin((1/2).*t.*theta)).*(q02.*sin((1/2).*(1+(-1).*t).*theta)+ ...
  q12.*sin((1/2).*t.*theta))+csc((1/2).*theta).^2.*(q03.*sin((1/2).*(1+( ...
  -1).*t).*theta)+q13.*sin((1/2).*t.*theta)).*(q04.*sin((1/2).*(1+(-1).*t) ...
  .*theta)+q14.*sin((1/2).*t.*theta)))+(-4).*(2.*((-1/2).*q02.*theta.*cos( ...
  (1/2).*(1+(-1).*t).*theta)+(1/2).*q12.*theta.*cos((1/2).*t.*theta)).* ...
  csc((1/2).*theta).^2.*(q02.*sin((1/2).*(1+(-1).*t).*theta)+q12.*sin(( ...
  1/2).*t.*theta))+2.*((-1/2).*q03.*theta.*cos((1/2).*(1+(-1).*t).*theta)+ ...
  (1/2).*q13.*theta.*cos((1/2).*t.*theta)).*csc((1/2).*theta).^2.*(q03.* ...
  sin((1/2).*(1+(-1).*t).*theta)+q13.*sin((1/2).*t.*theta))).*(1+(-2).*( ...
  csc((1/2).*theta).^2.*(q02.*sin((1/2).*(1+(-1).*t).*theta)+q12.*sin(( ...
  1/2).*t.*theta)).^2+csc((1/2).*theta).^2.*(q03.*sin((1/2).*(1+(-1).*t).* ...
  theta)+q13.*sin((1/2).*t.*theta)).^2))).*(4.*((-1).*csc((1/2).*theta) ...
  .^2.*(q01.*sin((1/2).*(1+(-1).*t).*theta)+q11.*sin((1/2).*t.*theta)).*( ...
  q02.*sin((1/2).*(1+(-1).*t).*theta)+q12.*sin((1/2).*t.*theta))+csc((1/2) ...
  .*theta).^2.*(q03.*sin((1/2).*(1+(-1).*t).*theta)+q13.*sin((1/2).*t.* ...
  theta)).*(q04.*sin((1/2).*(1+(-1).*t).*theta)+q14.*sin((1/2).*t.*theta)) ...
  ).^2+(1+(-2).*(csc((1/2).*theta).^2.*(q02.*sin((1/2).*(1+(-1).*t).* ...
  theta)+q12.*sin((1/2).*t.*theta)).^2+csc((1/2).*theta).^2.*(q03.*sin(( ...
  1/2).*(1+(-1).*t).*theta)+q13.*sin((1/2).*t.*theta)).^2)).^2).^(-1)+(1+( ...
  -2).*(csc((1/2).*theta).^2.*(q03.*sin((1/2).*(1+(-1).*t).*theta)+q13.* ...
  sin((1/2).*t.*theta)).^2+csc((1/2).*theta).^2.*(q04.*sin((1/2).*(1+(-1) ...
  .*t).*theta)+q14.*sin((1/2).*t.*theta)).^2)).^2.*(8.*(((-1/2).*q03.* ...
  theta.*cos((1/2).*(1+(-1).*t).*theta)+(1/2).*q13.*theta.*cos((1/2).*t.* ...
  theta)).*csc((1/2).*theta).^2.*(q01.*sin((1/2).*(1+(-1).*t).*theta)+ ...
  q11.*sin((1/2).*t.*theta))+((-1/2).*q04.*theta.*cos((1/2).*(1+(-1).*t).* ...
  theta)+(1/2).*q14.*theta.*cos((1/2).*t.*theta)).*csc((1/2).*theta).^2.*( ...
  q02.*sin((1/2).*(1+(-1).*t).*theta)+q12.*sin((1/2).*t.*theta))+((-1/2).* ...
  q01.*theta.*cos((1/2).*(1+(-1).*t).*theta)+(1/2).*q11.*theta.*cos((1/2) ...
  .*t.*theta)).*csc((1/2).*theta).^2.*(q03.*sin((1/2).*(1+(-1).*t).*theta) ...
  +q13.*sin((1/2).*t.*theta))+((-1/2).*q02.*theta.*cos((1/2).*(1+(-1).*t) ...
  .*theta)+(1/2).*q12.*theta.*cos((1/2).*t.*theta)).*csc((1/2).*theta) ...
  .^2.*(q04.*sin((1/2).*(1+(-1).*t).*theta)+q14.*sin((1/2).*t.*theta))).*( ...
  csc((1/2).*theta).^2.*(q01.*sin((1/2).*(1+(-1).*t).*theta)+q11.*sin(( ...
  1/2).*t.*theta)).*(q03.*sin((1/2).*(1+(-1).*t).*theta)+q13.*sin((1/2).* ...
  t.*theta))+csc((1/2).*theta).^2.*(q02.*sin((1/2).*(1+(-1).*t).*theta)+ ...
  q12.*sin((1/2).*t.*theta)).*(q04.*sin((1/2).*(1+(-1).*t).*theta)+q14.* ...
  sin((1/2).*t.*theta)))+8.*((-1).*((-1/2).*q02.*theta.*cos((1/2).*(1+(-1) ...
  .*t).*theta)+(1/2).*q12.*theta.*cos((1/2).*t.*theta)).*csc((1/2).*theta) ...
  .^2.*(q01.*sin((1/2).*(1+(-1).*t).*theta)+q11.*sin((1/2).*t.*theta))+( ...
  -1).*((-1/2).*q01.*theta.*cos((1/2).*(1+(-1).*t).*theta)+(1/2).*q11.* ...
  theta.*cos((1/2).*t.*theta)).*csc((1/2).*theta).^2.*(q02.*sin((1/2).*(1+ ...
  (-1).*t).*theta)+q12.*sin((1/2).*t.*theta))+((-1/2).*q04.*theta.*cos(( ...
  1/2).*(1+(-1).*t).*theta)+(1/2).*q14.*theta.*cos((1/2).*t.*theta)).*csc( ...
  (1/2).*theta).^2.*(q03.*sin((1/2).*(1+(-1).*t).*theta)+q13.*sin((1/2).* ...
  t.*theta))+((-1/2).*q03.*theta.*cos((1/2).*(1+(-1).*t).*theta)+(1/2).* ...
  q13.*theta.*cos((1/2).*t.*theta)).*csc((1/2).*theta).^2.*(q04.*sin((1/2) ...
  .*(1+(-1).*t).*theta)+q14.*sin((1/2).*t.*theta))).*((-1).*csc((1/2).* ...
  theta).^2.*(q01.*sin((1/2).*(1+(-1).*t).*theta)+q11.*sin((1/2).*t.* ...
  theta)).*(q02.*sin((1/2).*(1+(-1).*t).*theta)+q12.*sin((1/2).*t.*theta)) ...
  +csc((1/2).*theta).^2.*(q03.*sin((1/2).*(1+(-1).*t).*theta)+q13.*sin(( ...
  1/2).*t.*theta)).*(q04.*sin((1/2).*(1+(-1).*t).*theta)+q14.*sin((1/2).* ...
  t.*theta)))+(-4).*(2.*((-1/2).*q02.*theta.*cos((1/2).*(1+(-1).*t).* ...
  theta)+(1/2).*q12.*theta.*cos((1/2).*t.*theta)).*csc((1/2).*theta).^2.*( ...
  q02.*sin((1/2).*(1+(-1).*t).*theta)+q12.*sin((1/2).*t.*theta))+2.*(( ...
  -1/2).*q03.*theta.*cos((1/2).*(1+(-1).*t).*theta)+(1/2).*q13.*theta.* ...
  cos((1/2).*t.*theta)).*csc((1/2).*theta).^2.*(q03.*sin((1/2).*(1+(-1).* ...
  t).*theta)+q13.*sin((1/2).*t.*theta))).*(1+(-2).*(csc((1/2).*theta).^2.* ...
  (q02.*sin((1/2).*(1+(-1).*t).*theta)+q12.*sin((1/2).*t.*theta)).^2+csc(( ...
  1/2).*theta).^2.*(q03.*sin((1/2).*(1+(-1).*t).*theta)+q13.*sin((1/2).* ...
  t.*theta)).^2))).*(4.*((-1).*csc((1/2).*theta).^2.*(q01.*sin((1/2).*(1+( ...
  -1).*t).*theta)+q11.*sin((1/2).*t.*theta)).*(q02.*sin((1/2).*(1+(-1).*t) ...
  .*theta)+q12.*sin((1/2).*t.*theta))+csc((1/2).*theta).^2.*(q03.*sin(( ...
  1/2).*(1+(-1).*t).*theta)+q13.*sin((1/2).*t.*theta)).*(q04.*sin((1/2).*( ...
  1+(-1).*t).*theta)+q14.*sin((1/2).*t.*theta))).^2+(1+(-2).*(csc((1/2).* ...
  theta).^2.*(q02.*sin((1/2).*(1+(-1).*t).*theta)+q12.*sin((1/2).*t.* ...
  theta)).^2+csc((1/2).*theta).^2.*(q03.*sin((1/2).*(1+(-1).*t).*theta)+ ...
  q13.*sin((1/2).*t.*theta)).^2)).^2).^(-1)+(-4).*(csc((1/2).*theta).^2.*( ...
  q02.*sin((1/2).*(1+(-1).*t).*theta)+q12.*sin((1/2).*t.*theta)).*(q03.* ...
  sin((1/2).*(1+(-1).*t).*theta)+q13.*sin((1/2).*t.*theta))+(-1).*csc(( ...
  1/2).*theta).^2.*(q01.*sin((1/2).*(1+(-1).*t).*theta)+q11.*sin((1/2).* ...
  t.*theta)).*(q04.*sin((1/2).*(1+(-1).*t).*theta)+q14.*sin((1/2).*t.* ...
  theta))).^2.*(8.*((-1).*((-1/2).*q02.*theta.*cos((1/2).*(1+(-1).*t).* ...
  theta)+(1/2).*q12.*theta.*cos((1/2).*t.*theta)).*csc((1/2).*theta).^2.*( ...
  q01.*sin((1/2).*(1+(-1).*t).*theta)+q11.*sin((1/2).*t.*theta))+(-1).*(( ...
  -1/2).*q01.*theta.*cos((1/2).*(1+(-1).*t).*theta)+(1/2).*q11.*theta.* ...
  cos((1/2).*t.*theta)).*csc((1/2).*theta).^2.*(q02.*sin((1/2).*(1+(-1).* ...
  t).*theta)+q12.*sin((1/2).*t.*theta))+((-1/2).*q04.*theta.*cos((1/2).*( ...
  1+(-1).*t).*theta)+(1/2).*q14.*theta.*cos((1/2).*t.*theta)).*csc((1/2).* ...
  theta).^2.*(q03.*sin((1/2).*(1+(-1).*t).*theta)+q13.*sin((1/2).*t.* ...
  theta))+((-1/2).*q03.*theta.*cos((1/2).*(1+(-1).*t).*theta)+(1/2).*q13.* ...
  theta.*cos((1/2).*t.*theta)).*csc((1/2).*theta).^2.*(q04.*sin((1/2).*(1+ ...
  (-1).*t).*theta)+q14.*sin((1/2).*t.*theta))).*((-1).*csc((1/2).*theta) ...
  .^2.*(q01.*sin((1/2).*(1+(-1).*t).*theta)+q11.*sin((1/2).*t.*theta)).*( ...
  q02.*sin((1/2).*(1+(-1).*t).*theta)+q12.*sin((1/2).*t.*theta))+csc((1/2) ...
  .*theta).^2.*(q03.*sin((1/2).*(1+(-1).*t).*theta)+q13.*sin((1/2).*t.* ...
  theta)).*(q04.*sin((1/2).*(1+(-1).*t).*theta)+q14.*sin((1/2).*t.*theta)) ...
  )+(-4).*(2.*((-1/2).*q02.*theta.*cos((1/2).*(1+(-1).*t).*theta)+(1/2).* ...
  q12.*theta.*cos((1/2).*t.*theta)).*csc((1/2).*theta).^2.*(q02.*sin((1/2) ...
  .*(1+(-1).*t).*theta)+q12.*sin((1/2).*t.*theta))+2.*((-1/2).*q03.* ...
  theta.*cos((1/2).*(1+(-1).*t).*theta)+(1/2).*q13.*theta.*cos((1/2).*t.* ...
  theta)).*csc((1/2).*theta).^2.*(q03.*sin((1/2).*(1+(-1).*t).*theta)+ ...
  q13.*sin((1/2).*t.*theta))).*(1+(-2).*(csc((1/2).*theta).^2.*(q02.*sin(( ...
  1/2).*(1+(-1).*t).*theta)+q12.*sin((1/2).*t.*theta)).^2+csc((1/2).* ...
  theta).^2.*(q03.*sin((1/2).*(1+(-1).*t).*theta)+q13.*sin((1/2).*t.* ...
  theta)).^2))).*(4.*((-1).*csc((1/2).*theta).^2.*(q01.*sin((1/2).*(1+(-1) ...
  .*t).*theta)+q11.*sin((1/2).*t.*theta)).*(q02.*sin((1/2).*(1+(-1).*t).* ...
  theta)+q12.*sin((1/2).*t.*theta))+csc((1/2).*theta).^2.*(q03.*sin((1/2) ...
  .*(1+(-1).*t).*theta)+q13.*sin((1/2).*t.*theta)).*(q04.*sin((1/2).*(1+( ...
  -1).*t).*theta)+q14.*sin((1/2).*t.*theta))).^2+(1+(-2).*(csc((1/2).* ...
  theta).^2.*(q02.*sin((1/2).*(1+(-1).*t).*theta)+q12.*sin((1/2).*t.* ...
  theta)).^2+csc((1/2).*theta).^2.*(q03.*sin((1/2).*(1+(-1).*t).*theta)+ ...
  q13.*sin((1/2).*t.*theta)).^2)).^2).^(-2).*(4.*(csc((1/2).*theta).^2.*( ...
  q01.*sin((1/2).*(1+(-1).*t).*theta)+q11.*sin((1/2).*t.*theta)).*(q03.* ...
  sin((1/2).*(1+(-1).*t).*theta)+q13.*sin((1/2).*t.*theta))+csc((1/2).* ...
  theta).^2.*(q02.*sin((1/2).*(1+(-1).*t).*theta)+q12.*sin((1/2).*t.* ...
  theta)).*(q04.*sin((1/2).*(1+(-1).*t).*theta)+q14.*sin((1/2).*t.*theta)) ...
  ).^2+4.*((-1).*csc((1/2).*theta).^2.*(q01.*sin((1/2).*(1+(-1).*t).* ...
  theta)+q11.*sin((1/2).*t.*theta)).*(q02.*sin((1/2).*(1+(-1).*t).*theta)+ ...
  q12.*sin((1/2).*t.*theta))+csc((1/2).*theta).^2.*(q03.*sin((1/2).*(1+( ...
  -1).*t).*theta)+q13.*sin((1/2).*t.*theta)).*(q04.*sin((1/2).*(1+(-1).*t) ...
  .*theta)+q14.*sin((1/2).*t.*theta))).^2+(1+(-2).*(csc((1/2).*theta).^2.* ...
  (q02.*sin((1/2).*(1+(-1).*t).*theta)+q12.*sin((1/2).*t.*theta)).^2+csc(( ...
  1/2).*theta).^2.*(q03.*sin((1/2).*(1+(-1).*t).*theta)+q13.*sin((1/2).* ...
  t.*theta)).^2)).^2)+(-1).*(1+(-2).*(csc((1/2).*theta).^2.*(q03.*sin(( ...
  1/2).*(1+(-1).*t).*theta)+q13.*sin((1/2).*t.*theta)).^2+csc((1/2).* ...
  theta).^2.*(q04.*sin((1/2).*(1+(-1).*t).*theta)+q14.*sin((1/2).*t.* ...
  theta)).^2)).^2.*(8.*((-1).*((-1/2).*q02.*theta.*cos((1/2).*(1+(-1).*t) ...
  .*theta)+(1/2).*q12.*theta.*cos((1/2).*t.*theta)).*csc((1/2).*theta) ...
  .^2.*(q01.*sin((1/2).*(1+(-1).*t).*theta)+q11.*sin((1/2).*t.*theta))+( ...
  -1).*((-1/2).*q01.*theta.*cos((1/2).*(1+(-1).*t).*theta)+(1/2).*q11.* ...
  theta.*cos((1/2).*t.*theta)).*csc((1/2).*theta).^2.*(q02.*sin((1/2).*(1+ ...
  (-1).*t).*theta)+q12.*sin((1/2).*t.*theta))+((-1/2).*q04.*theta.*cos(( ...
  1/2).*(1+(-1).*t).*theta)+(1/2).*q14.*theta.*cos((1/2).*t.*theta)).*csc( ...
  (1/2).*theta).^2.*(q03.*sin((1/2).*(1+(-1).*t).*theta)+q13.*sin((1/2).* ...
  t.*theta))+((-1/2).*q03.*theta.*cos((1/2).*(1+(-1).*t).*theta)+(1/2).* ...
  q13.*theta.*cos((1/2).*t.*theta)).*csc((1/2).*theta).^2.*(q04.*sin((1/2) ...
  .*(1+(-1).*t).*theta)+q14.*sin((1/2).*t.*theta))).*((-1).*csc((1/2).* ...
  theta).^2.*(q01.*sin((1/2).*(1+(-1).*t).*theta)+q11.*sin((1/2).*t.* ...
  theta)).*(q02.*sin((1/2).*(1+(-1).*t).*theta)+q12.*sin((1/2).*t.*theta)) ...
  +csc((1/2).*theta).^2.*(q03.*sin((1/2).*(1+(-1).*t).*theta)+q13.*sin(( ...
  1/2).*t.*theta)).*(q04.*sin((1/2).*(1+(-1).*t).*theta)+q14.*sin((1/2).* ...
  t.*theta)))+(-4).*(2.*((-1/2).*q02.*theta.*cos((1/2).*(1+(-1).*t).* ...
  theta)+(1/2).*q12.*theta.*cos((1/2).*t.*theta)).*csc((1/2).*theta).^2.*( ...
  q02.*sin((1/2).*(1+(-1).*t).*theta)+q12.*sin((1/2).*t.*theta))+2.*(( ...
  -1/2).*q03.*theta.*cos((1/2).*(1+(-1).*t).*theta)+(1/2).*q13.*theta.* ...
  cos((1/2).*t.*theta)).*csc((1/2).*theta).^2.*(q03.*sin((1/2).*(1+(-1).* ...
  t).*theta)+q13.*sin((1/2).*t.*theta))).*(1+(-2).*(csc((1/2).*theta).^2.* ...
  (q02.*sin((1/2).*(1+(-1).*t).*theta)+q12.*sin((1/2).*t.*theta)).^2+csc(( ...
  1/2).*theta).^2.*(q03.*sin((1/2).*(1+(-1).*t).*theta)+q13.*sin((1/2).* ...
  t.*theta)).^2))).*(4.*((-1).*csc((1/2).*theta).^2.*(q01.*sin((1/2).*(1+( ...
  -1).*t).*theta)+q11.*sin((1/2).*t.*theta)).*(q02.*sin((1/2).*(1+(-1).*t) ...
  .*theta)+q12.*sin((1/2).*t.*theta))+csc((1/2).*theta).^2.*(q03.*sin(( ...
  1/2).*(1+(-1).*t).*theta)+q13.*sin((1/2).*t.*theta)).*(q04.*sin((1/2).*( ...
  1+(-1).*t).*theta)+q14.*sin((1/2).*t.*theta))).^2+(1+(-2).*(csc((1/2).* ...
  theta).^2.*(q02.*sin((1/2).*(1+(-1).*t).*theta)+q12.*sin((1/2).*t.* ...
  theta)).^2+csc((1/2).*theta).^2.*(q03.*sin((1/2).*(1+(-1).*t).*theta)+ ...
  q13.*sin((1/2).*t.*theta)).^2)).^2).^(-2).*(4.*(csc((1/2).*theta).^2.*( ...
  q01.*sin((1/2).*(1+(-1).*t).*theta)+q11.*sin((1/2).*t.*theta)).*(q03.* ...
  sin((1/2).*(1+(-1).*t).*theta)+q13.*sin((1/2).*t.*theta))+csc((1/2).* ...
  theta).^2.*(q02.*sin((1/2).*(1+(-1).*t).*theta)+q12.*sin((1/2).*t.* ...
  theta)).*(q04.*sin((1/2).*(1+(-1).*t).*theta)+q14.*sin((1/2).*t.*theta)) ...
  ).^2+4.*((-1).*csc((1/2).*theta).^2.*(q01.*sin((1/2).*(1+(-1).*t).* ...
  theta)+q11.*sin((1/2).*t.*theta)).*(q02.*sin((1/2).*(1+(-1).*t).*theta)+ ...
  q12.*sin((1/2).*t.*theta))+csc((1/2).*theta).^2.*(q03.*sin((1/2).*(1+( ...
  -1).*t).*theta)+q13.*sin((1/2).*t.*theta)).*(q04.*sin((1/2).*(1+(-1).*t) ...
  .*theta)+q14.*sin((1/2).*t.*theta))).^2+(1+(-2).*(csc((1/2).*theta).^2.* ...
  (q02.*sin((1/2).*(1+(-1).*t).*theta)+q12.*sin((1/2).*t.*theta)).^2+csc(( ...
  1/2).*theta).^2.*(q03.*sin((1/2).*(1+(-1).*t).*theta)+q13.*sin((1/2).* ...
  t.*theta)).^2)).^2)+8.*((-1).*((-1/2).*q04.*theta.*cos((1/2).*(1+(-1).* ...
  t).*theta)+(1/2).*q14.*theta.*cos((1/2).*t.*theta)).*csc((1/2).*theta) ...
  .^2.*(q01.*sin((1/2).*(1+(-1).*t).*theta)+q11.*sin((1/2).*t.*theta))+(( ...
  -1/2).*q03.*theta.*cos((1/2).*(1+(-1).*t).*theta)+(1/2).*q13.*theta.* ...
  cos((1/2).*t.*theta)).*csc((1/2).*theta).^2.*(q02.*sin((1/2).*(1+(-1).* ...
  t).*theta)+q12.*sin((1/2).*t.*theta))+((-1/2).*q02.*theta.*cos((1/2).*( ...
  1+(-1).*t).*theta)+(1/2).*q12.*theta.*cos((1/2).*t.*theta)).*csc((1/2).* ...
  theta).^2.*(q03.*sin((1/2).*(1+(-1).*t).*theta)+q13.*sin((1/2).*t.* ...
  theta))+(-1).*((-1/2).*q01.*theta.*cos((1/2).*(1+(-1).*t).*theta)+(1/2) ...
  .*q11.*theta.*cos((1/2).*t.*theta)).*csc((1/2).*theta).^2.*(q04.*sin(( ...
  1/2).*(1+(-1).*t).*theta)+q14.*sin((1/2).*t.*theta))).*(csc((1/2).* ...
  theta).^2.*(q02.*sin((1/2).*(1+(-1).*t).*theta)+q12.*sin((1/2).*t.* ...
  theta)).*(q03.*sin((1/2).*(1+(-1).*t).*theta)+q13.*sin((1/2).*t.*theta)) ...
  +(-1).*csc((1/2).*theta).^2.*(q01.*sin((1/2).*(1+(-1).*t).*theta)+q11.* ...
  sin((1/2).*t.*theta)).*(q04.*sin((1/2).*(1+(-1).*t).*theta)+q14.*sin(( ...
  1/2).*t.*theta))).*(4.*((-1).*csc((1/2).*theta).^2.*(q01.*sin((1/2).*(1+ ...
  (-1).*t).*theta)+q11.*sin((1/2).*t.*theta)).*(q02.*sin((1/2).*(1+(-1).* ...
  t).*theta)+q12.*sin((1/2).*t.*theta))+csc((1/2).*theta).^2.*(q03.*sin(( ...
  1/2).*(1+(-1).*t).*theta)+q13.*sin((1/2).*t.*theta)).*(q04.*sin((1/2).*( ...
  1+(-1).*t).*theta)+q14.*sin((1/2).*t.*theta))).^2+(1+(-2).*(csc((1/2).* ...
  theta).^2.*(q02.*sin((1/2).*(1+(-1).*t).*theta)+q12.*sin((1/2).*t.* ...
  theta)).^2+csc((1/2).*theta).^2.*(q03.*sin((1/2).*(1+(-1).*t).*theta)+ ...
  q13.*sin((1/2).*t.*theta)).^2)).^2).^(-1).*(4.*(csc((1/2).*theta).^2.*( ...
  q01.*sin((1/2).*(1+(-1).*t).*theta)+q11.*sin((1/2).*t.*theta)).*(q03.* ...
  sin((1/2).*(1+(-1).*t).*theta)+q13.*sin((1/2).*t.*theta))+csc((1/2).* ...
  theta).^2.*(q02.*sin((1/2).*(1+(-1).*t).*theta)+q12.*sin((1/2).*t.* ...
  theta)).*(q04.*sin((1/2).*(1+(-1).*t).*theta)+q14.*sin((1/2).*t.*theta)) ...
  ).^2+4.*((-1).*csc((1/2).*theta).^2.*(q01.*sin((1/2).*(1+(-1).*t).* ...
  theta)+q11.*sin((1/2).*t.*theta)).*(q02.*sin((1/2).*(1+(-1).*t).*theta)+ ...
  q12.*sin((1/2).*t.*theta))+csc((1/2).*theta).^2.*(q03.*sin((1/2).*(1+( ...
  -1).*t).*theta)+q13.*sin((1/2).*t.*theta)).*(q04.*sin((1/2).*(1+(-1).*t) ...
  .*theta)+q14.*sin((1/2).*t.*theta))).^2+(1+(-2).*(csc((1/2).*theta).^2.* ...
  (q02.*sin((1/2).*(1+(-1).*t).*theta)+q12.*sin((1/2).*t.*theta)).^2+csc(( ...
  1/2).*theta).^2.*(q03.*sin((1/2).*(1+(-1).*t).*theta)+q13.*sin((1/2).* ...
  t.*theta)).^2)).^2)+(-4).*(2.*((-1/2).*q03.*theta.*cos((1/2).*(1+(-1).* ...
  t).*theta)+(1/2).*q13.*theta.*cos((1/2).*t.*theta)).*csc((1/2).*theta) ...
  .^2.*(q03.*sin((1/2).*(1+(-1).*t).*theta)+q13.*sin((1/2).*t.*theta))+2.* ...
  ((-1/2).*q04.*theta.*cos((1/2).*(1+(-1).*t).*theta)+(1/2).*q14.*theta.* ...
  cos((1/2).*t.*theta)).*csc((1/2).*theta).^2.*(q04.*sin((1/2).*(1+(-1).* ...
  t).*theta)+q14.*sin((1/2).*t.*theta))).*(1+(-2).*(csc((1/2).*theta).^2.* ...
  (q03.*sin((1/2).*(1+(-1).*t).*theta)+q13.*sin((1/2).*t.*theta)).^2+csc(( ...
  1/2).*theta).^2.*(q04.*sin((1/2).*(1+(-1).*t).*theta)+q14.*sin((1/2).* ...
  t.*theta)).^2)).*(4.*((-1).*csc((1/2).*theta).^2.*(q01.*sin((1/2).*(1+( ...
  -1).*t).*theta)+q11.*sin((1/2).*t.*theta)).*(q02.*sin((1/2).*(1+(-1).*t) ...
  .*theta)+q12.*sin((1/2).*t.*theta))+csc((1/2).*theta).^2.*(q03.*sin(( ...
  1/2).*(1+(-1).*t).*theta)+q13.*sin((1/2).*t.*theta)).*(q04.*sin((1/2).*( ...
  1+(-1).*t).*theta)+q14.*sin((1/2).*t.*theta))).^2+(1+(-2).*(csc((1/2).* ...
  theta).^2.*(q02.*sin((1/2).*(1+(-1).*t).*theta)+q12.*sin((1/2).*t.* ...
  theta)).^2+csc((1/2).*theta).^2.*(q03.*sin((1/2).*(1+(-1).*t).*theta)+ ...
  q13.*sin((1/2).*t.*theta)).^2)).^2).^(-1).*(4.*(csc((1/2).*theta).^2.*( ...
  q01.*sin((1/2).*(1+(-1).*t).*theta)+q11.*sin((1/2).*t.*theta)).*(q03.* ...
  sin((1/2).*(1+(-1).*t).*theta)+q13.*sin((1/2).*t.*theta))+csc((1/2).* ...
  theta).^2.*(q02.*sin((1/2).*(1+(-1).*t).*theta)+q12.*sin((1/2).*t.* ...
  theta)).*(q04.*sin((1/2).*(1+(-1).*t).*theta)+q14.*sin((1/2).*t.*theta)) ...
  ).^2+4.*((-1).*csc((1/2).*theta).^2.*(q01.*sin((1/2).*(1+(-1).*t).* ...
  theta)+q11.*sin((1/2).*t.*theta)).*(q02.*sin((1/2).*(1+(-1).*t).*theta)+ ...
  q12.*sin((1/2).*t.*theta))+csc((1/2).*theta).^2.*(q03.*sin((1/2).*(1+( ...
  -1).*t).*theta)+q13.*sin((1/2).*t.*theta)).*(q04.*sin((1/2).*(1+(-1).*t) ...
  .*theta)+q14.*sin((1/2).*t.*theta))).^2+(1+(-2).*(csc((1/2).*theta).^2.* ...
  (q02.*sin((1/2).*(1+(-1).*t).*theta)+q12.*sin((1/2).*t.*theta)).^2+csc(( ...
  1/2).*theta).^2.*(q03.*sin((1/2).*(1+(-1).*t).*theta)+q13.*sin((1/2).* ...
  t.*theta)).^2)).^2)).*(4.*(csc((1/2).*theta).^2.*(q02.*sin((1/2).*(1+( ...
  -1).*t).*theta)+q12.*sin((1/2).*t.*theta)).*(q03.*sin((1/2).*(1+(-1).*t) ...
  .*theta)+q13.*sin((1/2).*t.*theta))+(-1).*csc((1/2).*theta).^2.*(q01.* ...
  sin((1/2).*(1+(-1).*t).*theta)+q11.*sin((1/2).*t.*theta)).*(q04.*sin(( ...
  1/2).*(1+(-1).*t).*theta)+q14.*sin((1/2).*t.*theta))).^2.*(4.*((-1).* ...
  csc((1/2).*theta).^2.*(q01.*sin((1/2).*(1+(-1).*t).*theta)+q11.*sin(( ...
  1/2).*t.*theta)).*(q02.*sin((1/2).*(1+(-1).*t).*theta)+q12.*sin((1/2).* ...
  t.*theta))+csc((1/2).*theta).^2.*(q03.*sin((1/2).*(1+(-1).*t).*theta)+ ...
  q13.*sin((1/2).*t.*theta)).*(q04.*sin((1/2).*(1+(-1).*t).*theta)+q14.* ...
  sin((1/2).*t.*theta))).^2+(1+(-2).*(csc((1/2).*theta).^2.*(q02.*sin(( ...
  1/2).*(1+(-1).*t).*theta)+q12.*sin((1/2).*t.*theta)).^2+csc((1/2).* ...
  theta).^2.*(q03.*sin((1/2).*(1+(-1).*t).*theta)+q13.*sin((1/2).*t.* ...
  theta)).^2)).^2).^(-1).*(4.*(csc((1/2).*theta).^2.*(q01.*sin((1/2).*(1+( ...
  -1).*t).*theta)+q11.*sin((1/2).*t.*theta)).*(q03.*sin((1/2).*(1+(-1).*t) ...
  .*theta)+q13.*sin((1/2).*t.*theta))+csc((1/2).*theta).^2.*(q02.*sin(( ...
  1/2).*(1+(-1).*t).*theta)+q12.*sin((1/2).*t.*theta)).*(q04.*sin((1/2).*( ...
  1+(-1).*t).*theta)+q14.*sin((1/2).*t.*theta))).^2+4.*((-1).*csc((1/2).* ...
  theta).^2.*(q01.*sin((1/2).*(1+(-1).*t).*theta)+q11.*sin((1/2).*t.* ...
  theta)).*(q02.*sin((1/2).*(1+(-1).*t).*theta)+q12.*sin((1/2).*t.*theta)) ...
  +csc((1/2).*theta).^2.*(q03.*sin((1/2).*(1+(-1).*t).*theta)+q13.*sin(( ...
  1/2).*t.*theta)).*(q04.*sin((1/2).*(1+(-1).*t).*theta)+q14.*sin((1/2).* ...
  t.*theta))).^2+(1+(-2).*(csc((1/2).*theta).^2.*(q02.*sin((1/2).*(1+(-1) ...
  .*t).*theta)+q12.*sin((1/2).*t.*theta)).^2+csc((1/2).*theta).^2.*(q03.* ...
  sin((1/2).*(1+(-1).*t).*theta)+q13.*sin((1/2).*t.*theta)).^2)).^2)+(1+( ...
  -2).*(csc((1/2).*theta).^2.*(q03.*sin((1/2).*(1+(-1).*t).*theta)+q13.* ...
  sin((1/2).*t.*theta)).^2+csc((1/2).*theta).^2.*(q04.*sin((1/2).*(1+(-1) ...
  .*t).*theta)+q14.*sin((1/2).*t.*theta)).^2)).^2.*(4.*((-1).*csc((1/2).* ...
  theta).^2.*(q01.*sin((1/2).*(1+(-1).*t).*theta)+q11.*sin((1/2).*t.* ...
  theta)).*(q02.*sin((1/2).*(1+(-1).*t).*theta)+q12.*sin((1/2).*t.*theta)) ...
  +csc((1/2).*theta).^2.*(q03.*sin((1/2).*(1+(-1).*t).*theta)+q13.*sin(( ...
  1/2).*t.*theta)).*(q04.*sin((1/2).*(1+(-1).*t).*theta)+q14.*sin((1/2).* ...
  t.*theta))).^2+(1+(-2).*(csc((1/2).*theta).^2.*(q02.*sin((1/2).*(1+(-1) ...
  .*t).*theta)+q12.*sin((1/2).*t.*theta)).^2+csc((1/2).*theta).^2.*(q03.* ...
  sin((1/2).*(1+(-1).*t).*theta)+q13.*sin((1/2).*t.*theta)).^2)).^2).^(-1) ...
  .*(4.*(csc((1/2).*theta).^2.*(q01.*sin((1/2).*(1+(-1).*t).*theta)+q11.* ...
  sin((1/2).*t.*theta)).*(q03.*sin((1/2).*(1+(-1).*t).*theta)+q13.*sin(( ...
  1/2).*t.*theta))+csc((1/2).*theta).^2.*(q02.*sin((1/2).*(1+(-1).*t).* ...
  theta)+q12.*sin((1/2).*t.*theta)).*(q04.*sin((1/2).*(1+(-1).*t).*theta)+ ...
  q14.*sin((1/2).*t.*theta))).^2+4.*((-1).*csc((1/2).*theta).^2.*(q01.* ...
  sin((1/2).*(1+(-1).*t).*theta)+q11.*sin((1/2).*t.*theta)).*(q02.*sin(( ...
  1/2).*(1+(-1).*t).*theta)+q12.*sin((1/2).*t.*theta))+csc((1/2).*theta) ...
  .^2.*(q03.*sin((1/2).*(1+(-1).*t).*theta)+q13.*sin((1/2).*t.*theta)).*( ...
  q04.*sin((1/2).*(1+(-1).*t).*theta)+q14.*sin((1/2).*t.*theta))).^2+(1+( ...
  -2).*(csc((1/2).*theta).^2.*(q02.*sin((1/2).*(1+(-1).*t).*theta)+q12.* ...
  sin((1/2).*t.*theta)).^2+csc((1/2).*theta).^2.*(q03.*sin((1/2).*(1+(-1) ...
  .*t).*theta)+q13.*sin((1/2).*t.*theta)).^2)).^2)).^(-2)+(1/2).*(1+(-2).* ...
  (csc((1/2).*theta).^2.*(q03.*sin((1/2).*(1+(-1).*t).*theta)+q13.*sin(( ...
  1/2).*t.*theta)).^2+csc((1/2).*theta).^2.*(q04.*sin((1/2).*(1+(-1).*t).* ...
  theta)+q14.*sin((1/2).*t.*theta)).^2)).*(8.*(((-1/2).*q03.*theta.*cos(( ...
  1/2).*(1+(-1).*t).*theta)+(1/2).*q13.*theta.*cos((1/2).*t.*theta)).*csc( ...
  (1/2).*theta).^2.*(q01.*sin((1/2).*(1+(-1).*t).*theta)+q11.*sin((1/2).* ...
  t.*theta))+((-1/2).*q04.*theta.*cos((1/2).*(1+(-1).*t).*theta)+(1/2).* ...
  q14.*theta.*cos((1/2).*t.*theta)).*csc((1/2).*theta).^2.*(q02.*sin((1/2) ...
  .*(1+(-1).*t).*theta)+q12.*sin((1/2).*t.*theta))+((-1/2).*q01.*theta.* ...
  cos((1/2).*(1+(-1).*t).*theta)+(1/2).*q11.*theta.*cos((1/2).*t.*theta)) ...
  .*csc((1/2).*theta).^2.*(q03.*sin((1/2).*(1+(-1).*t).*theta)+q13.*sin(( ...
  1/2).*t.*theta))+((-1/2).*q02.*theta.*cos((1/2).*(1+(-1).*t).*theta)+( ...
  1/2).*q12.*theta.*cos((1/2).*t.*theta)).*csc((1/2).*theta).^2.*(q04.* ...
  sin((1/2).*(1+(-1).*t).*theta)+q14.*sin((1/2).*t.*theta))).*(csc((1/2).* ...
  theta).^2.*(q01.*sin((1/2).*(1+(-1).*t).*theta)+q11.*sin((1/2).*t.* ...
  theta)).*(q03.*sin((1/2).*(1+(-1).*t).*theta)+q13.*sin((1/2).*t.*theta)) ...
  +csc((1/2).*theta).^2.*(q02.*sin((1/2).*(1+(-1).*t).*theta)+q12.*sin(( ...
  1/2).*t.*theta)).*(q04.*sin((1/2).*(1+(-1).*t).*theta)+q14.*sin((1/2).* ...
  t.*theta)))+8.*((-1).*((-1/2).*q02.*theta.*cos((1/2).*(1+(-1).*t).* ...
  theta)+(1/2).*q12.*theta.*cos((1/2).*t.*theta)).*csc((1/2).*theta).^2.*( ...
  q01.*sin((1/2).*(1+(-1).*t).*theta)+q11.*sin((1/2).*t.*theta))+(-1).*(( ...
  -1/2).*q01.*theta.*cos((1/2).*(1+(-1).*t).*theta)+(1/2).*q11.*theta.* ...
  cos((1/2).*t.*theta)).*csc((1/2).*theta).^2.*(q02.*sin((1/2).*(1+(-1).* ...
  t).*theta)+q12.*sin((1/2).*t.*theta))+((-1/2).*q04.*theta.*cos((1/2).*( ...
  1+(-1).*t).*theta)+(1/2).*q14.*theta.*cos((1/2).*t.*theta)).*csc((1/2).* ...
  theta).^2.*(q03.*sin((1/2).*(1+(-1).*t).*theta)+q13.*sin((1/2).*t.* ...
  theta))+((-1/2).*q03.*theta.*cos((1/2).*(1+(-1).*t).*theta)+(1/2).*q13.* ...
  theta.*cos((1/2).*t.*theta)).*csc((1/2).*theta).^2.*(q04.*sin((1/2).*(1+ ...
  (-1).*t).*theta)+q14.*sin((1/2).*t.*theta))).*((-1).*csc((1/2).*theta) ...
  .^2.*(q01.*sin((1/2).*(1+(-1).*t).*theta)+q11.*sin((1/2).*t.*theta)).*( ...
  q02.*sin((1/2).*(1+(-1).*t).*theta)+q12.*sin((1/2).*t.*theta))+csc((1/2) ...
  .*theta).^2.*(q03.*sin((1/2).*(1+(-1).*t).*theta)+q13.*sin((1/2).*t.* ...
  theta)).*(q04.*sin((1/2).*(1+(-1).*t).*theta)+q14.*sin((1/2).*t.*theta)) ...
  )+(-4).*(2.*((-1/2).*q02.*theta.*cos((1/2).*(1+(-1).*t).*theta)+(1/2).* ...
  q12.*theta.*cos((1/2).*t.*theta)).*csc((1/2).*theta).^2.*(q02.*sin((1/2) ...
  .*(1+(-1).*t).*theta)+q12.*sin((1/2).*t.*theta))+2.*((-1/2).*q03.* ...
  theta.*cos((1/2).*(1+(-1).*t).*theta)+(1/2).*q13.*theta.*cos((1/2).*t.* ...
  theta)).*csc((1/2).*theta).^2.*(q03.*sin((1/2).*(1+(-1).*t).*theta)+ ...
  q13.*sin((1/2).*t.*theta))).*(1+(-2).*(csc((1/2).*theta).^2.*(q02.*sin(( ...
  1/2).*(1+(-1).*t).*theta)+q12.*sin((1/2).*t.*theta)).^2+csc((1/2).* ...
  theta).^2.*(q03.*sin((1/2).*(1+(-1).*t).*theta)+q13.*sin((1/2).*t.* ...
  theta)).^2))).*(4.*((-1).*csc((1/2).*theta).^2.*(q01.*sin((1/2).*(1+(-1) ...
  .*t).*theta)+q11.*sin((1/2).*t.*theta)).*(q02.*sin((1/2).*(1+(-1).*t).* ...
  theta)+q12.*sin((1/2).*t.*theta))+csc((1/2).*theta).^2.*(q03.*sin((1/2) ...
  .*(1+(-1).*t).*theta)+q13.*sin((1/2).*t.*theta)).*(q04.*sin((1/2).*(1+( ...
  -1).*t).*theta)+q14.*sin((1/2).*t.*theta))).^2+(1+(-2).*(csc((1/2).* ...
  theta).^2.*(q02.*sin((1/2).*(1+(-1).*t).*theta)+q12.*sin((1/2).*t.* ...
  theta)).^2+csc((1/2).*theta).^2.*(q03.*sin((1/2).*(1+(-1).*t).*theta)+ ...
  q13.*sin((1/2).*t.*theta)).^2)).^2).^(-1/2).*(4.*(csc((1/2).*theta).^2.* ...
  (q01.*sin((1/2).*(1+(-1).*t).*theta)+q11.*sin((1/2).*t.*theta)).*(q03.* ...
  sin((1/2).*(1+(-1).*t).*theta)+q13.*sin((1/2).*t.*theta))+csc((1/2).* ...
  theta).^2.*(q02.*sin((1/2).*(1+(-1).*t).*theta)+q12.*sin((1/2).*t.* ...
  theta)).*(q04.*sin((1/2).*(1+(-1).*t).*theta)+q14.*sin((1/2).*t.*theta)) ...
  ).^2+4.*((-1).*csc((1/2).*theta).^2.*(q01.*sin((1/2).*(1+(-1).*t).* ...
  theta)+q11.*sin((1/2).*t.*theta)).*(q02.*sin((1/2).*(1+(-1).*t).*theta)+ ...
  q12.*sin((1/2).*t.*theta))+csc((1/2).*theta).^2.*(q03.*sin((1/2).*(1+( ...
  -1).*t).*theta)+q13.*sin((1/2).*t.*theta)).*(q04.*sin((1/2).*(1+(-1).*t) ...
  .*theta)+q14.*sin((1/2).*t.*theta))).^2+(1+(-2).*(csc((1/2).*theta).^2.* ...
  (q02.*sin((1/2).*(1+(-1).*t).*theta)+q12.*sin((1/2).*t.*theta)).^2+csc(( ...
  1/2).*theta).^2.*(q03.*sin((1/2).*(1+(-1).*t).*theta)+q13.*sin((1/2).* ...
  t.*theta)).^2)).^2).^(-1/2).*((-1).*(csc((1/2).*theta).^2.*(q02.*sin(( ...
  1/2).*(1+(-1).*t).*theta)+q12.*sin((1/2).*t.*theta)).*(q03.*sin((1/2).*( ...
  1+(-1).*t).*theta)+q13.*sin((1/2).*t.*theta))+(-1).*csc((1/2).*theta) ...
  .^2.*(q01.*sin((1/2).*(1+(-1).*t).*theta)+q11.*sin((1/2).*t.*theta)).*( ...
  q04.*sin((1/2).*(1+(-1).*t).*theta)+q14.*sin((1/2).*t.*theta))).*(8.*((( ...
  -1/2).*q03.*theta.*cos((1/2).*(1+(-1).*t).*theta)+(1/2).*q13.*theta.* ...
  cos((1/2).*t.*theta)).*csc((1/2).*theta).^2.*(q01.*sin((1/2).*(1+(-1).* ...
  t).*theta)+q11.*sin((1/2).*t.*theta))+((-1/2).*q04.*theta.*cos((1/2).*( ...
  1+(-1).*t).*theta)+(1/2).*q14.*theta.*cos((1/2).*t.*theta)).*csc((1/2).* ...
  theta).^2.*(q02.*sin((1/2).*(1+(-1).*t).*theta)+q12.*sin((1/2).*t.* ...
  theta))+((-1/2).*q01.*theta.*cos((1/2).*(1+(-1).*t).*theta)+(1/2).*q11.* ...
  theta.*cos((1/2).*t.*theta)).*csc((1/2).*theta).^2.*(q03.*sin((1/2).*(1+ ...
  (-1).*t).*theta)+q13.*sin((1/2).*t.*theta))+((-1/2).*q02.*theta.*cos(( ...
  1/2).*(1+(-1).*t).*theta)+(1/2).*q12.*theta.*cos((1/2).*t.*theta)).*csc( ...
  (1/2).*theta).^2.*(q04.*sin((1/2).*(1+(-1).*t).*theta)+q14.*sin((1/2).* ...
  t.*theta))).*(csc((1/2).*theta).^2.*(q01.*sin((1/2).*(1+(-1).*t).*theta) ...
  +q11.*sin((1/2).*t.*theta)).*(q03.*sin((1/2).*(1+(-1).*t).*theta)+q13.* ...
  sin((1/2).*t.*theta))+csc((1/2).*theta).^2.*(q02.*sin((1/2).*(1+(-1).*t) ...
  .*theta)+q12.*sin((1/2).*t.*theta)).*(q04.*sin((1/2).*(1+(-1).*t).* ...
  theta)+q14.*sin((1/2).*t.*theta)))+8.*((-1).*((-1/2).*q02.*theta.*cos(( ...
  1/2).*(1+(-1).*t).*theta)+(1/2).*q12.*theta.*cos((1/2).*t.*theta)).*csc( ...
  (1/2).*theta).^2.*(q01.*sin((1/2).*(1+(-1).*t).*theta)+q11.*sin((1/2).* ...
  t.*theta))+(-1).*((-1/2).*q01.*theta.*cos((1/2).*(1+(-1).*t).*theta)+( ...
  1/2).*q11.*theta.*cos((1/2).*t.*theta)).*csc((1/2).*theta).^2.*(q02.* ...
  sin((1/2).*(1+(-1).*t).*theta)+q12.*sin((1/2).*t.*theta))+((-1/2).*q04.* ...
  theta.*cos((1/2).*(1+(-1).*t).*theta)+(1/2).*q14.*theta.*cos((1/2).*t.* ...
  theta)).*csc((1/2).*theta).^2.*(q03.*sin((1/2).*(1+(-1).*t).*theta)+ ...
  q13.*sin((1/2).*t.*theta))+((-1/2).*q03.*theta.*cos((1/2).*(1+(-1).*t).* ...
  theta)+(1/2).*q13.*theta.*cos((1/2).*t.*theta)).*csc((1/2).*theta).^2.*( ...
  q04.*sin((1/2).*(1+(-1).*t).*theta)+q14.*sin((1/2).*t.*theta))).*((-1).* ...
  csc((1/2).*theta).^2.*(q01.*sin((1/2).*(1+(-1).*t).*theta)+q11.*sin(( ...
